simulink model "Simulation"  (R2016a)
(part 16 of 30)

C= [ thetadot4*(cos(theta5)*(((sin(theta6)*(cos(theta5)*(sin(theta4)*(thetadot2 + thetadot3) + thetadot1*cos(theta2 + theta3)*cos(theta4)) - sin(theta5)*(thetadot4 + thetadot1*sin(theta2 + theta3))))/10 + (cos(theta6)*(thetadot5 + cos(theta4)*(thetadot2 + thetadot3) - thetadot1*cos(theta2 + theta3)*sin(theta4)))/10)*(cos(theta2)*cos(theta6)*sin(theta3)*sin(theta5) - cos(theta2)*cos(theta3)*sin(theta4)*sin(theta6) + cos(theta3)*cos(theta6)*sin(theta2)*sin(theta5) + sin(theta2)*sin(theta3)*sin(theta4)*sin(theta6) - cos(theta2)*cos(theta3)*cos(theta4)*cos(theta5)*cos(theta6) + cos(theta4)*cos(theta5)*cos(theta6)*sin(theta2)*sin(theta3)) + ((sin(theta6)*(thetadot5 + cos(theta4)*(thetadot2 + thetadot3) - thetadot1*cos(theta2 + theta3)*sin(theta4)))/10 - (cos(theta6)*(cos(theta5)*(sin(theta4)*(thetadot2 + thetadot3) + thetadot1*cos(theta2 + theta3)*cos(theta4)) - sin(theta5)*(thetadot4 + thetadot1*sin(theta2 + theta3))))/10)*(cos(theta2)*cos(theta3)*cos(theta6)*sin(theta4) - cos(theta6)*sin(theta2)*sin(theta3)*sin(theta4) + cos(theta2)*sin(theta3)*sin(theta5)*sin(theta6) + cos(theta3)*sin(theta2)*sin(theta5)*sin(theta6) - cos(theta2)*cos(theta3)*cos(theta4)*cos(theta5)*sin(theta6) + cos(theta4)*cos(theta5)*sin(theta2)*sin(theta3)*sin(theta6))) + sin(theta5)*((thetadot5/10 + (cos(theta4)*(thetadot2 + thetadot3))/10 - (thetadot1*cos(theta2 + theta3)*sin(theta4))/10)*(cos(theta2)*cos(theta5)*sin(theta3) + cos(theta3)*cos(theta5)*sin(theta2) + cos(theta2)*cos(theta3)*cos(theta4)*sin(theta5) - cos(theta4)*sin(theta2)*sin(theta3)*sin(theta5)) - (thetadot6*sin(theta6)*(cos(theta2)*cos(theta6)*sin(theta3)*sin(theta5) - cos(theta2)*cos(theta3)*sin(theta4)*sin(theta6) + cos(theta3)*cos(theta6)*sin(theta2)*sin(theta5) + sin(theta2)*sin(theta3)*sin(theta4)*sin(theta6) - cos(theta2)*cos(theta3)*cos(theta4)*cos(theta5)*cos(theta6) + cos(theta4)*cos(theta5)*cos(theta6)*sin(theta2)*sin(theta3)))/10 + (2*thetadot6*cos(theta6)*((cos(theta2)*sin(theta4)*sin(theta5))/5 + (2*sin(theta2)*sin(theta3)*sin(theta4))/5 - (2*cos(theta2)*cos(theta3)*sin(theta4))/5 + (2*cos(theta2)*cos(theta3)*cos(theta6)*sin(theta4))/5 + (2*cos(theta2)*cos(theta3)*sin(theta4)*sin(theta5))/5 - (2*cos(theta6)*sin(theta2)*sin(theta3)*sin(theta4))/5 + (2*cos(theta2)*sin(theta3)*sin(theta5)*sin(theta6))/5 + (2*cos(theta3)*sin(theta2)*sin(theta5)*sin(theta6))/5 - (2*sin(theta2)*sin(theta3)*sin(theta4)*sin(theta5))/5 - (2*cos(theta2)*cos(theta3)*cos(theta4)*cos(theta5)*sin(theta6))/5 + (2*cos(theta4)*cos(theta5)*sin(theta2)*sin(theta3)*sin(theta6))/5))/5 + (thetadot6*cos(theta6)*(cos(theta2)*cos(theta3)*cos(theta6)*sin(theta4) - cos(theta6)*sin(theta2)*sin(theta3)*sin(theta4) + cos(theta2)*sin(theta3)*sin(theta5)*sin(theta6) + cos(theta3)*sin(theta2)*sin(theta5)*sin(theta6) - cos(theta2)*cos(theta3)*cos(theta4)*cos(theta5)*sin(theta6) + cos(theta4)*cos(theta5)*sin(theta2)*sin(theta3)*sin(theta6)))/10 + cos(theta2 + theta3)*sin(theta4)*((sin(theta5)*(sin(theta4)*(thetadot2 + thetadot3) + thetadot1*cos(theta2 + theta3)*cos(theta4)))/10 + (cos(theta5)*(thetadot4 + thetadot1*sin(theta2 + theta3)))/10)) + cos(theta5)*(((2*thetadot6)/5 + thetadot6*((2*cos(theta6))/5 - 2/5))*((cos(theta2)*cos(theta5)*cos(theta6)*sin(theta4))/5 - (2*cos(theta2)*cos(theta3)*cos(theta4)*sin(theta6))/5 - (cos(theta2)*cos(theta4)*sin(theta6))/5 + (2*cos(theta2)*cos(theta5)*sin(theta3)*sin(theta6))/5 + (2*cos(theta3)*cos(theta5)*sin(theta2)*sin(theta6))/5 + (2*cos(theta4)*sin(theta2)*sin(theta3)*sin(theta6))/5 + (2*cos(theta2)*cos(theta3)*cos(theta5)*cos(theta6)*sin(theta4))/5 + (2*cos(theta2)*cos(theta3)*cos(theta4)*sin(theta5)*sin(theta6))/5 - (2*cos(theta5)*cos(theta6)*sin(theta2)*sin(theta3)*sin(theta4))/5 - (2*cos(theta4)*sin(theta2)*sin(theta3)*sin(theta5)*sin(theta6))/5) - (thetadot5/10 + (cos(theta4)*(thetadot2 + thetadot3))/10 - (thetadot1*cos(theta2 + theta3)*sin(theta4))/10)*(cos(theta2)*sin(theta3)*sin(theta5) + cos(theta3)*sin(theta2)*sin(theta5) - cos(theta2)*cos(theta3)*cos(theta4)*cos(theta5) + cos(theta4)*cos(theta5)*sin(theta2)*sin(theta3)) + cos(theta2 + theta3)*sin(theta4)*((cos(theta5)*(sin(theta4)*(thetadot2 + thetadot3) + thetadot1*cos(theta2 + theta3)*cos(theta4)))/10 - (sin(theta5)*(thetadot4 + thetadot1*sin(theta2 + theta3)))/10) + (2*thetadot6*sin(theta6)*((cos(theta2)*cos(theta4)*cos(theta6))/5 + (2*cos(theta2)*cos(theta5)*sin(theta3))/5 + (2*cos(theta3)*cos(theta5)*sin(theta2))/5 + (2*cos(theta2)*cos(theta3)*cos(theta4)*cos(theta6))/5 + (2*cos(theta2)*cos(theta3)*cos(theta4)*sin(theta5))/5 - (2*cos(theta2)*cos(theta5)*cos(theta6)*sin(theta3))/5 - (2*cos(theta3)*cos(theta5)*cos(theta6)*sin(theta2))/5 - (2*cos(theta4)*cos(theta6)*sin(theta2)*sin(theta3))/5 + (cos(theta2)*cos(theta5)*sin(theta4)*sin(theta6))/5 - (2*cos(theta4)*sin(theta2)*sin(theta3)*sin(theta5))/5 - (2*cos(theta2)*cos(theta3)*cos(theta4)*cos(theta6)*sin(theta5))/5 + (2*cos(theta2)*cos(theta3)*cos(theta5)*sin(theta4)*sin(theta6))/5 + (2*cos(theta4)*cos(theta6)*sin(theta2)*sin(theta3)*sin(theta5))/5 - (2*cos(theta5)*sin(theta2)*sin(theta3)*sin(theta4)*sin(theta6))/5))/5) + sin(theta5)*sin(theta6)*((thetadot6/10 + (sin(theta5)*(sin(theta4)*(thetadot2 + thetadot3) + thetadot1*cos(theta2 + theta3)*cos(theta4)))/10 + (cos(theta5)*(thetadot4 + thetadot1*sin(theta2 + theta3)))/10)*(cos(theta2)*cos(theta6)*sin(theta3)*sin(theta5) - cos(theta2)*cos(theta3)*sin(theta4)*sin(theta6) + cos(theta3)*cos(theta6)*sin(theta2)*sin(theta5) + sin(theta2)*sin(theta3)*sin(theta4)*sin(theta6) - cos(theta2)*cos(theta3)*cos(theta4)*cos(theta5)*cos(theta6) + cos(theta4)*cos(theta5)*cos(theta6)*sin(theta2)*sin(theta3)) - ((sin(theta6)*(thetadot5 + cos(theta4)*(thetadot2 + thetadot3) - thetadot1*cos(theta2 + theta3)*sin(theta4)))/10 - (cos(theta6)*(cos(theta5)*(sin(theta4)*(thetadot2 + thetadot3) + thetadot1*cos(theta2 + theta3)*cos(theta4)) - sin(theta5)*(thetadot4 + thetadot1*sin(theta2 + theta3))))/10)*(cos(theta2)*cos(theta5)*sin(theta3) + cos(theta3)*cos(theta5)*sin(theta2) + cos(theta2)*cos(theta3)*cos(theta4)*sin(theta5) - cos(theta4)*sin(theta2)*sin(theta3)*sin(theta5))) + cos(theta2 + theta3)*cos(theta4)*((cos(theta4)*(thetadot2 + thetadot3))/10 - (thetadot1*cos(theta2 + theta3)*sin(theta4))/10) - cos(theta6)*sin(theta5)*((thetadot6/10 + (sin(theta5)*(sin(theta4)*(thetadot2 + thetadot3) + thetadot1*cos(theta2 + theta3)*cos(theta4)))/10 + (cos(theta5)*(thetadot4 + thetadot1*sin(theta2 + theta3)))/10)*(cos(theta2)*cos(theta3)*cos(theta6)*sin(theta4) - cos(theta6)*sin(theta2)*sin(theta3)*sin(theta4) + cos(theta2)*sin(theta3)*sin(theta5)*sin(theta6) + cos(theta3)*sin(theta2)*sin(theta5)*sin(theta6) - cos(theta2)*cos(theta3)*cos(theta4)*cos(theta5)*sin(theta6) + cos(theta4)*cos(theta5)*sin(theta2)*sin(theta3)*sin(theta6)) + ((sin(theta6)*(cos(theta5)*(sin(theta4)*(thetadot2 + thetadot3) + thetadot1*cos(theta2 + theta3)*cos(theta4)) - sin(theta5)*(thetadot4 + thetadot1*sin(theta2 + theta3))))/10 + (cos(theta6)*(thetadot5 + cos(theta4)*(thetadot2 + thetadot3) - thetadot1*cos(theta2 + theta3)*sin(theta4)))/10)*(cos(theta2)*cos(theta5)*sin(theta3) + cos(theta3)*cos(theta5)*sin(theta2) + cos(theta2)*cos(theta3)*cos(theta4)*sin(theta5) - cos(theta4)*sin(theta2)*sin(theta3)*sin(theta5))) + cos(theta2 + theta3)*sin(theta4)*((sin(theta4)*(thetadot2 + thetadot3))/10 + (thetadot1*cos(theta2 + theta3)*cos(theta4))/10) - (2*cos(theta5)*sin(theta6)*((thetadot6 + sin(theta5)*(sin(theta4)*(thetadot2 + thetadot3) + thetadot1*cos(theta2 + theta3)*cos(theta4)) + cos(theta5)*(thetadot4 + thetadot1*sin(theta2 + theta3)))*((cos(theta2)*cos(theta4)*cos(theta6))/5 + (2*cos(theta2)*cos(theta5)*sin(theta3))/5 + (2*cos(theta3)*cos(theta5)*sin(theta2))/5 + (2*cos(theta2)*cos(theta3)*cos(theta4)*cos(theta6))/5 + (2*cos(theta2)*cos(theta3)*cos(theta4)*sin(theta5))/5 - (2*cos(theta2)*cos(theta5)*cos(theta6)*sin(theta3))/5 - (2*cos(theta3)*cos(theta5)*cos(theta6)*sin(theta2))/5 - (2*cos(theta4)*cos(theta6)*sin(theta2)*sin(theta3))/5 + (cos(theta2)*cos(theta5)*sin(theta4)*sin(theta6))/5 - (2*cos(theta4)*sin(theta2)*sin(theta3)*sin(theta5))/5 - (2*cos(theta2)*cos(theta3)*cos(theta4)*cos(theta6)*sin(theta5))/5 + (2*cos(theta2)*cos(theta3)*cos(theta5)*sin(theta4)*sin(theta6))/5 + (2*cos(theta4)*cos(theta6)*sin(theta2)*sin(theta3)*sin(theta5))/5 - (2*cos(theta5)*sin(theta2)*sin(theta3)*sin(theta4)*sin(theta6))/5) - (cos(theta2)*cos(theta5)*sin(theta3) + cos(theta3)*cos(theta5)*sin(theta2) + cos(theta2)*cos(theta3)*cos(theta4)*sin(theta5) - cos(theta4)*sin(theta2)*sin(theta3)*sin(theta5))*((2*thetadot6)/5 - (sin(theta5)*(thetadot2*sin(theta4) + thetadot3*sin(theta4) + thetadot1*cos(theta2 + theta3)*cos(theta4)) + cos(theta5)*(thetadot4 + thetadot1*sin(theta2 + theta3)))*((2*cos(theta6))/5 - 2/5) - (sin(theta6)*(2*thetadot2*cos(theta4)*cos(theta5) + 2*thetadot3*cos(theta4)*cos(theta5) - thetadot2*sin(theta3)*sin(theta5) + thetadot2*cos(theta3)*cos(theta4)*cos(theta5) - thetadot1*cos(theta2)*cos(theta5)*sin(theta4) - 2*thetadot1*cos(theta2)*cos(theta3)*cos(theta5)*sin(theta4) + 2*thetadot1*cos(theta5)*sin(theta2)*sin(theta3)*sin(theta4)))/5 + (cos(theta6)*(2*thetadot2*sin(theta4) + 2*thetadot3*sin(theta4) + thetadot1*cos(theta2)*cos(theta4) + thetadot2*cos(theta3)*sin(theta4) + 2*thetadot1*cos(theta2)*cos(theta3)*cos(theta4) - 2*thetadot1*cos(theta4)*sin(theta2)*sin(theta3)))/5) - (sin(theta6)*(cos(theta5)*(sin(theta4)*(thetadot2 + thetadot3) + thetadot1*cos(theta2 + theta3)*cos(theta4)) - sin(theta5)*(thetadot4 + thetadot1*sin(theta2 + theta3))) + cos(theta6)*(thetadot5 + cos(theta4)*(thetadot2 + thetadot3) - thetadot1*cos(theta2 + theta3)*sin(theta4)))*((cos(theta2)*sin(theta4)*sin(theta5))/5 + (2*sin(theta2)*sin(theta3)*sin(theta4))/5 - (2*cos(theta2)*cos(theta3)*sin(theta4))/5 + (2*cos(theta2)*cos(theta3)*cos(theta6)*sin(theta4))/5 + (2*cos(theta2)*cos(theta3)*sin(theta4)*sin(theta5))/5 - (2*cos(theta6)*sin(theta2)*sin(theta3)*sin(theta4))/5 + (2*cos(theta2)*sin(theta3)*sin(theta5)*sin(theta6))/5 + (2*cos(theta3)*sin(theta2)*sin(theta5)*sin(theta6))/5 - (2*sin(theta2)*sin(theta3)*sin(theta4)*sin(theta5))/5 - (2*cos(theta2)*cos(theta3)*cos(theta4)*cos(theta5)*sin(theta6))/5 + (2*cos(theta4)*cos(theta5)*sin(theta2)*sin(theta3)*sin(theta6))/5) + ((sin(theta5)*(thetadot2*cos(theta4) + thetadot3*cos(theta4) - thetadot1*cos(theta2 + theta3)*sin(theta4)))/5 + sin(theta5)*((thetadot2*cos(theta4))/5 + (thetadot3*cos(theta4))/5 - (thetadot1*cos(theta2 + theta3)*sin(theta4))/5 + (thetadot2*cos(theta3)*cos(theta4))/5 - (thetadot1*cos(theta2)*sin(theta4))/5) + ((2*cos(theta6))/5 - 2/5)*(thetadot5 + thetadot2*cos(theta4) + thetadot3*cos(theta4) - thetadot1*cos(theta2 + theta3)*sin(theta4)) + (2*sin(theta6)*(cos(theta5)*(thetadot2*sin(theta4) + thetadot3*sin(theta4) + thetadot1*cos(theta2 + theta3)*cos(theta4)) - sin(theta5)*(thetadot4 + thetadot1*sin(theta2 + theta3))))/5 + (thetadot2*cos(theta5)*sin(theta3))/5)*(cos(theta2)*cos(theta3)*cos(theta6)*sin(theta4) - cos(theta6)*sin(theta2)*sin(theta3)*sin(theta4) + cos(theta2)*sin(theta3)*sin(theta5)*sin(theta6) + cos(theta3)*sin(theta2)*sin(theta5)*sin(theta6) - cos(theta2)*cos(theta3)*cos(theta4)*cos(theta5)*sin(theta6) + cos(theta4)*cos(theta5)*sin(theta2)*sin(theta3)*sin(theta6))))/5 - (2*cos(theta5)*(cos(theta6) - 1)*(((sin(theta6)*(2*thetadot2*sin(theta4) + 2*thetadot3*sin(theta4) + thetadot1*cos(theta2)*cos(theta4) + thetadot2*cos(theta3)*sin(theta4) + 2*thetadot1*cos(theta2)*cos(theta3)*cos(theta4) - 2*thetadot1*cos(theta4)*sin(theta2)*sin(theta3)))/5 + (cos(theta6)*(2*thetadot2*cos(theta4)*cos(theta5) + 2*thetadot3*cos(theta4)*cos(theta5) - thetadot2*sin(theta3)*sin(theta5) + thetadot2*cos(theta3)*cos(theta4)*cos(theta5) - thetadot1*cos(theta2)*cos(theta5)*sin(theta4) - 2*thetadot1*cos(theta2)*cos(theta3)*cos(theta5)*sin(theta4) + 2*thetadot1*cos(theta5)*sin(theta2)*sin(theta3)*sin(theta4)))/5 - (2*sin(theta6)*(sin(theta5)*(thetadot2*sin(theta4) + thetadot3*sin(theta4) + thetadot1*cos(theta2 + theta3)*cos(theta4)) + cos(theta5)*(thetadot4 + thetadot1*sin(theta2 + theta3))))/5)*(cos(theta2)*cos(theta5)*sin(theta3) + cos(theta3)*cos(theta5)*sin(theta2) + cos(theta2)*cos(theta3)*cos(theta4)*sin(theta5) - cos(theta4)*sin(theta2)*sin(theta3)*sin(theta5)) + ((sin(theta5)*(thetadot2*cos(theta4) + thetadot3*cos(theta4) - thetadot1*cos(theta2 + theta3)*sin(theta4)))/5 + sin(theta5)*((thetadot2*cos(theta4))/5 + (thetadot3*cos(theta4))/5 - (thetadot1*cos(theta2 + theta3)*sin(theta4))/5 + (thetadot2*cos(theta3)*cos(theta4))/5 - (thetadot1*cos(theta2)*sin(theta4))/5) + ((2*cos(theta6))/5 - 2/5)*(thetadot5 + thetadot2*cos(theta4) + thetadot3*cos(theta4) - thetadot1*cos(theta2 + theta3)*sin(theta4)) + (2*sin(theta6)*(cos(theta5)*(thetadot2*sin(theta4) + thetadot3*sin(theta4) + thetadot1*cos(theta2 + theta3)*cos(theta4)) - sin(theta5)*(thetadot4 + thetadot1*sin(theta2 + theta3))))/5 + (thetadot2*cos(theta5)*sin(theta3))/5)*(cos(theta2)*cos(theta6)*sin(theta3)*sin(theta5) - cos(theta2)*cos(theta3)*sin(theta4)*sin(theta6) + cos(theta3)*cos(theta6)*sin(theta2)*sin(theta5) + sin(theta2)*sin(theta3)*sin(theta4)*sin(theta6) - cos(theta2)*cos(theta3)*cos(theta4)*cos(theta5)*cos(theta6) + cos(theta4)*cos(theta5)*cos(theta6)*sin(theta2)*sin(theta3)) + (sin(theta6)*(thetadot5 + cos(theta4)*(thetadot2 + thetadot3) - thetadot1*cos(theta2 + theta3)*sin(theta4)) - cos(theta6)*(cos(theta5)*(sin(theta4)*(thetadot2 + thetadot3) + thetadot1*cos(theta2 + theta3)*cos(theta4)) - sin(theta5)*(thetadot4 + thetadot1*sin(theta2 + theta3))))*((cos(theta2)*sin(theta4)*sin(theta5))/5 + (2*sin(theta2)*sin(theta3)*sin(theta4))/5 - (2*cos(theta2)*cos(theta3)*sin(theta4))/5 + (2*cos(theta2)*cos(theta3)*cos(theta6)*sin(theta4))/5 + (2*cos(theta2)*cos(theta3)*sin(theta4)*sin(theta5))/5 - (2*cos(theta6)*sin(theta2)*sin(theta3)*sin(theta4))/5 + (2*cos(theta2)*sin(theta3)*sin(theta5)*sin(theta6))/5 + (2*cos(theta3)*sin(theta2)*sin(theta5)*sin(theta6))/5 - (2*sin(theta2)*sin(theta3)*sin(theta4)*sin(theta5))/5 - (2*cos(theta2)*cos(theta3)*cos(theta4)*cos(theta5)*sin(theta6))/5 + (2*cos(theta4)*cos(theta5)*sin(theta2)*sin(theta3)*sin(theta6))/5) + (thetadot6 + sin(theta5)*(sin(theta4)*(thetadot2 + thetadot3) + thetadot1*cos(theta2 + theta3)*cos(theta4)) + cos(theta5)*(thetadot4 + thetadot1*sin(theta2 + theta3)))*((cos(theta2)*cos(theta5)*cos(theta6)*sin(theta4))/5 - (2*cos(theta2)*cos(theta3)*cos(theta4)*sin(theta6))/5 - (cos(theta2)*cos(theta4)*sin(theta6))/5 + (2*cos(theta2)*cos(theta5)*sin(theta3)*sin(theta6))/5 + (2*cos(theta3)*cos(theta5)*sin(theta2)*sin(theta6))/5 + (2*cos(theta4)*sin(theta2)*sin(theta3)*sin(theta6))/5 + (2*cos(theta2)*cos(theta3)*cos(theta5)*cos(theta6)*sin(theta4))/5 + (2*cos(theta2)*cos(theta3)*cos(theta4)*sin(theta5)*sin(theta6))/5 - (2*cos(theta5)*cos(theta6)*sin(theta2)*sin(theta3)*sin(theta4))/5 - (2*cos(theta4)*sin(theta2)*sin(theta3)*sin(theta5)*sin(theta6))/5)))/5 + (thetadot5*cos(theta5)*(cos(theta2)*sin(theta3)*sin(theta5) + cos(theta3)*sin(theta2)*sin(theta5) - cos(theta2)*cos(theta3)*cos(theta4)*cos(theta5) + cos(theta4)*cos(theta5)*sin(theta2)*sin(theta3)))/10 - (2*sin(theta5)*sin(theta6)*((sin(theta6)*(cos(theta5)*(sin(theta4)*(thetadot2 + thetadot3) + thetadot1*cos(theta2 + theta3)*cos(theta4)) - sin(theta5)*(thetadot4 + thetadot1*sin(theta2 + theta3))) + cos(theta6)*(thetadot5 + cos(theta4)*(thetadot2 + thetadot3) - thetadot1*cos(theta2 + theta3)*sin(theta4)))*((cos(theta2)*cos(theta5)*cos(theta6)*sin(theta4))/5 - (2*cos(theta2)*cos(theta3)*cos(theta4)*sin(theta6))/5 - (cos(theta2)*cos(theta4)*sin(theta6))/5 + (2*cos(theta2)*cos(theta5)*sin(theta3)*sin(theta6))/5 + (2*cos(theta3)*cos(theta5)*sin(theta2)*sin(theta6))/5 + (2*cos(theta4)*sin(theta2)*sin(theta3)*sin(theta6))/5 + (2*cos(theta2)*cos(theta3)*cos(theta5)*cos(theta6)*sin(theta4))/5 + (2*cos(theta2)*cos(theta3)*cos(theta4)*sin(theta5)*sin(theta6))/5 - (2*cos(theta5)*cos(theta6)*sin(theta2)*sin(theta3)*sin(theta4))/5 - (2*cos(theta4)*sin(theta2)*sin(theta3)*sin(theta5)*sin(theta6))/5) + (sin(theta6)*(thetadot5 + cos(theta4)*(thetadot2 + thetadot3) - thetadot1*cos(theta2 + theta3)*sin(theta4)) - cos(theta6)*(cos(theta5)*(sin(theta4)*(thetadot2 + thetadot3) + thetadot1*cos(theta2 + theta3)*cos(theta4)) - sin(theta5)*(thetadot4 + thetadot1*sin(theta2 + theta3))))*((cos(theta2)*cos(theta4)*cos(theta6))/5 + (2*cos(theta2)*cos(theta5)*sin(theta3))/5 + (2*cos(theta3)*cos(theta5)*sin(theta2))/5 + (2*cos(theta2)*cos(theta3)*cos(theta4)*cos(theta6))/5 + (2*cos(theta2)*cos(theta3)*cos(theta4)*sin(theta5))/5 - (2*cos(theta2)*cos(theta5)*cos(theta6)*sin(theta3))/5 - (2*cos(theta3)*cos(theta5)*cos(theta6)*sin(theta2))/5 - (2*cos(theta4)*cos(theta6)*sin(theta2)*sin(theta3))/5 + (cos(theta2)*cos(theta5)*sin(theta4)*sin(theta6))/5 - (2*cos(theta4)*sin(theta2)*sin(theta3)*sin(theta5))/5 - (2*cos(theta2)*cos(theta3)*cos(theta4)*cos(theta6)*sin(theta5))/5 + (2*cos(theta2)*cos(theta3)*cos(theta5)*sin(theta4)*sin(theta6))/5 + (2*cos(theta4)*cos(theta6)*sin(theta2)*sin(theta3)*sin(theta5))/5 - (2*cos(theta5)*sin(theta2)*sin(theta3)*sin(theta4)*sin(theta6))/5) - ((sin(theta6)*(2*thetadot2*sin(theta4) + 2*thetadot3*sin(theta4) + thetadot1*cos(theta2)*cos(theta4) + thetadot2*cos(theta3)*sin(theta4) + 2*thetadot1*cos(theta2)*cos(theta3)*cos(theta4) - 2*thetadot1*cos(theta4)*sin(theta2)*sin(theta3)))/5 + (cos(theta6)*(2*thetadot2*cos(theta4)*cos(theta5) + 2*thetadot3*cos(theta4)*cos(theta5) - thetadot2*sin(theta3)*sin(theta5) + thetadot2*cos(theta3)*cos(theta4)*cos(theta5) - thetadot1*cos(theta2)*cos(theta5)*sin(theta4) - 2*thetadot1*cos(theta2)*cos(theta3)*cos(theta5)*sin(theta4) + 2*thetadot1*cos(theta5)*sin(theta2)*sin(theta3)*sin(theta4)))/5 - (2*sin(theta6)*(sin(theta5)*(thetadot2*sin(theta4) + thetadot3*sin(theta4) + thetadot1*cos(theta2 + theta3)*cos(theta4)) + cos(theta5)*(thetadot4 + thetadot1*sin(theta2 + theta3))))/5)*(cos(theta2)*cos(theta3)*cos(theta6)*sin(theta4) - cos(theta6)*sin(theta2)*sin(theta3)*sin(theta4) + cos(theta2)*sin(theta3)*sin(theta5)*sin(theta6) + cos(theta3)*sin(theta2)*sin(theta5)*sin(theta6) - cos(theta2)*cos(theta3)*cos(theta4)*cos(theta5)*sin(theta6) + cos(theta4)*cos(theta5)*sin(theta2)*sin(theta3)*sin(theta6)) - ((2*thetadot6)/5 - (sin(theta5)*(thetadot2*sin(theta4) + thetadot3*sin(theta4) + thetadot1*cos(theta2 + theta3)*cos(theta4)) + cos(theta5)*(thetadot4 + thetadot1*sin(theta2 + theta3)))*((2*cos(theta6))/5 - 2/5) - (sin(theta6)*(2*thetadot2*cos(theta4)*cos(theta5) + 2*thetadot3*cos(theta4)*cos(theta5) - thetadot2*sin(theta3)*sin(theta5) + thetadot2*cos(theta3)*cos(theta4)*cos(theta5) - thetadot1*cos(theta2)*cos(theta5)*sin(theta4) - 2*thetadot1*cos(theta2)*cos(theta3)*cos(theta5)*sin(theta4) + 2*thetadot1*cos(theta5)*sin(theta2)*sin(theta3)*sin(theta4)))/5 + (cos(theta6)*(2*thetadot2*sin(theta4) + 2*thetadot3*sin(theta4) + thetadot1*cos(theta2)*cos(theta4) + thetadot2*cos(theta3)*sin(theta4) + 2*thetadot1*cos(theta2)*cos(theta3)*cos(theta4) - 2*thetadot1*cos(theta4)*sin(theta2)*sin(theta3)))/5)*(cos(theta2)*cos(theta6)*sin(theta3)*sin(theta5) - cos(theta2)*cos(theta3)*sin(theta4)*sin(theta6) + cos(theta3)*cos(theta6)*sin(theta2)*sin(theta5) + sin(theta2)*sin(theta3)*sin(theta4)*sin(theta6) - cos(theta2)*cos(theta3)*cos(theta4)*cos(theta5)*cos(theta6) + cos(theta4)*cos(theta5)*cos(theta6)*sin(theta2)*sin(theta3))))/5 - (thetadot5*sin(theta5)*(cos(theta2)*cos(theta5)*sin(theta3) + cos(theta3)*cos(theta5)*sin(theta2) + cos(theta2)*cos(theta3)*cos(theta4)*sin(theta5) - cos(theta4)*sin(theta2)*sin(theta3)*sin(theta5)))/5 - (2*thetadot5*sin(theta5)*sin(theta6)*((cos(theta2)*cos(theta5)*cos(theta6)*sin(theta4))/5 - (2*cos(theta2)*cos(theta3)*cos(theta4)*sin(theta6))/5 - (cos(theta2)*cos(theta4)*sin(theta6))/5 + (2*cos(theta2)*cos(theta5)*sin(theta3)*sin(theta6))/5 + (2*cos(theta3)*cos(theta5)*sin(theta2)*sin(theta6))/5 + (2*cos(theta4)*sin(theta2)*sin(theta3)*sin(theta6))/5 + (2*cos(theta2)*cos(theta3)*cos(theta5)*cos(theta6)*sin(theta4))/5 + (2*cos(theta2)*cos(theta3)*cos(theta4)*sin(theta5)*sin(theta6))/5 - (2*cos(theta5)*cos(theta6)*sin(theta2)*sin(theta3)*sin(theta4))/5 - (2*cos(theta4)*sin(theta2)*sin(theta3)*sin(theta5)*sin(theta6))/5))/5 + thetadot5*sin(theta5)*((2*cos(theta6))/5 - 2/5)*((cos(theta2)*cos(theta4)*cos(theta6))/5 + (2*cos(theta2)*cos(theta5)*sin(theta3))/5 + (2*cos(theta3)*cos(theta5)*sin(theta2))/5 + (2*cos(theta2)*cos(theta3)*cos(theta4)*cos(theta6))/5 + (2*cos(theta2)*cos(theta3)*cos(theta4)*sin(theta5))/5 - (2*cos(theta2)*cos(theta5)*cos(theta6)*sin(theta3))/5 - (2*cos(theta3)*cos(theta5)*cos(theta6)*sin(theta2))/5 - (2*cos(theta4)*cos(theta6)*sin(theta2)*sin(theta3))/5 + (cos(theta2)*cos(theta5)*sin(theta4)*sin(theta6))/5 - (2*cos(theta4)*sin(theta2)*sin(theta3)*sin(theta5))/5 - (2*cos(theta2)*cos(theta3)*cos(theta4)*cos(theta6)*sin(theta5))/5 + (2*cos(theta2)*cos(theta3)*cos(theta5)*sin(theta4)*sin(theta6))/5 + (2*cos(theta4)*cos(theta6)*sin(theta2)*sin(theta3)*sin(theta5))/5 - (2*cos(theta5)*sin(theta2)*sin(theta3)*sin(theta4)*sin(theta6))/5) + (thetadot5*cos(theta5)*cos(theta6)*(cos(theta2)*cos(theta6)*sin(theta3)*sin(theta5) - cos(theta2)*cos(theta3)*sin(theta4)*sin(theta6) + cos(theta3)*cos(theta6)*sin(theta2)*sin(theta5) + sin(theta2)*sin(theta3)*sin(theta4)*sin(theta6) - cos(theta2)*cos(theta3)*cos(theta4)*cos(theta5)*cos(theta6) + cos(theta4)*cos(theta5)*cos(theta6)*sin(theta2)*sin(theta3)))/10 + (2*thetadot5*cos(theta5)*sin(theta6)*((cos(theta2)*sin(theta4)*sin(theta5))/5 + (2*sin(theta2)*sin(theta3)*sin(theta4))/5 - (2*cos(theta2)*cos(theta3)*sin(theta4))/5 + (2*cos(theta2)*cos(theta3)*cos(theta6)*sin(theta4))/5 + (2*cos(theta2)*cos(theta3)*sin(theta4)*sin(theta5))/5 - (2*cos(theta6)*sin(theta2)*sin(theta3)*sin(theta4))/5 + (2*cos(theta2)*sin(theta3)*sin(theta5)*sin(theta6))/5 + (2*cos(theta3)*sin(theta2)*sin(theta5)*sin(theta6))/5 - (2*sin(theta2)*sin(theta3)*sin(theta4)*sin(theta5))/5 - (2*cos(theta2)*cos(theta3)*cos(theta4)*cos(theta5)*sin(theta6))/5 + (2*cos(theta4)*cos(theta5)*sin(theta2)*sin(theta3)*sin(theta6))/5))/5 + (thetadot5*cos(theta5)*sin(theta6)*(cos(theta2)*cos(theta3)*cos(theta6)*sin(theta4) - cos(theta6)*sin(theta2)*sin(theta3)*sin(theta4) + cos(theta2)*sin(theta3)*sin(theta5)*sin(theta6) + cos(theta3)*sin(theta2)*sin(theta5)*sin(theta6) - cos(theta2)*cos(theta3)*cos(theta4)*cos(theta5)*sin(theta6) + cos(theta4)*cos(theta5)*sin(theta2)*sin(theta3)*sin(theta6)))/10) - thetadot1*(((thetadot6 + sin(theta5)*(sin(theta4)*(thetadot2 + thetadot3) + thetadot1*cos(theta2 + theta3)*cos(theta4)) + cos(theta5)*(thetadot4 + thetadot1*sin(theta2 + theta3)))*((cos(theta2)*cos(theta4)*cos(theta6))/5 + (2*cos(theta2)*cos(theta5)*sin(theta3))/5 + (2*cos(theta3)*cos(theta5)*sin(theta2))/5 + (2*cos(theta2)*cos(theta3)*cos(theta4)*cos(theta6))/5 + (2*cos(theta2)*cos(theta3)*cos(theta4)*sin(theta5))/5 - (2*cos(theta2)*cos(theta5)*cos(theta6)*sin(theta3))/5 - (2*cos(theta3)*cos(theta5)*cos(theta6)*sin(theta2))/5 - (2*cos(theta4)*cos(theta6)*sin(theta2)*sin(theta3))/5 + (cos(theta2)*cos(theta5)*sin(theta4)*sin(theta6))/5 - (2*cos(theta4)*sin(theta2)*sin(theta3)*sin(theta5))/5 - (2*cos(theta2)*cos(theta3)*cos(theta4)*cos(theta6)*sin(theta5))/5 + (2*cos(theta2)*cos(theta3)*cos(theta5)*sin(theta4)*sin(theta6))/5 + (2*cos(theta4)*cos(theta6)*sin(theta2)*sin(theta3)*sin(theta5))/5 - (2*cos(theta5)*sin(theta2)*sin(theta3)*sin(theta4)*sin(theta6))/5) - (cos(theta2)*cos(theta5)*sin(theta3) + cos(theta3)*cos(theta5)*sin(theta2) + cos(theta2)*cos(theta3)*cos(theta4)*sin(theta5) - cos(theta4)*sin(theta2)*sin(theta3)*sin(theta5))*((2*thetadot6)/5 - (sin(theta5)*(thetadot2*sin(theta4) + thetadot3*sin(theta4) + thetadot1*cos(theta2 + theta3)*cos(theta4)) + cos(theta5)*(thetadot4 + thetadot1*sin(theta2 + theta3)))*((2*cos(theta6))/5 - 2/5) - (sin(theta6)*(2*thetadot2*cos(theta4)*cos(theta5) + 2*thetadot3*cos(theta4)*cos(theta5) - thetadot2*sin(theta3)*sin(theta5) + thetadot2*cos(theta3)*cos(theta4)*cos(theta5) - thetadot1*cos(theta2)*cos(theta5)*sin(theta4) - 2*thetadot1*cos(theta2)*cos(theta3)*cos(theta5)*sin(theta4) + 2*thetadot1*cos(theta5)*sin(theta2)*sin(theta3)*sin(theta4)))/5 + (cos(theta6)*(2*thetadot2*sin(theta4) + 2*thetadot3*sin(theta4) + thetadot1*cos(theta2)*cos(theta4) + thetadot2*cos(theta3)*sin(theta4) + 2*thetadot1*cos(theta2)*cos(theta3)*cos(theta4) - 2*thetadot1*cos(theta4)*sin(theta2)*sin(theta3)))/5) - (sin(theta6)*(cos(theta5)*(sin(theta4)*(thetadot2 + thetadot3) + thetadot1*cos(theta2 + theta3)*cos(theta4)) - sin(theta5)*(thetadot4 + thetadot1*sin(theta2 + theta3))) + cos(theta6)*(thetadot5 + cos(theta4)*(thetadot2 + thetadot3) - thetadot1*cos(theta2 + theta3)*sin(theta4)))*((cos(theta2)*sin(theta4)*sin(theta5))/5 + (2*sin(theta2)*sin(theta3)*sin(theta4))/5 - (2*cos(theta2)*cos(theta3)*sin(theta4))/5 + (2*cos(theta2)*cos(theta3)*cos(theta6)*sin(theta4))/5 + (2*cos(theta2)*cos(theta3)*sin(theta4)*sin(theta5))/5 - (2*cos(theta6)*sin(theta2)*sin(theta3)*sin(theta4))/5 + (2*cos(theta2)*sin(theta3)*sin(theta5)*sin(theta6))/5 + (2*cos(theta3)*sin(theta2)*sin(theta5)*sin(theta6))/5 - (2*sin(theta2)*sin(theta3)*sin(theta4)*sin(theta5))/5 - (2*cos(theta2)*cos(theta3)*cos(theta4)*cos(theta5)*sin(theta6))/5 + (2*cos(theta4)*cos(theta5)*sin(theta2)*sin(theta3)*sin(theta6))/5) + ((sin(theta5)*(thetadot2*cos(theta4) + thetadot3*cos(theta4) - thetadot1*cos(theta2 + theta3)*sin(theta4)))/5 + sin(theta5)*((thetadot2*cos(theta4))/5 + (thetadot3*cos(theta4))/5 - (thetadot1*cos(theta2 + theta3)*sin(theta4))/5 + (thetadot2*cos(theta3)*cos(theta4))/5 - (thetadot1*cos(theta2)*sin(theta4))/5) + ((2*cos(theta6))/5 - 2/5)*(thetadot5 + thetadot2*cos(theta4) + thetadot3*cos(theta4) - thetadot1*cos(theta2 + theta3)*sin(theta4)) + (2*sin(theta6)*(cos(theta5)*(thetadot2*sin(theta4) + thetadot3*sin(theta4) + thetadot1*cos(theta2 + theta3)*cos(theta4)) - sin(theta5)*(thetadot4 + thetadot1*sin(theta2 + theta3))))/5 + (thetadot2*cos(theta5)*sin(theta3))/5)*(cos(theta2)*cos(theta3)*cos(theta6)*sin(theta4) - cos(theta6)*sin(theta2)*sin(theta3)*sin(theta4) + cos(theta2)*sin(theta3)*sin(theta5)*sin(theta6) + cos(theta3)*sin(theta2)*sin(theta5)*sin(theta6) - cos(theta2)*cos(theta3)*cos(theta4)*cos(theta5)*sin(theta6) + cos(theta4)*cos(theta5)*sin(theta2)*sin(theta3)*sin(theta6)))*((cos(theta2)*cos(theta5)*cos(theta6)*sin(theta4))/5 - (2*cos(theta2)*cos(theta3)*cos(theta4)*sin(theta6))/5 - (cos(theta2)*cos(theta4)*sin(theta6))/5 + (2*cos(theta2)*cos(theta5)*sin(theta3)*sin(theta6))/5 + (2*cos(theta3)*cos(theta5)*sin(theta2)*sin(theta6))/5 + (2*cos(theta4)*sin(theta2)*sin(theta3)*sin(theta6))/5 + (2*cos(theta2)*cos(theta3)*cos(theta5)*cos(theta6)*sin(theta4))/5 + (2*cos(theta2)*cos(theta3)*cos(theta4)*sin(theta5)*sin(theta6))/5 - (2*cos(theta5)*cos(theta6)*sin(theta2)*sin(theta3)*sin(theta4))/5 - (2*cos(theta4)*sin(theta2)*sin(theta3)*sin(theta5)*sin(theta6))/5) - cos(theta2 + theta3)*(((thetadot4*cos(theta4)*cos(theta6))/10 + (thetadot4*cos(theta5)*sin(theta4)*sin(theta6))/10)*(cos(theta2)*cos(theta3)*cos(theta6)*sin(theta4) - cos(theta6)*sin(theta2)*sin(theta3)*sin(theta4) + cos(theta2)*sin(theta3)*sin(theta5)*sin(theta6) + cos(theta3)*sin(theta2)*sin(theta5)*sin(theta6) - cos(theta2)*cos(theta3)*cos(theta4)*cos(theta5)*sin(theta6) + cos(theta4)*cos(theta5)*sin(theta2)*sin(theta3)*sin(theta6)) - sin(theta2 + theta3)*(thetadot2/10 + thetadot3/10) - ((thetadot4*cos(theta4)*sin(theta6))/10 - (thetadot4*cos(theta5)*cos(theta6)*sin(theta4))/10)*(cos(theta2)*cos(theta6)*sin(theta3)*sin(theta5) - cos(theta2)*cos(theta3)*sin(theta4)*sin(theta6) + cos(theta3)*cos(theta6)*sin(theta2)*sin(theta5) + sin(theta2)*sin(theta3)*sin(theta4)*sin(theta6) - cos(theta2)*cos(theta3)*cos(theta4)*cos(theta5)*cos(theta6) + cos(theta4)*cos(theta5)*cos(theta6)*sin(theta2)*sin(theta3)) - ((thetadot4*cos(theta6)*sin(theta4))/5 + thetadot4*sin(theta4)*(cos(theta6)/5 + (2*sin(theta5))/5 - (2*cos(theta6)*sin(theta5))/5) - (2*thetadot4*cos(theta4)*cos(theta5)*sin(theta6))/5)*((cos(theta2)*cos(theta4)*cos(theta6))/5 + (2*cos(theta2)*cos(theta5)*sin(theta3))/5 + (2*cos(theta3)*cos(theta5)*sin(theta2))/5 + (2*cos(theta2)*cos(theta3)*cos(theta4)*cos(theta6))/5 + (2*cos(theta2)*cos(theta3)*cos(theta4)*sin(theta5))/5 - (2*cos(theta2)*cos(theta5)*cos(theta6)*sin(theta3))/5 - (2*cos(theta3)*cos(theta5)*cos(theta6)*sin(theta2))/5 - (2*cos(theta4)*cos(theta6)*sin(theta2)*sin(theta3))/5 + (cos(theta2)*cos(theta5)*sin(theta4)*sin(theta6))/5 - (2*cos(theta4)*sin(theta2)*sin(theta3)*sin(theta5))/5 - (2*cos(theta2)*cos(theta3)*cos(theta4)*cos(theta6)*sin(theta5))/5 + (2*cos(theta2)*cos(theta3)*cos(theta5)*sin(theta4)*sin(theta6))/5 + (2*cos(theta4)*cos(theta6)*sin(theta2)*sin(theta3)*sin(theta5))/5 - (2*cos(theta5)*sin(theta2)*sin(theta3)*sin(theta4)*sin(theta6))/5) + ((thetadot4*sin(theta4)*sin(theta6))/5 - (thetadot4*sin(theta4)*sin(theta6)*(2*sin(theta5) - 1))/5 + (2*thetadot4*cos(theta4)*cos(theta5)*cos(theta6))/5)*((cos(theta2)*cos(theta5)*cos(theta6)*sin(theta4))/5 - (2*cos(theta2)*cos(theta3)*cos(theta4)*sin(theta6))/5 - (cos(theta2)*cos(theta4)*sin(theta6))/5 + (2*cos(theta2)*cos(theta5)*sin(theta3)*sin(theta6))/5 + (2*cos(theta3)*cos(theta5)*sin(theta2)*sin(theta6))/5 + (2*cos(theta4)*sin(theta2)*sin(theta3)*sin(theta6))/5 + (2*cos(theta2)*cos(theta3)*cos(theta5)*cos(theta6)*sin(theta4))/5 + (2*cos(theta2)*cos(theta3)*cos(theta4)*sin(theta5)*sin(theta6))/5 - (2*cos(theta5)*cos(theta6)*sin(theta2)*sin(theta3)*sin(theta4))/5 - (2*cos(theta4)*sin(theta2)*sin(theta3)*sin(theta5)*sin(theta6))/5) + (thetadot4*cos(theta4)*((2*cos(theta6))/5 + sin(theta5)/5 - 2/5) + (thetadot4*cos(theta4)*sin(theta5))/5 + (2*thetadot4*cos(theta5)*sin(theta4)*sin(theta6))/5)*((cos(theta2)*sin(theta4)*sin(theta5))/5 + (2*sin(theta2)*sin(theta3)*sin(theta4))/5 - (2*cos(theta2)*cos(theta3)*sin(theta4))/5 + (2*cos(theta2)*cos(theta3)*cos(theta6)*sin(theta4))/5 + (2*cos(theta2)*cos(theta3)*sin(theta4)*sin(theta5))/5 - (2*cos(theta6)*sin(theta2)*sin(theta3)*sin(theta4))/5 + (2*cos(theta2)*sin(theta3)*sin(theta5)*sin(theta6))/5 + (2*cos(theta3)*sin(theta2)*sin(theta5)*sin(theta6))/5 - (2*sin(theta2)*sin(theta3)*sin(theta4)*sin(theta5))/5 - (2*cos(theta2)*cos(theta3)*cos(theta4)*cos(theta5)*sin(theta6))/5 + (2*cos(theta4)*cos(theta5)*sin(theta2)*sin(theta3)*sin(theta6))/5) + (thetadot4*cos(theta2 + theta3)*cos(theta4)*sin(theta4))/10 + (thetadot4*cos(theta5)*sin(theta4)*(cos(theta2)*sin(theta3)*sin(theta5) + cos(theta3)*sin(theta2)*sin(theta5) - cos(theta2)*cos(theta3)*cos(theta4)*cos(theta5) + cos(theta4)*cos(theta5)*sin(theta2)*sin(theta3)))/10 - (thetadot4*sin(theta4)*sin(theta5)*(cos(theta2)*cos(theta5)*sin(theta3) + cos(theta3)*cos(theta5)*sin(theta2) + cos(theta2)*cos(theta3)*cos(theta4)*sin(theta5) - cos(theta4)*sin(theta2)*sin(theta3)*sin(theta5)))/5 - (2*thetadot4*cos(theta4)*sin(theta4)*(2*cos(theta2 + theta3) + cos(theta2)))/25 + (2*thetadot4*cos(theta4)*cos(theta5)^2*sin(theta4)*(2*cos(theta2 + theta3) + cos(theta2)))/25 + (2*thetadot4*cos(theta4)*sin(theta4)*sin(theta5)^2*(2*cos(theta2 + theta3) + cos(theta2)))/25) - (thetadot2*cos(theta2)*((cos(theta3)*sin(theta5)*sin(theta6))/10 - (cos(theta6)*sin(theta3)*sin(theta4))/10 + (cos(theta4)*cos(theta5)*sin(theta3)*sin(theta6))/10) - thetadot2*sin(theta2)*((sin(theta3)*sin(theta5)*sin(theta6))/10 + (cos(theta3)*cos(theta6)*sin(theta4))/10 - (cos(theta3)*cos(theta4)*cos(theta5)*sin(theta6))/10))*(cos(theta2)*cos(theta3)*cos(theta6)*sin(theta4) - cos(theta6)*sin(theta2)*sin(theta3)*sin(theta4) + cos(theta2)*sin(theta3)*sin(theta5)*sin(theta6) + cos(theta3)*sin(theta2)*sin(theta5)*sin(theta6) - cos(theta2)*cos(theta3)*cos(theta4)*cos(theta5)*sin(theta6) + cos(theta4)*cos(theta5)*sin(theta2)*sin(theta3)*sin(theta6)) - 2*(thetadot2*cos(theta2)*((cos(theta3)*cos(theta5))/10 - (cos(theta4)*sin(theta3)*sin(theta5))/10) - thetadot2*sin(theta2)*((cos(theta5)*sin(theta3))/10 + (cos(theta3)*cos(theta4)*sin(theta5))/10))*(cos(theta2)*cos(theta5)*sin(theta3) + cos(theta3)*cos(theta5)*sin(theta2) + cos(theta2)*cos(theta3)*cos(theta4)*sin(theta5) - cos(theta4)*sin(theta2)*sin(theta3)*sin(theta5)) - (thetadot2*cos(theta2)*((cos(theta3)*sin(theta5))/10 + (cos(theta4)*cos(theta5)*sin(theta3))/10) - thetadot2*sin(theta2)*((sin(theta3)*sin(theta5))/10 - (cos(theta3)*cos(theta4)*cos(theta5))/10))*(cos(theta2)*sin(theta3)*sin(theta5) + cos(theta3)*sin(theta2)*sin(theta5) - cos(theta2)*cos(theta3)*cos(theta4)*cos(theta5) + cos(theta4)*cos(theta5)*sin(theta2)*sin(theta3)) - (cos(theta2)*cos(theta5)*sin(theta3) + cos(theta3)*cos(theta5)*sin(theta2) + cos(theta2)*cos(theta3)*cos(theta4)*sin(theta5) - cos(theta4)*sin(theta2)*sin(theta3)*sin(theta5))*(((2*thetadot6)/5 + thetadot6*((2*cos(theta6))/5 - 2/5))*((cos(theta2)*cos(theta5)*cos(theta6)*sin(theta4))/5 - (2*cos(theta2)*cos(theta3)*cos(theta4)*sin(theta6))/5 - (cos(theta2)*cos(theta4)*sin(theta6))/5 + (2*cos(theta2)*cos(theta5)*sin(theta3)*sin(theta6))/5 + (2*cos(theta3)*cos(theta5)*sin(theta2)*sin(theta6))/5 + (2*cos(theta4)*sin(theta2)*sin(theta3)*sin(theta6))/5 + (2*cos(theta2)*cos(theta3)*cos(theta5)*cos(theta6)*sin(theta4))/5 + (2*cos(theta2)*cos(theta3)*cos(theta4)*sin(theta5)*sin(theta6))/5 - (2*cos(theta5)*cos(theta6)*sin(theta2)*sin(theta3)*sin(theta4))/5 - (2*cos(theta4)*sin(theta2)*sin(theta3)*sin(theta5)*sin(theta6))/5) - (thetadot5/10 + (cos(theta4)*(thetadot2 + thetadot3))/10 - (thetadot1*cos(theta2 + theta3)*sin(theta4))/10)*(cos(theta2)*sin(theta3)*sin(theta5) + cos(theta3)*sin(theta2)*sin(theta5) - cos(theta2)*cos(theta3)*cos(theta4)*cos(theta5) + cos(theta4)*cos(theta5)*sin(theta2)*sin(theta3)) + cos(theta2 + theta3)*sin(theta4)*((cos(theta5)*(sin(theta4)*(thetadot2 + thetadot3) + thetadot1*cos(theta2 + theta3)*cos(theta4)))/10 - (sin(theta5)*(thetadot4 + thetadot1*sin(theta2 + theta3)))/10) + (2*thetadot6*sin(theta6)*((cos(theta2)*cos(theta4)*cos(theta6))/5 + (2*cos(theta2)*cos(theta5)*sin(theta3))/5 + (2*cos(theta3)*cos(theta5)*sin(theta2))/5 + (2*cos(theta2)*cos(theta3)*cos(theta4)*cos(theta6))/5 + (2*cos(theta2)*cos(theta3)*cos(theta4)*sin(theta5))/5 - (2*cos(theta2)*cos(theta5)*cos(theta6)*sin(theta3))/5 - (2*cos(theta3)*cos(theta5)*cos(theta6)*sin(theta2))/5 - (2*cos(theta4)*cos(theta6)*sin(theta2)*sin(theta3))/5 + (cos(theta2)*cos(theta5)*sin(theta4)*sin(theta6))/5 - (2*cos(theta4)*sin(theta2)*sin(theta3)*sin(theta5))/5 - (2*cos(theta2)*cos(theta3)*cos(theta4)*cos(theta6)*sin(theta5))/5 + (2*cos(theta2)*cos(theta3)*cos(theta5)*sin(theta4)*sin(theta6))/5 + (2*cos(theta4)*cos(theta6)*sin(theta2)*sin(theta3)*sin(theta5))/5 - (2*cos(theta5)*sin(theta2)*sin(theta3)*sin(theta4)*sin(theta6))/5))/5) - (thetadot2*cos(theta2)*((2*cos(theta4)*sin(theta3)*sin(theta6))/5 + (2*cos(theta3)*cos(theta5)*sin(theta6))/5 - (2*cos(theta5)*cos(theta6)*sin(theta3)*sin(theta4))/5 - (2*cos(theta4)*sin(theta3)*sin(theta5)*sin(theta6))/5) - thetadot2*sin(theta2)*((2*cos(theta5)*sin(theta3)*sin(theta6))/5 - (cos(theta4)*sin(theta6))/5 - (2*cos(theta3)*cos(theta4)*sin(theta6))/5 + (cos(theta5)*cos(theta6)*sin(theta4))/5 + (2*cos(theta3)*cos(theta5)*cos(theta6)*sin(theta4))/5 + (2*cos(theta3)*cos(theta4)*sin(theta5)*sin(theta6))/5))*((cos(theta2)*cos(theta5)*cos(theta6)*sin(theta4))/5 - (2*cos(theta2)*cos(theta3)*cos(theta4)*sin(theta6))/5 - (cos(theta2)*cos(theta4)*sin(theta6))/5 + (2*cos(theta2)*cos(theta5)*sin(theta3)*sin(theta6))/5 + (2*cos(theta3)*cos(theta5)*sin(theta2)*sin(theta6))/5 + (2*cos(theta4)*sin(theta2)*sin(theta3)*sin(theta6))/5 + (2*cos(theta2)*cos(theta3)*cos(theta5)*cos(theta6)*sin(theta4))/5 + (2*cos(theta2)*cos(theta3)*cos(theta4)*sin(theta5)*sin(theta6))/5 - (2*cos(theta5)*cos(theta6)*sin(theta2)*sin(theta3)*sin(theta4))/5 - (2*cos(theta4)*sin(theta2)*sin(theta3)*sin(theta5)*sin(theta6))/5) + ((sin(theta6)*(cos(theta5)*(sin(theta4)*(thetadot2 + thetadot3) + thetadot1*cos(theta2 + theta3)*cos(theta4)) - sin(theta5)*(thetadot4 + thetadot1*sin(theta2 + theta3))) + cos(theta6)*(thetadot5 + cos(theta4)*(thetadot2 + thetadot3) - thetadot1*cos(theta2 + theta3)*sin(theta4)))*((cos(theta2)*cos(theta5)*cos(theta6)*sin(theta4))/5 - (2*cos(theta2)*cos(theta3)*cos(theta4)*sin(theta6))/5 - (cos(theta2)*cos(theta4)*sin(theta6))/5 + (2*cos(theta2)*cos(theta5)*sin(theta3)*sin(theta6))/5 + (2*cos(theta3)*cos(theta5)*sin(theta2)*sin(theta6))/5 + (2*cos(theta4)*sin(theta2)*sin(theta3)*sin(theta6))/5 + (2*cos(theta2)*cos(theta3)*cos(theta5)*cos(theta6)*sin(theta4))/5 + (2*cos(theta2)*cos(theta3)*cos(theta4)*sin(theta5)*sin(theta6))/5 - (2*cos(theta5)*cos(theta6)*sin(theta2)*sin(theta3)*sin(theta4))/5 - (2*cos(theta4)*sin(theta2)*sin(theta3)*sin(theta5)*sin(theta6))/5) + (sin(theta6)*(thetadot5 + cos(theta4)*(thetadot2 + thetadot3) - thetadot1*cos(theta2 + theta3)*sin(theta4)) - cos(theta6)*(cos(theta5)*(sin(theta4)*(thetadot2 + thetadot3) + thetadot1*cos(theta2 + theta3)*cos(theta4)) - sin(theta5)*(thetadot4 + thetadot1*sin(theta2 + theta3))))*((cos(theta2)*cos(theta4)*cos(theta6))/5 + (2*cos(theta2)*cos(theta5)*sin(theta3))/5 + (2*cos(theta3)*cos(theta5)*sin(theta2))/5 + (2*cos(theta2)*cos(theta3)*cos(theta4)*cos(theta6))/5 + (2*cos(theta2)*cos(theta3)*cos(theta4)*sin(theta5))/5 - (2*cos(theta2)*cos(theta5)*cos(theta6)*sin(theta3))/5 - (2*cos(theta3)*cos(theta5)*cos(theta6)*sin(theta2))/5 - (2*cos(theta4)*cos(theta6)*sin(theta2)*sin(theta3))/5 + (cos(theta2)*cos(theta5)*sin(theta4)*sin(theta6))/5 - (2*cos(theta4)*sin(theta2)*sin(theta3)*sin(theta5))/5 - (2*cos(theta2)*cos(theta3)*cos(theta4)*cos(theta6)*sin(theta5))/5 + (2*cos(theta2)*cos(theta3)*cos(theta5)*sin(theta4)*sin(theta6))/5 + (2*cos(theta4)*cos(theta6)*sin(theta2)*sin(theta3)*sin(theta5))/5 - (2*cos(theta5)*sin(theta2)*sin(theta3)*sin(theta4)*sin(theta6))/5) - ((sin(theta6)*(2*thetadot2*sin(theta4) + 2*thetadot3*sin(theta4) + thetadot1*cos(theta2)*cos(theta4) + thetadot2*cos(theta3)*sin(theta4) + 2*thetadot1*cos(theta2)*cos(theta3)*cos(theta4) - 2*thetadot1*cos(theta4)*sin(theta2)*sin(theta3)))/5 + (cos(theta6)*(2*thetadot2*cos(theta4)*cos(theta5) + 2*thetadot3*cos(theta4)*cos(theta5) - thetadot2*sin(theta3)*sin(theta5) + thetadot2*cos(theta3)*cos(theta4)*cos(theta5) - thetadot1*cos(theta2)*cos(theta5)*sin(theta4) - 2*thetadot1*cos(theta2)*cos(theta3)*cos(theta5)*sin(theta4) + 2*thetadot1*cos(theta5)*sin(theta2)*sin(theta3)*sin(theta4)))/5 - (2*sin(theta6)*(sin(theta5)*(thetadot2*sin(theta4) + thetadot3*sin(theta4) + thetadot1*cos(theta2 + theta3)*cos(theta4)) + cos(theta5)*(thetadot4 + thetadot1*sin(theta2 + theta3))))/5)*(cos(theta2)*cos(theta3)*cos(theta6)*sin(theta4) - cos(theta6)*sin(theta2)*sin(theta3)*sin(theta4) + cos(theta2)*sin(theta3)*sin(theta5)*sin(theta6) + cos(theta3)*sin(theta2)*sin(theta5)*sin(theta6) - cos(theta2)*cos(theta3)*cos(theta4)*cos(theta5)*sin(theta6) + cos(theta4)*cos(theta5)*sin(theta2)*sin(theta3)*sin(theta6)) - ((2*thetadot6)/5 - (sin(theta5)*(thetadot2*sin(theta4) + thetadot3*sin(theta4) + thetadot1*cos(theta2 + theta3)*cos(theta4)) + cos(theta5)*(thetadot4 + thetadot1*sin(theta2 + theta3)))*((2*cos(theta6))/5 - 2/5) - (sin(theta6)*(2*thetadot2*cos(theta4)*cos(theta5) + 2*thetadot3*cos(theta4)*cos(theta5) - thetadot2*sin(theta3)*sin(theta5) + thetadot2*cos(theta3)*cos(theta4)*cos(theta5) - thetadot1*cos(theta2)*cos(theta5)*sin(theta4) - 2*thetadot1*cos(theta2)*cos(theta3)*cos(theta5)*sin(theta4) + 2*thetadot1*cos(theta5)*sin(theta2)*sin(theta3)*sin(theta4)))/5 + (cos(theta6)*(2*thetadot2*sin(theta4) + 2*thetadot3*sin(theta4) + thetadot1*cos(theta2)*cos(theta4) + thetadot2*cos(theta3)*sin(theta4) + 2*thetadot1*cos(theta2)*cos(theta3)*cos(theta4) - 2*thetadot1*cos(theta4)*sin(theta2)*sin(theta3)))/5)*(cos(theta2)*cos(theta6)*sin(theta3)*sin(theta5) - cos(theta2)*cos(theta3)*sin(theta4)*sin(theta6) + cos(theta3)*cos(theta6)*sin(theta2)*sin(theta5) + sin(theta2)*sin(theta3)*sin(theta4)*sin(theta6) - cos(theta2)*cos(theta3)*cos(theta4)*cos(theta5)*cos(theta6) + cos(theta4)*cos(theta5)*cos(theta6)*sin(theta2)*sin(theta3)))*((cos(theta2)*sin(theta4)*sin(theta5))/5 + (2*sin(theta2)*sin(theta3)*sin(theta4))/5 - (2*cos(theta2)*cos(theta3)*sin(theta4))/5 + (2*cos(theta2)*cos(theta3)*cos(theta6)*sin(theta4))/5 + (2*cos(theta2)*cos(theta3)*sin(theta4)*sin(theta5))/5 - (2*cos(theta6)*sin(theta2)*sin(theta3)*sin(theta4))/5 + (2*cos(theta2)*sin(theta3)*sin(theta5)*sin(theta6))/5 + (2*cos(theta3)*sin(theta2)*sin(theta5)*sin(theta6))/5 - (2*sin(theta2)*sin(theta3)*sin(theta4)*sin(theta5))/5 - (2*cos(theta2)*cos(theta3)*cos(theta4)*cos(theta5)*sin(theta6))/5 + (2*cos(theta4)*cos(theta5)*sin(theta2)*sin(theta3)*sin(theta6))/5) + (thetadot2*cos(theta2)*((2*cos(theta4)*sin(theta3)*sin(theta5))/5 - (2*cos(theta3)*cos(theta5))/5 + (2*cos(theta3)*cos(theta5)*cos(theta6))/5 + (2*cos(theta4)*cos(theta6)*sin(theta3))/5 - (2*cos(theta4)*cos(theta6)*sin(theta3)*sin(theta5))/5 + (2*cos(theta5)*sin(theta3)*sin(theta4)*sin(theta6))/5) + thetadot2*sin(theta2)*((cos(theta4)*cos(theta6))/5 + (2*cos(theta5)*sin(theta3))/5 + (cos(theta5)*sin(theta4)*sin(theta6))/5 + (2*cos(theta3)*cos(theta4)*cos(theta6))/5 + (2*cos(theta3)*cos(theta4)*sin(theta5))/5 - (2*cos(theta5)*cos(theta6)*sin(theta3))/5 - (2*cos(theta3)*cos(theta4)*cos(theta6)*sin(theta5))/5 + (2*cos(theta3)*cos(theta5)*sin(theta4)*sin(theta6))/5))*((cos(theta2)*cos(theta4)*cos(theta6))/5 + (2*cos(theta2)*cos(theta5)*sin(theta3))/5 + (2*cos(theta3)*cos(theta5)*sin(theta2))/5 + (2*cos(theta2)*cos(theta3)*cos(theta4)*cos(theta6))/5 + (2*cos(theta2)*cos(theta3)*cos(theta4)*sin(theta5))/5 - (2*cos(theta2)*cos(theta5)*cos(theta6)*sin(theta3))/5 - (2*cos(theta3)*cos(theta5)*cos(theta6)*sin(theta2))/5 - (2*cos(theta4)*cos(theta6)*sin(theta2)*sin(theta3))/5 + (cos(theta2)*cos(theta5)*sin(theta4)*sin(theta6))/5 - (2*cos(theta4)*sin(theta2)*sin(theta3)*sin(theta5))/5 - (2*cos(theta2)*cos(theta3)*cos(theta4)*cos(theta6)*sin(theta5))/5 + (2*cos(theta2)*cos(theta3)*cos(theta5)*sin(theta4)*sin(theta6))/5 + (2*cos(theta4)*cos(theta6)*sin(theta2)*sin(theta3)*sin(theta5))/5 - (2*cos(theta5)*sin(theta2)*sin(theta3)*sin(theta4)*sin(theta6))/5) + cos(theta2)*((thetadot2*sin(theta2))/10 - (thetadot3*sin(theta3)*((sin(theta4)*sin(theta6))/10 + (cos(theta4)*cos(theta5)*cos(theta6))/10) + (thetadot3*cos(theta3)*cos(theta6)*sin(theta5))/10)*(cos(theta2)*cos(theta6)*sin(theta3)*sin(theta5) - cos(theta2)*cos(theta3)*sin(theta4)*sin(theta6) + cos(theta3)*cos(theta6)*sin(theta2)*sin(theta5) + sin(theta2)*sin(theta3)*sin(theta4)*sin(theta6) - cos(theta2)*cos(theta3)*cos(theta4)*cos(theta5)*cos(theta6) + cos(theta4)*cos(theta5)*cos(theta6)*sin(theta2)*sin(theta3)) - (thetadot3*sin(theta3)*((2*sin(theta4))/5 - (2*cos(theta6)*sin(theta4))/5 - (2*sin(theta4)*sin(theta5))/5 + (2*cos(theta4)*cos(theta5)*sin(theta6))/5) + (2*thetadot3*cos(theta3)*sin(theta5)*sin(theta6))/5)*((cos(theta2)*sin(theta4)*sin(theta5))/5 + (2*sin(theta2)*sin(theta3)*sin(theta4))/5 - (2*cos(theta2)*cos(theta3)*sin(theta4))/5 + (2*cos(theta2)*cos(theta3)*cos(theta6)*sin(theta4))/5 + (2*cos(theta2)*cos(theta3)*sin(theta4)*sin(theta5))/5 - (2*cos(theta6)*sin(theta2)*sin(theta3)*sin(theta4))/5 + (2*cos(theta2)*sin(theta3)*sin(theta5)*sin(theta6))/5 + (2*cos(theta3)*sin(theta2)*sin(theta5)*sin(theta6))/5 - (2*sin(theta2)*sin(theta3)*sin(theta4)*sin(theta5))/5 - (2*cos(theta2)*cos(theta3)*cos(theta4)*cos(theta5)*sin(theta6))/5 + (2*cos(theta4)*cos(theta5)*sin(theta2)*sin(theta3)*sin(theta6))/5) + (thetadot3*sin(theta3)*((2*cos(theta4)*cos(theta6))/5 + (2*cos(theta4)*sin(theta5))/5 + (2*cos(theta5)*sin(theta4)*sin(theta6))/5 - (2*cos(theta4)*cos(theta6)*sin(theta5))/5) + (2*thetadot3*cos(theta3)*cos(theta5)*(cos(theta6) - 1))/5)*((cos(theta2)*cos(theta4)*cos(theta6))/5 + (2*cos(theta2)*cos(theta5)*sin(theta3))/5 + (2*cos(theta3)*cos(theta5)*sin(theta2))/5 + (2*cos(theta2)*cos(theta3)*cos(theta4)*cos(theta6))/5 + (2*cos(theta2)*cos(theta3)*cos(theta4)*sin(theta5))/5 - (2*cos(theta2)*cos(theta5)*cos(theta6)*sin(theta3))/5 - (2*cos(theta3)*cos(theta5)*cos(theta6)*sin(theta2))/5 - (2*cos(theta4)*cos(theta6)*sin(theta2)*sin(theta3))/5 + (cos(theta2)*cos(theta5)*sin(theta4)*sin(theta6))/5 - (2*cos(theta4)*sin(theta2)*sin(theta3)*sin(theta5))/5 - (2*cos(theta2)*cos(theta3)*cos(theta4)*cos(theta6)*sin(theta5))/5 + (2*cos(theta2)*cos(theta3)*cos(theta5)*sin(theta4)*sin(theta6))/5 + (2*cos(theta4)*cos(theta6)*sin(theta2)*sin(theta3)*sin(theta5))/5 - (2*cos(theta5)*sin(theta2)*sin(theta3)*sin(theta4)*sin(theta6))/5) - 2*((thetadot3*cos(theta3)*cos(theta5))/10 - (thetadot3*cos(theta4)*sin(theta3)*sin(theta5))/10)*(cos(theta2)*cos(theta5)*sin(theta3) + cos(theta3)*cos(theta5)*sin(theta2) + cos(theta2)*cos(theta3)*cos(theta4)*sin(theta5) - cos(theta4)*sin(theta2)*sin(theta3)*sin(theta5)) - ((thetadot3*cos(theta3)*sin(theta5))/10 + (thetadot3*cos(theta4)*cos(theta5)*sin(theta3))/10)*(cos(theta2)*sin(theta3)*sin(theta5) + cos(theta3)*sin(theta2)*sin(theta5) - cos(theta2)*cos(theta3)*cos(theta4)*cos(theta5) + cos(theta4)*cos(theta5)*sin(theta2)*sin(theta3)) + (thetadot3*sin(theta3)*((cos(theta6)*sin(theta4))/10 - (cos(theta4)*cos(theta5)*sin(theta6))/10) - (thetadot3*cos(theta3)*sin(theta5)*sin(theta6))/10)*(cos(theta2)*cos(theta3)*cos(theta6)*sin(theta4) - cos(theta6)*sin(theta2)*sin(theta3)*sin(theta4) + cos(theta2)*sin(theta3)*sin(theta5)*sin(theta6) + cos(theta3)*sin(theta2)*sin(theta5)*sin(theta6) - cos(theta2)*cos(theta3)*cos(theta4)*cos(theta5)*sin(theta6) + cos(theta4)*cos(theta5)*sin(theta2)*sin(theta3)*sin(theta6)) + (thetadot3*sin(theta3)*((2*cos(theta4)*sin(theta5)*sin(theta6))/5 - (2*cos(theta4)*sin(theta6))/5 + (2*cos(theta5)*cos(theta6)*sin(theta4))/5) - (2*thetadot3*cos(theta3)*cos(theta5)*sin(theta6))/5)*((cos(theta2)*cos(theta5)*cos(theta6)*sin(theta4))/5 - (2*cos(theta2)*cos(theta3)*cos(theta4)*sin(theta6))/5 - (cos(theta2)*cos(theta4)*sin(theta6))/5 + (2*cos(theta2)*cos(theta5)*sin(theta3)*sin(theta6))/5 + (2*cos(theta3)*cos(theta5)*sin(theta2)*sin(theta6))/5 + (2*cos(theta4)*sin(theta2)*sin(theta3)*sin(theta6))/5 + (2*cos(theta2)*cos(theta3)*cos(theta5)*cos(theta6)*sin(theta4))/5 + (2*cos(theta2)*cos(theta3)*cos(theta4)*sin(theta5)*sin(theta6))/5 - (2*cos(theta5)*cos(theta6)*sin(theta2)*sin(theta3)*sin(theta4))/5 - (2*cos(theta4)*sin(theta2)*sin(theta3)*sin(theta5)*sin(theta6))/5) + (thetadot3*cos(theta2 + theta3)*sin(theta3))/10 - (thetadot3*sin(theta2 + theta3)*cos(theta3))/5 + (2*thetadot3*cos(theta4)^2*sin(theta3)*(2*cos(theta2 + theta3) + cos(theta2)))/25 + (thetadot3*cos(theta2 + theta3)*cos(theta4)^2*sin(theta3))/10 + (thetadot3*cos(theta2 + theta3)*sin(theta3)*sin(theta4)^2)/5 + (thetadot3*cos(theta4)^2*sin(theta3)*(cos(theta2 + theta3) + cos(theta2)))/25 + (thetadot3*sin(theta3)*sin(theta4)^2*(cos(theta2 + theta3) + cos(theta2)))/25 + (2*thetadot3*cos(theta5)^2*sin(theta3)*sin(theta4)^2*(2*cos(theta2 + theta3) + cos(theta2)))/25 + (2*thetadot3*sin(theta3)*sin(theta4)^2*sin(theta5)^2*(2*cos(theta2 + theta3) + cos(theta2)))/25) - (cos(theta2)*((thetadot4*sin(theta4)*sin(theta6) + thetadot4*cos(theta4)*cos(theta5)*cos(theta6))*((cos(theta2)*cos(theta5)*cos(theta6)*sin(theta4))/5 - (2*cos(theta2)*cos(theta3)*cos(theta4)*sin(theta6))/5 - (cos(theta2)*cos(theta4)*sin(theta6))/5 + (2*cos(theta2)*cos(theta5)*sin(theta3)*sin(theta6))/5 + (2*cos(theta3)*cos(theta5)*sin(theta2)*sin(theta6))/5 + (2*cos(theta4)*sin(theta2)*sin(theta3)*sin(theta6))/5 + (2*cos(theta2)*cos(theta3)*cos(theta5)*cos(theta6)*sin(theta4))/5 + (2*cos(theta2)*cos(theta3)*cos(theta4)*sin(theta5)*sin(theta6))/5 - (2*cos(theta5)*cos(theta6)*sin(theta2)*sin(theta3)*sin(theta4))/5 - (2*cos(theta4)*sin(theta2)*sin(theta3)*sin(theta5)*sin(theta6))/5) - (thetadot4*cos(theta6)*sin(theta4) - thetadot4*cos(theta4)*cos(theta5)*sin(theta6))*((cos(theta2)*cos(theta4)*cos(theta6))/5 + (2*cos(theta2)*cos(theta5)*sin(theta3))/5 + (2*cos(theta3)*cos(theta5)*sin(theta2))/5 + (2*cos(theta2)*cos(theta3)*cos(theta4)*cos(theta6))/5 + (2*cos(theta2)*cos(theta3)*cos(theta4)*sin(theta5))/5 - (2*cos(theta2)*cos(theta5)*cos(theta6)*sin(theta3))/5 - (2*cos(theta3)*cos(theta5)*cos(theta6)*sin(theta2))/5 - (2*cos(theta4)*cos(theta6)*sin(theta2)*sin(theta3))/5 + (cos(theta2)*cos(theta5)*sin(theta4)*sin(theta6))/5 - (2*cos(theta4)*sin(theta2)*sin(theta3)*sin(theta5))/5 - (2*cos(theta2)*cos(theta3)*cos(theta4)*cos(theta6)*sin(theta5))/5 + (2*cos(theta2)*cos(theta3)*cos(theta5)*sin(theta4)*sin(theta6))/5 + (2*cos(theta4)*cos(theta6)*sin(theta2)*sin(theta3)*sin(theta5))/5 - (2*cos(theta5)*sin(theta2)*sin(theta3)*sin(theta4)*sin(theta6))/5) + (thetadot2*cos(theta2 + theta3)*sin(theta3))/5 - (thetadot2*sin(theta2 + theta3)*cos(theta3))/5 - (thetadot4*cos(theta4)*sin(theta4)*(2*cos(theta2 + theta3) + cos(theta2)))/5 + thetadot4*cos(theta4)*sin(theta5)*((cos(theta2)*sin(theta4)*sin(theta5))/5 + (2*sin(theta2)*sin(theta3)*sin(theta4))/5 - (2*cos(theta2)*cos(theta3)*sin(theta4))/5 + (2*cos(theta2)*cos(theta3)*cos(theta6)*sin(theta4))/5 + (2*cos(theta2)*cos(theta3)*sin(theta4)*sin(theta5))/5 - (2*cos(theta6)*sin(theta2)*sin(theta3)*sin(theta4))/5 + (2*cos(theta2)*sin(theta3)*sin(theta5)*sin(theta6))/5 + (2*cos(theta3)*sin(theta2)*sin(theta5)*sin(theta6))/5 - (2*sin(theta2)*sin(theta3)*sin(theta4)*sin(theta5))/5 - (2*cos(theta2)*cos(theta3)*cos(theta4)*cos(theta5)*sin(theta6))/5 + (2*cos(theta4)*cos(theta5)*sin(theta2)*sin(theta3)*sin(theta6))/5) + (thetadot4*cos(theta4)*cos(theta5)^2*sin(theta4)*(2*cos(theta2 + theta3) + cos(theta2)))/5 + (thetadot4*cos(theta4)*sin(theta4)*sin(theta5)^2*(2*cos(theta2 + theta3) + cos(theta2)))/5))/5 - (((sin(theta6)*(cos(theta5)*(sin(theta4)*(thetadot2 + thetadot3) + thetadot1*cos(theta2 + theta3)*cos(theta4)) - sin(theta5)*(thetadot4 + thetadot1*sin(theta2 + theta3))))/10 + (cos(theta6)*(thetadot5 + cos(theta4)*(thetadot2 + thetadot3) - thetadot1*cos(theta2 + theta3)*sin(theta4)))/10)*(cos(theta2)*cos(theta6)*sin(theta3)*sin(theta5) - cos(theta2)*cos(theta3)*sin(theta4)*sin(theta6) + cos(theta3)*cos(theta6)*sin(theta2)*sin(theta5) + sin(theta2)*sin(theta3)*sin(theta4)*sin(theta6) - cos(theta2)*cos(theta3)*cos(theta4)*cos(theta5)*cos(theta6) + cos(theta4)*cos(theta5)*cos(theta6)*sin(theta2)*sin(theta3)) + ((sin(theta6)*(thetadot5 + cos(theta4)*(thetadot2 + thetadot3) - thetadot1*cos(theta2 + theta3)*sin(theta4)))/10 - (cos(theta6)*(cos(theta5)*(sin(theta4)*(thetadot2 + thetadot3) + thetadot1*cos(theta2 + theta3)*cos(theta4)) - sin(theta5)*(thetadot4 + thetadot1*sin(theta2 + theta3))))/10)*(cos(theta2)*cos(theta3)*cos(theta6)*sin(theta4) - cos(theta6)*sin(theta2)*sin(theta3)*sin(theta4) + cos(theta2)*sin(theta3)*sin(theta5)*sin(theta6) + cos(theta3)*sin(theta2)*sin(theta5)*sin(theta6) - cos(theta2)*cos(theta3)*cos(theta4)*cos(theta5)*sin(theta6) + cos(theta4)*cos(theta5)*sin(theta2)*sin(theta3)*sin(theta6)))*(cos(theta2)*cos(theta5)*sin(theta3) + cos(theta3)*cos(theta5)*sin(theta2) + cos(theta2)*cos(theta3)*cos(theta4)*sin(theta5) - cos(theta4)*sin(theta2)*sin(theta3)*sin(theta5)) - (((sin(theta6)*(2*thetadot2*sin(theta4) + 2*thetadot3*sin(theta4) + thetadot1*cos(theta2)*cos(theta4) + thetadot2*cos(theta3)*sin(theta4) + 2*thetadot1*cos(theta2)*cos(theta3)*cos(theta4) - 2*thetadot1*cos(theta4)*sin(theta2)*sin(theta3)))/5 + (cos(theta6)*(2*thetadot2*cos(theta4)*cos(theta5) + 2*thetadot3*cos(theta4)*cos(theta5) - thetadot2*sin(theta3)*sin(theta5) + thetadot2*cos(theta3)*cos(theta4)*cos(theta5) - thetadot1*cos(theta2)*cos(theta5)*sin(theta4) - 2*thetadot1*cos(theta2)*cos(theta3)*cos(theta5)*sin(theta4) + 2*thetadot1*cos(theta5)*sin(theta2)*sin(theta3)*sin(theta4)))/5 - (2*sin(theta6)*(sin(theta5)*(thetadot2*sin(theta4) + thetadot3*sin(theta4) + thetadot1*cos(theta2 + theta3)*cos(theta4)) + cos(theta5)*(thetadot4 + thetadot1*sin(theta2 + theta3))))/5)*(cos(theta2)*cos(theta5)*sin(theta3) + cos(theta3)*cos(theta5)*sin(theta2) + cos(theta2)*cos(theta3)*cos(theta4)*sin(theta5) - cos(theta4)*sin(theta2)*sin(theta3)*sin(theta5)) + ((sin(theta5)*(thetadot2*cos(theta4) + thetadot3*cos(theta4) - thetadot1*cos(theta2 + theta3)*sin(theta4)))/5 + sin(theta5)*((thetadot2*cos(theta4))/5 + (thetadot3*cos(theta4))/5 - (thetadot1*cos(theta2 + theta3)*sin(theta4))/5 + (thetadot2*cos(theta3)*cos(theta4))/5 - (thetadot1*cos(theta2)*sin(theta4))/5) + ((2*cos(theta6))/5 - 2/5)*(thetadot5 + thetadot2*cos(theta4) + thetadot3*cos(theta4) - thetadot1*cos(theta2 + theta3)*sin(theta4)) + (2*sin(theta6)*(cos(theta5)*(thetadot2*sin(theta4) + thetadot3*sin(theta4) + thetadot1*cos(theta2 + theta3)*cos(theta4)) - sin(theta5)*(thetadot4 + thetadot1*sin(theta2 + theta3))))/5 + (thetadot2*cos(theta5)*sin(theta3))/5)*(cos(theta2)*cos(theta6)*sin(theta3)*sin(theta5) - cos(theta2)*cos(theta3)*sin(theta4)*sin(theta6) + cos(theta3)*cos(theta6)*sin(theta2)*sin(theta5) + sin(theta2)*sin(theta3)*sin(theta4)*sin(theta6) - cos(theta2)*cos(theta3)*cos(theta4)*cos(theta5)*cos(theta6) + cos(theta4)*cos(theta5)*cos(theta6)*sin(theta2)*sin(theta3)) + (sin(theta6)*(thetadot5 + cos(theta4)*(thetadot2 + thetadot3) - thetadot1*cos(theta2 + theta3)*sin(theta4)) - cos(theta6)*(cos(theta5)*(sin(theta4)*(thetadot2 + thetadot3) + thetadot1*cos(theta2 + theta3)*cos(theta4)) - sin(theta5)*(thetadot4 + thetadot1*sin(theta2 + theta3))))*((cos(theta2)*sin(theta4)*sin(theta5))/5 + (2*sin(theta2)*sin(theta3)*sin(theta4))/5 - (2*cos(theta2)*cos(theta3)*sin(theta4))/5 + (2*cos(theta2)*cos(theta3)*cos(theta6)*sin(theta4))/5 + (2*cos(theta2)*cos(theta3)*sin(theta4)*sin(theta5))/5 - (2*cos(theta6)*sin(theta2)*sin(theta3)*sin(theta4))/5 + (2*cos(theta2)*sin(theta3)*sin(theta5)*sin(theta6))/5 + (2*cos(theta3)*sin(theta2)*sin(theta5)*sin(theta6))/5 - (2*sin(theta2)*sin(theta3)*sin(theta4)*sin(theta5))/5 - (2*cos(theta2)*cos(theta3)*cos(theta4)*cos(theta5)*sin(theta6))/5 + (2*cos(theta4)*cos(theta5)*sin(theta2)*sin(theta3)*sin(theta6))/5) + (thetadot6 + sin(theta5)*(sin(theta4)*(thetadot2 + thetadot3) + thetadot1*cos(theta2 + theta3)*cos(theta4)) + cos(theta5)*(thetadot4 + thetadot1*sin(theta2 + theta3)))*((cos(theta2)*cos(theta5)*cos(theta6)*sin(theta4))/5 - (2*cos(theta2)*cos(theta3)*cos(theta4)*sin(theta6))/5 - (cos(theta2)*cos(theta4)*sin(theta6))/5 + (2*cos(theta2)*cos(theta5)*sin(theta3)*sin(theta6))/5 + (2*cos(theta3)*cos(theta5)*sin(theta2)*sin(theta6))/5 + (2*cos(theta4)*sin(theta2)*sin(theta3)*sin(theta6))/5 + (2*cos(theta2)*cos(theta3)*cos(theta5)*cos(theta6)*sin(theta4))/5 + (2*cos(theta2)*cos(theta3)*cos(theta4)*sin(theta5)*sin(theta6))/5 - (2*cos(theta5)*cos(theta6)*sin(theta2)*sin(theta3)*sin(theta4))/5 - (2*cos(theta4)*sin(theta2)*sin(theta3)*sin(theta5)*sin(theta6))/5))*((cos(theta2)*cos(theta4)*cos(theta6))/5 + (2*cos(theta2)*cos(theta5)*sin(theta3))/5 + (2*cos(theta3)*cos(theta5)*sin(theta2))/5 + (2*cos(theta2)*cos(theta3)*cos(theta4)*cos(theta6))/5 + (2*cos(theta2)*cos(theta3)*cos(theta4)*sin(theta5))/5 - (2*cos(theta2)*cos(theta5)*cos(theta6)*sin(theta3))/5 - (2*cos(theta3)*cos(theta5)*cos(theta6)*sin(theta2))/5 - (2*cos(theta4)*cos(theta6)*sin(theta2)*sin(theta3))/5 + (cos(theta2)*cos(theta5)*sin(theta4)*sin(theta6))/5 - (2*cos(theta4)*sin(theta2)*sin(theta3)*sin(theta5))/5 - (2*cos(theta2)*cos(theta3)*cos(theta4)*cos(theta6)*sin(theta5))/5 + (2*cos(theta2)*cos(theta3)*cos(theta5)*sin(theta4)*sin(theta6))/5 + (2*cos(theta4)*cos(theta6)*sin(theta2)*sin(theta3)*sin(theta5))/5 - (2*cos(theta5)*sin(theta2)*sin(theta3)*sin(theta4)*sin(theta6))/5) + cos(theta2 + theta3)*((thetadot2*cos(theta2)*sin(theta3))/10 + (thetadot2*cos(theta3)*sin(theta2))/10) - 2*sin(theta2 + theta3)*((thetadot2*cos(theta2)*cos(theta3))/10 - (thetadot2*sin(theta2)*sin(theta3))/10) - (thetadot2*cos(theta2)*((2*sin(theta3)*sin(theta4))/5 - (2*cos(theta6)*sin(theta3)*sin(theta4))/5 + (2*cos(theta3)*sin(theta5)*sin(theta6))/5 - (2*sin(theta3)*sin(theta4)*sin(theta5))/5 + (2*cos(theta4)*cos(theta5)*sin(theta3)*sin(theta6))/5) - thetadot2*sin(theta2)*((sin(theta4)*sin(theta5))/5 - (2*cos(theta3)*sin(theta4))/5 + (2*cos(theta3)*sin(theta4)*sin(theta5))/5 + (2*sin(theta3)*sin(theta5)*sin(theta6))/5 + (2*cos(theta3)*cos(theta6)*sin(theta4))/5 - (2*cos(theta3)*cos(theta4)*cos(theta5)*sin(theta6))/5))*((cos(theta2)*sin(theta4)*sin(theta5))/5 + (2*sin(theta2)*sin(theta3)*sin(theta4))/5 - (2*cos(theta2)*cos(theta3)*sin(theta4))/5 + (2*cos(theta2)*cos(theta3)*cos(theta6)*sin(theta4))/5 + (2*cos(theta2)*cos(theta3)*sin(theta4)*sin(theta5))/5 - (2*cos(theta6)*sin(theta2)*sin(theta3)*sin(theta4))/5 + (2*cos(theta2)*sin(theta3)*sin(theta5)*sin(theta6))/5 + (2*cos(theta3)*sin(theta2)*sin(theta5)*sin(theta6))/5 - (2*sin(theta2)*sin(theta3)*sin(theta4)*sin(theta5))/5 - (2*cos(theta2)*cos(theta3)*cos(theta4)*cos(theta5)*sin(theta6))/5 + (2*cos(theta4)*cos(theta5)*sin(theta2)*sin(theta3)*sin(theta6))/5) - sin(theta2 + theta3)*(cos(theta2 + theta3)*cos(theta4)*((cos(theta4)*(thetadot2 + thetadot3))/10 - (thetadot1*cos(theta2 + theta3)*sin(theta4))/10) + cos(theta2 + theta3)*sin(theta4)*((sin(theta4)*(thetadot2 + thetadot3))/10 + (thetadot1*cos(theta2 + theta3)*cos(theta4))/10) + (thetadot5*cos(theta5)*(cos(theta2)*sin(theta3)*sin(theta5) + cos(theta3)*sin(theta2)*sin(theta5) - cos(theta2)*cos(theta3)*cos(theta4)*cos(theta5) + cos(theta4)*cos(theta5)*sin(theta2)*sin(theta3)))/10 - (thetadot5*sin(theta5)*(cos(theta2)*cos(theta5)*sin(theta3) + cos(theta3)*cos(theta5)*sin(theta2) + cos(theta2)*cos(theta3)*cos(theta4)*sin(theta5) - cos(theta4)*sin(theta2)*sin(theta3)*sin(theta5)))/5 - (2*thetadot5*sin(theta5)*sin(theta6)*((cos(theta2)*cos(theta5)*cos(theta6)*sin(theta4))/5 - (2*cos(theta2)*cos(theta3)*cos(theta4)*sin(theta6))/5 - (cos(theta2)*cos(theta4)*sin(theta6))/5 + (2*cos(theta2)*cos(theta5)*sin(theta3)*sin(theta6))/5 + (2*cos(theta3)*cos(theta5)*sin(theta2)*sin(theta6))/5 + (2*cos(theta4)*sin(theta2)*sin(theta3)*sin(theta6))/5 + (2*cos(theta2)*cos(theta3)*cos(theta5)*cos(theta6)*sin(theta4))/5 + (2*cos(theta2)*cos(theta3)*cos(theta4)*sin(theta5)*sin(theta6))/5 - (2*cos(theta5)*cos(theta6)*sin(theta2)*sin(theta3)*sin(theta4))/5 - (2*cos(theta4)*sin(theta2)*sin(theta3)*sin(theta5)*sin(theta6))/5))/5 + thetadot5*sin(theta5)*((2*cos(theta6))/5 - 2/5)*((cos(theta2)*cos(theta4)*cos(theta6))/5 + (2*cos(theta2)*cos(theta5)*sin(theta3))/5 + (2*cos(theta3)*cos(theta5)*sin(theta2))/5 + (2*cos(theta2)*cos(theta3)*cos(theta4)*cos(theta6))/5 + (2*cos(theta2)*cos(theta3)*cos(theta4)*sin(theta5))/5 - (2*cos(theta2)*cos(theta5)*cos(theta6)*sin(theta3))/5 - (2*cos(theta3)*cos(theta5)*cos(theta6)*sin(theta2))/5 - (2*cos(theta4)*cos(theta6)*sin(theta2)*sin(theta3))/5 + (cos(theta2)*cos(theta5)*sin(theta4)*sin(theta6))/5 - (2*cos(theta4)*sin(theta2)*sin(theta3)*sin(theta5))/5 - (2*cos(theta2)*cos(theta3)*cos(theta4)*cos(theta6)*sin(theta5))/5 + (2*cos(theta2)*cos(theta3)*cos(theta5)*sin(theta4)*sin(theta6))/5 + (2*cos(theta4)*cos(theta6)*sin(theta2)*sin(theta3)*sin(theta5))/5 - (2*cos(theta5)*sin(theta2)*sin(theta3)*sin(theta4)*sin(theta6))/5) + (thetadot5*cos(theta5)*cos(theta6)*(cos(theta2)*cos(theta6)*sin(theta3)*sin(theta5) - cos(theta2)*cos(theta3)*sin(theta4)*sin(theta6) + cos(theta3)*cos(theta6)*sin(theta2)*sin(theta5) + sin(theta2)*sin(theta3)*sin(theta4)*sin(theta6) - cos(theta2)*cos(theta3)*cos(theta4)*cos(theta5)*cos(theta6) + cos(theta4)*cos(theta5)*cos(theta6)*sin(theta2)*sin(theta3)))/10 + (2*thetadot5*cos(theta5)*sin(theta6)*((cos(theta2)*sin(theta4)*sin(theta5))/5 + (2*sin(theta2)*sin(theta3)*sin(theta4))/5 - (2*cos(theta2)*cos(theta3)*sin(theta4))/5 + (2*cos(theta2)*cos(theta3)*cos(theta6)*sin(theta4))/5 + (2*cos(theta2)*cos(theta3)*sin(theta4)*sin(theta5))/5 - (2*cos(theta6)*sin(theta2)*sin(theta3)*sin(theta4))/5 + (2*cos(theta2)*sin(theta3)*sin(theta5)*sin(theta6))/5 + (2*cos(theta3)*sin(theta2)*sin(theta5)*sin(theta6))/5 - (2*sin(theta2)*sin(theta3)*sin(theta4)*sin(theta5))/5 - (2*cos(theta2)*cos(theta3)*cos(theta4)*cos(theta5)*sin(theta6))/5 + (2*cos(theta4)*cos(theta5)*sin(theta2)*sin(theta3)*sin(theta6))/5))/5 + (thetadot5*cos(theta5)*sin(theta6)*(cos(theta2)*cos(theta3)*cos(theta6)*sin(theta4) - cos(theta6)*sin(theta2)*sin(theta3)*sin(theta4) + cos(theta2)*sin(theta3)*sin(theta5)*sin(theta6) + cos(theta3)*sin(theta2)*sin(theta5)*sin(theta6) - cos(theta2)*cos(theta3)*cos(theta4)*cos(theta5)*sin(theta6) + cos(theta4)*cos(theta5)*sin(theta2)*sin(theta3)*sin(theta6)))/10) + ((thetadot6/10 + (sin(theta5)*(sin(theta4)*(thetadot2 + thetadot3) + thetadot1*cos(theta2 + theta3)*cos(theta4)))/10 + (cos(theta5)*(thetadot4 + thetadot1*sin(theta2 + theta3)))/10)*(cos(theta2)*cos(theta3)*cos(theta6)*sin(theta4) - cos(theta6)*sin(theta2)*sin(theta3)*sin(theta4) + cos(theta2)*sin(theta3)*sin(theta5)*sin(theta6) + cos(theta3)*sin(theta2)*sin(theta5)*sin(theta6) - cos(theta2)*cos(theta3)*cos(theta4)*cos(theta5)*sin(theta6) + cos(theta4)*cos(theta5)*sin(theta2)*sin(theta3)*sin(theta6)) + ((sin(theta6)*(cos(theta5)*(sin(theta4)*(thetadot2 + thetadot3) + thetadot1*cos(theta2 + theta3)*cos(theta4)) - sin(theta5)*(thetadot4 + thetadot1*sin(theta2 + theta3))))/10 + (cos(theta6)*(thetadot5 + cos(theta4)*(thetadot2 + thetadot3) - thetadot1*cos(theta2 + theta3)*sin(theta4)))/10)*(cos(theta2)*cos(theta5)*sin(theta3) + cos(theta3)*cos(theta5)*sin(theta2) + cos(theta2)*cos(theta3)*cos(theta4)*sin(theta5) - cos(theta4)*sin(theta2)*sin(theta3)*sin(theta5)))*(cos(theta2)*cos(theta6)*sin(theta3)*sin(theta5) - cos(theta2)*cos(theta3)*sin(theta4)*sin(theta6) + cos(theta3)*cos(theta6)*sin(theta2)*sin(theta5) + sin(theta2)*sin(theta3)*sin(theta4)*sin(theta6) - cos(theta2)*cos(theta3)*cos(theta4)*cos(theta5)*cos(theta6) + cos(theta4)*cos(theta5)*cos(theta6)*sin(theta2)*sin(theta3)) - ((thetadot6/10 + (sin(theta5)*(sin(theta4)*(thetadot2 + thetadot3) + thetadot1*cos(theta2 + theta3)*cos(theta4)))/10 + (cos(theta5)*(thetadot4 + thetadot1*sin(theta2 + theta3)))/10)*(cos(theta2)*cos(theta6)*sin(theta3)*sin(theta5) - cos(theta2)*cos(theta3)*sin(theta4)*sin(theta6) + cos(theta3)*cos(theta6)*sin(theta2)*sin(theta5) + sin(theta2)*sin(theta3)*sin(theta4)*sin(theta6) - cos(theta2)*cos(theta3)*cos(theta4)*cos(theta5)*cos(theta6) + cos(theta4)*cos(theta5)*cos(theta6)*sin(theta2)*sin(theta3)) - ((sin(theta6)*(thetadot5 + cos(theta4)*(thetadot2 + thetadot3) - thetadot1*cos(theta2 + theta3)*sin(theta4)))/10 - (cos(theta6)*(cos(theta5)*(sin(theta4)*(thetadot2 + thetadot3) + thetadot1*cos(theta2 + theta3)*cos(theta4)) - sin(theta5)*(thetadot4 + thetadot1*sin(theta2 + theta3))))/10)*(cos(theta2)*cos(theta5)*sin(theta3) + cos(theta3)*cos(theta5)*sin(theta2) + cos(theta2)*cos(theta3)*cos(theta4)*sin(theta5) - cos(theta4)*sin(theta2)*sin(theta3)*sin(theta5)))*(cos(theta2)*cos(theta3)*cos(theta6)*sin(theta4) - cos(theta6)*sin(theta2)*sin(theta3)*sin(theta4) + cos(theta2)*sin(theta3)*sin(theta5)*sin(theta6) + cos(theta3)*sin(theta2)*sin(theta5)*sin(theta6) - cos(theta2)*cos(theta3)*cos(theta4)*cos(theta5)*sin(theta6) + cos(theta4)*cos(theta5)*sin(theta2)*sin(theta3)*sin(theta6)) - (thetadot2*cos(theta2)*((sin(theta3)*sin(theta4)*sin(theta6))/10 + (cos(theta3)*cos(theta6)*sin(theta5))/10 + (cos(theta4)*cos(theta5)*cos(theta6)*sin(theta3))/10) + thetadot2*sin(theta2)*((cos(theta3)*sin(theta4)*sin(theta6))/10 - (cos(theta6)*sin(theta3)*sin(theta5))/10 + (cos(theta3)*cos(theta4)*cos(theta5)*cos(theta6))/10))*(cos(theta2)*cos(theta6)*sin(theta3)*sin(theta5) - cos(theta2)*cos(theta3)*sin(theta4)*sin(theta6) + cos(theta3)*cos(theta6)*sin(theta2)*sin(theta5) + sin(theta2)*sin(theta3)*sin(theta4)*sin(theta6) - cos(theta2)*cos(theta3)*cos(theta4)*cos(theta5)*cos(theta6) + cos(theta4)*cos(theta5)*cos(theta6)*sin(theta2)*sin(theta3)) - (cos(theta2)*sin(theta3)*sin(theta5) + cos(theta3)*sin(theta2)*sin(theta5) - cos(theta2)*cos(theta3)*cos(theta4)*cos(theta5) + cos(theta4)*cos(theta5)*sin(theta2)*sin(theta3))*((thetadot5/10 + (cos(theta4)*(thetadot2 + thetadot3))/10 - (thetadot1*cos(theta2 + theta3)*sin(theta4))/10)*(cos(theta2)*cos(theta5)*sin(theta3) + cos(theta3)*cos(theta5)*sin(theta2) + cos(theta2)*cos(theta3)*cos(theta4)*sin(theta5) - cos(theta4)*sin(theta2)*sin(theta3)*sin(theta5)) - (thetadot6*sin(theta6)*(cos(theta2)*cos(theta6)*sin(theta3)*sin(theta5) - cos(theta2)*cos(theta3)*sin(theta4)*sin(theta6) + cos(theta3)*cos(theta6)*sin(theta2)*sin(theta5) + sin(theta2)*sin(theta3)*sin(theta4)*sin(theta6) - cos(theta2)*cos(theta3)*cos(theta4)*cos(theta5)*cos(theta6) + cos(theta4)*cos(theta5)*cos(theta6)*sin(theta2)*sin(theta3)))/10 + (2*thetadot6*cos(theta6)*((cos(theta2)*sin(theta4)*sin(theta5))/5 + (2*sin(theta2)*sin(theta3)*sin(theta4))/5 - (2*cos(theta2)*cos(theta3)*sin(theta4))/5 + (2*cos(theta2)*cos(theta3)*cos(theta6)*sin(theta4))/5 + (2*cos(theta2)*cos(theta3)*sin(theta4)*sin(theta5))/5 - (2*cos(theta6)*sin(theta2)*sin(theta3)*sin(theta4))/5 + (2*cos(theta2)*sin(theta3)*sin(theta5)*sin(theta6))/5 + (2*cos(theta3)*sin(theta2)*sin(theta5)*sin(theta6))/5 - (2*sin(theta2)*sin(theta3)*sin(theta4)*sin(theta5))/5 - (2*cos(theta2)*cos(theta3)*cos(theta4)*cos(theta5)*sin(theta6))/5 + (2*cos(theta4)*cos(theta5)*sin(theta2)*sin(theta3)*sin(theta6))/5))/5 + (thetadot6*cos(theta6)*(cos(theta2)*cos(theta3)*cos(theta6)*sin(theta4) - cos(theta6)*sin(theta2)*sin(theta3)*sin(theta4) + cos(theta2)*sin(theta3)*sin(theta5)*sin(theta6) + cos(theta3)*sin(theta2)*sin(theta5)*sin(theta6) - cos(theta2)*cos(theta3)*cos(theta4)*cos(theta5)*sin(theta6) + cos(theta4)*cos(theta5)*sin(theta2)*sin(theta3)*sin(theta6)))/10 + cos(theta2 + theta3)*sin(theta4)*((sin(theta5)*(sin(theta4)*(thetadot2 + thetadot3) + thetadot1*cos(theta2 + theta3)*cos(theta4)))/10 + (cos(theta5)*(thetadot4 + thetadot1*sin(theta2 + theta3)))/10)) + sin(theta2)*((thetadot3*cos(theta3)*((2*cos(theta4)*cos(theta6))/5 + (2*cos(theta4)*sin(theta5))/5 + (2*cos(theta5)*sin(theta4)*sin(theta6))/5 - (2*cos(theta4)*cos(theta6)*sin(theta5))/5) - (2*thetadot3*cos(theta5)*sin(theta3)*(cos(theta6) - 1))/5)*((cos(theta2)*cos(theta4)*cos(theta6))/5 + (2*cos(theta2)*cos(theta5)*sin(theta3))/5 + (2*cos(theta3)*cos(theta5)*sin(theta2))/5 + (2*cos(theta2)*cos(theta3)*cos(theta4)*cos(theta6))/5 + (2*cos(theta2)*cos(theta3)*cos(theta4)*sin(theta5))/5 - (2*cos(theta2)*cos(theta5)*cos(theta6)*sin(theta3))/5 - (2*cos(theta3)*cos(theta5)*cos(theta6)*sin(theta2))/5 - (2*cos(theta4)*cos(theta6)*sin(theta2)*sin(theta3))/5 + (cos(theta2)*cos(theta5)*sin(theta4)*sin(theta6))/5 - (2*cos(theta4)*sin(theta2)*sin(theta3)*sin(theta5))/5 - (2*cos(theta2)*cos(theta3)*cos(theta4)*cos(theta6)*sin(theta5))/5 + (2*cos(theta2)*cos(theta3)*cos(theta5)*sin(theta4)*sin(theta6))/5 + (2*cos(theta4)*cos(theta6)*sin(theta2)*sin(theta3)*sin(theta5))/5 - (2*cos(theta5)*sin(theta2)*sin(theta3)*sin(theta4)*sin(theta6))/5) - (thetadot3*cos(theta3)*((sin(theta4)*sin(theta6))/10 + (cos(theta4)*cos(theta5)*cos(theta6))/10) - (thetadot3*cos(theta6)*sin(theta3)*sin(theta5))/10)*(cos(theta2)*cos(theta6)*sin(theta3)*sin(theta5) - cos(theta2)*cos(theta3)*sin(theta4)*sin(theta6) + cos(theta3)*cos(theta6)*sin(theta2)*sin(theta5) + sin(theta2)*sin(theta3)*sin(theta4)*sin(theta6) - cos(theta2)*cos(theta3)*cos(theta4)*cos(theta5)*cos(theta6) + cos(theta4)*cos(theta5)*cos(theta6)*sin(theta2)*sin(theta3)) - (thetadot2*cos(theta2))/10 - (thetadot3*cos(theta3)*((2*sin(theta4))/5 - (2*cos(theta6)*sin(theta4))/5 - (2*sin(theta4)*sin(theta5))/5 + (2*cos(theta4)*cos(theta5)*sin(theta6))/5) - (2*thetadot3*sin(theta3)*sin(theta5)*sin(theta6))/5)*((cos(theta2)*sin(theta4)*sin(theta5))/5 + (2*sin(theta2)*sin(theta3)*sin(theta4))/5 - (2*cos(theta2)*cos(theta3)*sin(theta4))/5 + (2*cos(theta2)*cos(theta3)*cos(theta6)*sin(theta4))/5 + (2*cos(theta2)*cos(theta3)*sin(theta4)*sin(theta5))/5 - (2*cos(theta6)*sin(theta2)*sin(theta3)*sin(theta4))/5 + (2*cos(theta2)*sin(theta3)*sin(theta5)*sin(theta6))/5 + (2*cos(theta3)*sin(theta2)*sin(theta5)*sin(theta6))/5 - (2*sin(theta2)*sin(theta3)*sin(theta4)*sin(theta5))/5 - (2*cos(theta2)*cos(theta3)*cos(theta4)*cos(theta5)*sin(theta6))/5 + (2*cos(theta4)*cos(theta5)*sin(theta2)*sin(theta3)*sin(theta6))/5) + 2*((thetadot3*cos(theta5)*sin(theta3))/10 + (thetadot3*cos(theta3)*cos(theta4)*sin(theta5))/10)*(cos(theta2)*cos(theta5)*sin(theta3) + cos(theta3)*cos(theta5)*sin(theta2) + cos(theta2)*cos(theta3)*cos(theta4)*sin(theta5) - cos(theta4)*sin(theta2)*sin(theta3)*sin(theta5)) + ((thetadot3*sin(theta3)*sin(theta5))/10 - (thetadot3*cos(theta3)*cos(theta4)*cos(theta5))/10)*(cos(theta2)*sin(theta3)*sin(theta5) + cos(theta3)*sin(theta2)*sin(theta5) - cos(theta2)*cos(theta3)*cos(theta4)*cos(theta5) + cos(theta4)*cos(theta5)*sin(theta2)*sin(theta3)) + (thetadot3*cos(theta3)*((cos(theta6)*sin(theta4))/10 - (cos(theta4)*cos(theta5)*sin(theta6))/10) + (thetadot3*sin(theta3)*sin(theta5)*sin(theta6))/10)*(cos(theta2)*cos(theta3)*cos(theta6)*sin(theta4) - cos(theta6)*sin(theta2)*sin(theta3)*sin(theta4) + cos(theta2)*sin(theta3)*sin(theta5)*sin(theta6) + cos(theta3)*sin(theta2)*sin(theta5)*sin(theta6) - cos(theta2)*cos(theta3)*cos(theta4)*cos(theta5)*sin(theta6) + cos(theta4)*cos(theta5)*sin(theta2)*sin(theta3)*sin(theta6)) + (thetadot3*cos(theta3)*((2*cos(theta4)*sin(theta5)*sin(theta6))/5 - (2*cos(theta4)*sin(theta6))/5 + (2*cos(theta5)*cos(theta6)*sin(theta4))/5) + (2*thetadot3*cos(theta5)*sin(theta3)*sin(theta6))/5)*((cos(theta2)*cos(theta5)*cos(theta6)*sin(theta4))/5 - (2*cos(theta2)*cos(theta3)*cos(theta4)*sin(theta6))/5 - (cos(theta2)*cos(theta4)*sin(theta6))/5 + (2*cos(theta2)*cos(theta5)*sin(theta3)*sin(theta6))/5 + (2*cos(theta3)*cos(theta5)*sin(theta2)*sin(theta6))/5 + (2*cos(theta4)*sin(theta2)*sin(theta3)*sin(theta6))/5 + (2*cos(theta2)*cos(theta3)*cos(theta5)*cos(theta6)*sin(theta4))/5 + (2*cos(theta2)*cos(theta3)*cos(theta4)*sin(theta5)*sin(theta6))/5 - (2*cos(theta5)*cos(theta6)*sin(theta2)*sin(theta3)*sin(theta4))/5 - (2*cos(theta4)*sin(theta2)*sin(theta3)*sin(theta5)*sin(theta6))/5) + (thetadot3*cos(theta2 + theta3)*cos(theta3))/10 + (thetadot3*sin(theta2 + theta3)*sin(theta3))/5 + (2*thetadot3*cos(theta3)*cos(theta4)^2*(2*cos(theta2 + theta3) + cos(theta2)))/25 + (thetadot3*cos(theta2 + theta3)*cos(theta3)*cos(theta4)^2)/10 + (thetadot3*cos(theta2 + theta3)*cos(theta3)*sin(theta4)^2)/5 + (thetadot3*cos(theta3)*cos(theta4)^2*(cos(theta2 + theta3) + cos(theta2)))/25 + (thetadot3*cos(theta3)*sin(theta4)^2*(cos(theta2 + theta3) + cos(theta2)))/25 + (2*thetadot3*cos(theta3)*cos(theta5)^2*sin(theta4)^2*(2*cos(theta2 + theta3) + cos(theta2)))/25 + (2*thetadot3*cos(theta3)*sin(theta4)^2*sin(theta5)^2*(2*cos(theta2 + theta3) + cos(theta2)))/25) + cos(theta2 + theta3)*cos(theta4)*((thetadot2*cos(theta2)*cos(theta4)*sin(theta3))/10 + (thetadot2*cos(theta3)*cos(theta4)*sin(theta2))/10) - cos(theta2 + theta3)*cos(theta4)*((thetadot5*cos(theta5)*(cos(theta2)*cos(theta5)*sin(theta3) + cos(theta3)*cos(theta5)*sin(theta2) + cos(theta2)*cos(theta3)*cos(theta4)*sin(theta5) - cos(theta4)*sin(theta2)*sin(theta3)*sin(theta5)))/5 - cos(theta2 + theta3)*sin(theta4)*(thetadot4/10 + (thetadot1*sin(theta2 + theta3))/10) - sin(theta2 + theta3)*((cos(theta4)*(thetadot2 + thetadot3))/10 - (thetadot1*cos(theta2 + theta3)*sin(theta4))/10) + (thetadot5*sin(theta5)*(cos(theta2)*sin(theta3)*sin(theta5) + cos(theta3)*sin(theta2)*sin(theta5) - cos(theta2)*cos(theta3)*cos(theta4)*cos(theta5) + cos(theta4)*cos(theta5)*sin(theta2)*sin(theta3)))/10 + (thetadot5*sin(theta5)*sin(theta6)*(cos(theta2)*cos(theta3)*cos(theta6)*sin(theta4) - cos(theta6)*sin(theta2)*sin(theta3)*sin(theta4) + cos(theta2)*sin(theta3)*sin(theta5)*sin(theta6) + cos(theta3)*sin(theta2)*sin(theta5)*sin(theta6) - cos(theta2)*cos(theta3)*cos(theta4)*cos(theta5)*sin(theta6) + cos(theta4)*cos(theta5)*sin(theta2)*sin(theta3)*sin(theta6)))/10 + (2*thetadot5*cos(theta5)*sin(theta6)*((cos(theta2)*cos(theta5)*cos(theta6)*sin(theta4))/5 - (2*cos(theta2)*cos(theta3)*cos(theta4)*sin(theta6))/5 - (cos(theta2)*cos(theta4)*sin(theta6))/5 + (2*cos(theta2)*cos(theta5)*sin(theta3)*sin(theta6))/5 + (2*cos(theta3)*cos(theta5)*sin(theta2)*sin(theta6))/5 + (2*cos(theta4)*sin(theta2)*sin(theta3)*sin(theta6))/5 + (2*cos(theta2)*cos(theta3)*cos(theta5)*cos(theta6)*sin(theta4))/5 + (2*cos(theta2)*cos(theta3)*cos(theta4)*sin(theta5)*sin(theta6))/5 - (2*cos(theta5)*cos(theta6)*sin(theta2)*sin(theta3)*sin(theta4))/5 - (2*cos(theta4)*sin(theta2)*sin(theta3)*sin(theta5)*sin(theta6))/5))/5 - thetadot5*cos(theta5)*((2*cos(theta6))/5 - 2/5)*((cos(theta2)*cos(theta4)*cos(theta6))/5 + (2*cos(theta2)*cos(theta5)*sin(theta3))/5 + (2*cos(theta3)*cos(theta5)*sin(theta2))/5 + (2*cos(theta2)*cos(theta3)*cos(theta4)*cos(theta6))/5 + (2*cos(theta2)*cos(theta3)*cos(theta4)*sin(theta5))/5 - (2*cos(theta2)*cos(theta5)*cos(theta6)*sin(theta3))/5 - (2*cos(theta3)*cos(theta5)*cos(theta6)*sin(theta2))/5 - (2*cos(theta4)*cos(theta6)*sin(theta2)*sin(theta3))/5 + (cos(theta2)*cos(theta5)*sin(theta4)*sin(theta6))/5 - (2*cos(theta4)*sin(theta2)*sin(theta3)*sin(theta5))/5 - (2*cos(theta2)*cos(theta3)*cos(theta4)*cos(theta6)*sin(theta5))/5 + (2*cos(theta2)*cos(theta3)*cos(theta5)*sin(theta4)*sin(theta6))/5 + (2*cos(theta4)*cos(theta6)*sin(theta2)*sin(theta3)*sin(theta5))/5 - (2*cos(theta5)*sin(theta2)*sin(theta3)*sin(theta4)*sin(theta6))/5) + (thetadot5*cos(theta6)*sin(theta5)*(cos(theta2)*cos(theta6)*sin(theta3)*sin(theta5) - cos(theta2)*cos(theta3)*sin(theta4)*sin(theta6) + cos(theta3)*cos(theta6)*sin(theta2)*sin(theta5) + sin(theta2)*sin(theta3)*sin(theta4)*sin(theta6) - cos(theta2)*cos(theta3)*cos(theta4)*cos(theta5)*cos(theta6) + cos(theta4)*cos(theta5)*cos(theta6)*sin(theta2)*sin(theta3)))/10 + (2*thetadot5*sin(theta5)*sin(theta6)*((cos(theta2)*sin(theta4)*sin(theta5))/5 + (2*sin(theta2)*sin(theta3)*sin(theta4))/5 - (2*cos(theta2)*cos(theta3)*sin(theta4))/5 + (2*cos(theta2)*cos(theta3)*cos(theta6)*sin(theta4))/5 + (2*cos(theta2)*cos(theta3)*sin(theta4)*sin(theta5))/5 - (2*cos(theta6)*sin(theta2)*sin(theta3)*sin(theta4))/5 + (2*cos(theta2)*sin(theta3)*sin(theta5)*sin(theta6))/5 + (2*cos(theta3)*sin(theta2)*sin(theta5)*sin(theta6))/5 - (2*sin(theta2)*sin(theta3)*sin(theta4)*sin(theta5))/5 - (2*cos(theta2)*cos(theta3)*cos(theta4)*cos(theta5)*sin(theta6))/5 + (2*cos(theta4)*cos(theta5)*sin(theta2)*sin(theta3)*sin(theta6))/5))/5) + cos(theta2 + theta3)*sin(theta4)*(sin(theta2 + theta3)*((sin(theta4)*(thetadot2 + thetadot3))/10 + (thetadot1*cos(theta2 + theta3)*cos(theta4))/10) - (thetadot5*cos(theta5)*((cos(theta2)*sin(theta4)*sin(theta5))/5 + (2*sin(theta2)*sin(theta3)*sin(theta4))/5 - (2*cos(theta2)*cos(theta3)*sin(theta4))/5 + (2*cos(theta2)*cos(theta3)*cos(theta6)*sin(theta4))/5 + (2*cos(theta2)*cos(theta3)*sin(theta4)*sin(theta5))/5 - (2*cos(theta6)*sin(theta2)*sin(theta3)*sin(theta4))/5 + (2*cos(theta2)*sin(theta3)*sin(theta5)*sin(theta6))/5 + (2*cos(theta3)*sin(theta2)*sin(theta5)*sin(theta6))/5 - (2*sin(theta2)*sin(theta3)*sin(theta4)*sin(theta5))/5 - (2*cos(theta2)*cos(theta3)*cos(theta4)*cos(theta5)*sin(theta6))/5 + (2*cos(theta4)*cos(theta5)*sin(theta2)*sin(theta3)*sin(theta6))/5))/5 - cos(theta2 + theta3)*cos(theta4)*(thetadot4/10 + (thetadot1*sin(theta2 + theta3))/10) + (thetadot5*cos(theta6)*sin(theta5)*((cos(theta2)*cos(theta5)*cos(theta6)*sin(theta4))/5 - (2*cos(theta2)*cos(theta3)*cos(theta4)*sin(theta6))/5 - (cos(theta2)*cos(theta4)*sin(theta6))/5 + (2*cos(theta2)*cos(theta5)*sin(theta3)*sin(theta6))/5 + (2*cos(theta3)*cos(theta5)*sin(theta2)*sin(theta6))/5 + (2*cos(theta4)*sin(theta2)*sin(theta3)*sin(theta6))/5 + (2*cos(theta2)*cos(theta3)*cos(theta5)*cos(theta6)*sin(theta4))/5 + (2*cos(theta2)*cos(theta3)*cos(theta4)*sin(theta5)*sin(theta6))/5 - (2*cos(theta5)*cos(theta6)*sin(theta2)*sin(theta3)*sin(theta4))/5 - (2*cos(theta4)*sin(theta2)*sin(theta3)*sin(theta5)*sin(theta6))/5))/5 + (thetadot5*sin(theta5)*sin(theta6)*((cos(theta2)*cos(theta4)*cos(theta6))/5 + (2*cos(theta2)*cos(theta5)*sin(theta3))/5 + (2*cos(theta3)*cos(theta5)*sin(theta2))/5 + (2*cos(theta2)*cos(theta3)*cos(theta4)*cos(theta6))/5 + (2*cos(theta2)*cos(theta3)*cos(theta4)*sin(theta5))/5 - (2*cos(theta2)*cos(theta5)*cos(theta6)*sin(theta3))/5 - (2*cos(theta3)*cos(theta5)*cos(theta6)*sin(theta2))/5 - (2*cos(theta4)*cos(theta6)*sin(theta2)*sin(theta3))/5 + (cos(theta2)*cos(theta5)*sin(theta4)*sin(theta6))/5 - (2*cos(theta4)*sin(theta2)*sin(theta3)*sin(theta5))/5 - (2*cos(theta2)*cos(theta3)*cos(theta4)*cos(theta6)*sin(theta5))/5 + (2*cos(theta2)*cos(theta3)*cos(theta5)*sin(theta4)*sin(theta6))/5 + (2*cos(theta4)*cos(theta6)*sin(theta2)*sin(theta3)*sin(theta5))/5 - (2*cos(theta5)*sin(theta2)*sin(theta3)*sin(theta4)*sin(theta6))/5))/5) + 2*cos(theta2 + theta3)*sin(theta4)*((thetadot2*cos(theta2)*sin(theta3)*sin(theta4))/10 + (thetadot2*cos(theta3)*sin(theta2)*sin(theta4))/10) + cos(theta2 + theta3)*sin(theta4)*(((cos(theta5)*(sin(theta4)*(thetadot2 + thetadot3) + thetadot1*cos(theta2 + theta3)*cos(theta4)))/10 - (sin(theta5)*(thetadot4 + thetadot1*sin(theta2 + theta3)))/10)*(cos(theta2)*cos(theta5)*sin(theta3) + cos(theta3)*cos(theta5)*sin(theta2) + cos(theta2)*cos(theta3)*cos(theta4)*sin(theta5) - cos(theta4)*sin(theta2)*sin(theta3)*sin(theta5)) + ((sin(theta5)*(sin(theta4)*(thetadot2 + thetadot3) + thetadot1*cos(theta2 + theta3)*cos(theta4)))/10 + (cos(theta5)*(thetadot4 + thetadot1*sin(theta2 + theta3)))/10)*(cos(theta2)*sin(theta3)*sin(theta5) + cos(theta3)*sin(theta2)*sin(theta5) - cos(theta2)*cos(theta3)*cos(theta4)*cos(theta5) + cos(theta4)*cos(theta5)*sin(theta2)*sin(theta3)) + (2*thetadot6*sin(theta6)*((cos(theta2)*sin(theta4)*sin(theta5))/5 + (2*sin(theta2)*sin(theta3)*sin(theta4))/5 - (2*cos(theta2)*cos(theta3)*sin(theta4))/5 + (2*cos(theta2)*cos(theta3)*cos(theta6)*sin(theta4))/5 + (2*cos(theta2)*cos(theta3)*sin(theta4)*sin(theta5))/5 - (2*cos(theta6)*sin(theta2)*sin(theta3)*sin(theta4))/5 + (2*cos(theta2)*sin(theta3)*sin(theta5)*sin(theta6))/5 + (2*cos(theta3)*sin(theta2)*sin(theta5)*sin(theta6))/5 - (2*sin(theta2)*sin(theta3)*sin(theta4)*sin(theta5))/5 - (2*cos(theta2)*cos(theta3)*cos(theta4)*cos(theta5)*sin(theta6))/5 + (2*cos(theta4)*cos(theta5)*sin(theta2)*sin(theta3)*sin(theta6))/5))/5 + (thetadot6*sin(theta6)*(cos(theta2)*cos(theta3)*cos(theta6)*sin(theta4) - cos(theta6)*sin(theta2)*sin(theta3)*sin(theta4) + cos(theta2)*sin(theta3)*sin(theta5)*sin(theta6) + cos(theta3)*sin(theta2)*sin(theta5)*sin(theta6) - cos(theta2)*cos(theta3)*cos(theta4)*cos(theta5)*sin(theta6) + cos(theta4)*cos(theta5)*sin(theta2)*sin(theta3)*sin(theta6)))/10 + (thetadot6*cos(theta6)*(cos(theta2)*cos(theta6)*sin(theta3)*sin(theta5) - cos(theta2)*cos(theta3)*sin(theta4)*sin(theta6) + cos(theta3)*cos(theta6)*sin(theta2)*sin(theta5) + sin(theta2)*sin(theta3)*sin(theta4)*sin(theta6) - cos(theta2)*cos(theta3)*cos(theta4)*cos(theta5)*cos(theta6) + cos(theta4)*cos(theta5)*cos(theta6)*sin(theta2)*sin(theta3)))/10) + (sin(theta4)*(cos(theta2 + theta3) + cos(theta2))*(sin(theta2 + theta3)*(sin(theta4)*(thetadot2/5 + thetadot3/5) + (thetadot1*cos(theta2 + theta3)*cos(theta4))/5 + (thetadot1*cos(theta2)*cos(theta4))/5 + (thetadot2*cos(theta3)*sin(theta4))/5) - thetadot5*cos(theta5)*((cos(theta2)*sin(theta4)*sin(theta5))/5 + (2*sin(theta2)*sin(theta3)*sin(theta4))/5 - (2*cos(theta2)*cos(theta3)*sin(theta4))/5 + (2*cos(theta2)*cos(theta3)*cos(theta6)*sin(theta4))/5 + (2*cos(theta2)*cos(theta3)*sin(theta4)*sin(theta5))/5 - (2*cos(theta6)*sin(theta2)*sin(theta3)*sin(theta4))/5 + (2*cos(theta2)*sin(theta3)*sin(theta5)*sin(theta6))/5 + (2*cos(theta3)*sin(theta2)*sin(theta5)*sin(theta6))/5 - (2*sin(theta2)*sin(theta3)*sin(theta4)*sin(theta5))/5 - (2*cos(theta2)*cos(theta3)*cos(theta4)*cos(theta5)*sin(theta6))/5 + (2*cos(theta4)*cos(theta5)*sin(theta2)*sin(theta3)*sin(theta6))/5) - (cos(theta4)*(thetadot4 + thetadot1*sin(theta2 + theta3))*(cos(theta2 + theta3) + cos(theta2)))/5 + thetadot5*cos(theta6)*sin(theta5)*((cos(theta2)*cos(theta5)*cos(theta6)*sin(theta4))/5 - (2*cos(theta2)*cos(theta3)*cos(theta4)*sin(theta6))/5 - (cos(theta2)*cos(theta4)*sin(theta6))/5 + (2*cos(theta2)*cos(theta5)*sin(theta3)*sin(theta6))/5 + (2*cos(theta3)*cos(theta5)*sin(theta2)*sin(theta6))/5 + (2*cos(theta4)*sin(theta2)*sin(theta3)*sin(theta6))/5 + (2*cos(theta2)*cos(theta3)*cos(theta5)*cos(theta6)*sin(theta4))/5 + (2*cos(theta2)*cos(theta3)*cos(theta4)*sin(theta5)*sin(theta6))/5 - (2*cos(theta5)*cos(theta6)*sin(theta2)*sin(theta3)*sin(theta4))/5 - (2*cos(theta4)*sin(theta2)*sin(theta3)*sin(theta5)*sin(theta6))/5) - (thetadot2*cos(theta2 + theta3)*sin(theta3)*sin(theta4))/5 + thetadot5*sin(theta5)*sin(theta6)*((cos(theta2)*cos(theta4)*cos(theta6))/5 + (2*cos(theta2)*cos(theta5)*sin(theta3))/5 + (2*cos(theta3)*cos(theta5)*sin(theta2))/5 + (2*cos(theta2)*cos(theta3)*cos(theta4)*cos(theta6))/5 + (2*cos(theta2)*cos(theta3)*cos(theta4)*sin(theta5))/5 - (2*cos(theta2)*cos(theta5)*cos(theta6)*sin(theta3))/5 - (2*cos(theta3)*cos(theta5)*cos(theta6)*sin(theta2))/5 - (2*cos(theta4)*cos(theta6)*sin(theta2)*sin(theta3))/5 + (cos(theta2)*cos(theta5)*sin(theta4)*sin(theta6))/5 - (2*cos(theta4)*sin(theta2)*sin(theta3)*sin(theta5))/5 - (2*cos(theta2)*cos(theta3)*cos(theta4)*cos(theta6)*sin(theta5))/5 + (2*cos(theta2)*cos(theta3)*cos(theta5)*sin(theta4)*sin(theta6))/5 + (2*cos(theta4)*cos(theta6)*sin(theta2)*sin(theta3)*sin(theta5))/5 - (2*cos(theta5)*sin(theta2)*sin(theta3)*sin(theta4)*sin(theta6))/5)))/5 + (cos(theta4)*(2*cos(theta2 + theta3) + cos(theta2))*((thetadot2*cos(theta4)*sin(theta2)*(2*cos(theta3) + 1))/5 + (2*thetadot2*cos(theta2)*cos(theta4)*sin(theta3))/5))/5 + (cos(theta4)*(cos(theta2 + theta3) + cos(theta2))*(sin(theta2 + theta3)*(cos(theta4)*(thetadot2/5 + thetadot3/5) - (thetadot1*cos(theta2 + theta3)*sin(theta4))/5 + (thetadot2*cos(theta3)*cos(theta4))/5 - (thetadot1*cos(theta2)*sin(theta4))/5) + (sin(theta4)*(thetadot4 + thetadot1*sin(theta2 + theta3))*(cos(theta2 + theta3) + cos(theta2)))/5 - (thetadot2*cos(theta2 + theta3)*cos(theta4)*sin(theta3))/5))/5 + (thetadot2*cos(theta2)*sin(theta2))/25 + (cos(theta4)*((thetadot2*cos(theta2)*cos(theta4)*sin(theta3))/5 + (thetadot2*cos(theta4)*sin(theta2)*(cos(theta3) + 1))/5)*(cos(theta2 + theta3) + cos(theta2)))/5 - cos(theta2 + theta3)*sin(theta2 + theta3)*(thetadot2/10 + thetadot3/10) + (cos(theta4)*(2*cos(theta2 + theta3) + cos(theta2))*((cos(theta2)*sin(theta3)*sin(theta5) + cos(theta3)*sin(theta2)*sin(theta5) - cos(theta2)*cos(theta3)*cos(theta4)*cos(theta5) + cos(theta4)*cos(theta5)*sin(theta2)*sin(theta3))*((thetadot2*cos(theta5)*sin(theta3))/5 + (2*thetadot2*cos(theta4)*sin(theta5))/5 + (2*thetadot3*cos(theta4)*sin(theta5))/5 + (thetadot2*cos(theta3)*cos(theta4)*sin(theta5))/5 - (thetadot1*cos(theta2)*sin(theta4)*sin(theta5))/5 - (2*thetadot1*cos(theta2)*cos(theta3)*sin(theta4)*sin(theta5))/5 + (2*thetadot1*sin(theta2)*sin(theta3)*sin(theta4)*sin(theta5))/5) + (cos(theta2)*cos(theta5)*sin(theta3) + cos(theta3)*cos(theta5)*sin(theta2) + cos(theta2)*cos(theta3)*cos(theta4)*sin(theta5) - cos(theta4)*sin(theta2)*sin(theta3)*sin(theta5))*((2*thetadot2*cos(theta4)*cos(theta5))/5 + (2*thetadot3*cos(theta4)*cos(theta5))/5 - (thetadot2*sin(theta3)*sin(theta5))/5 + (thetadot2*cos(theta3)*cos(theta4)*cos(theta5))/5 - (thetadot1*cos(theta2)*cos(theta5)*sin(theta4))/5 - (2*thetadot1*cos(theta2)*cos(theta3)*cos(theta5)*sin(theta4))/5 + (2*thetadot1*cos(theta5)*sin(theta2)*sin(theta3)*sin(theta4))/5) + thetadot6*cos(theta6)*((cos(theta2)*cos(theta5)*cos(theta6)*sin(theta4))/5 - (2*cos(theta2)*cos(theta3)*cos(theta4)*sin(theta6))/5 - (cos(theta2)*cos(theta4)*sin(theta6))/5 + (2*cos(theta2)*cos(theta5)*sin(theta3)*sin(theta6))/5 + (2*cos(theta3)*cos(theta5)*sin(theta2)*sin(theta6))/5 + (2*cos(theta4)*sin(theta2)*sin(theta3)*sin(theta6))/5 + (2*cos(theta2)*cos(theta3)*cos(theta5)*cos(theta6)*sin(theta4))/5 + (2*cos(theta2)*cos(theta3)*cos(theta4)*sin(theta5)*sin(theta6))/5 - (2*cos(theta5)*cos(theta6)*sin(theta2)*sin(theta3)*sin(theta4))/5 - (2*cos(theta4)*sin(theta2)*sin(theta3)*sin(theta5)*sin(theta6))/5) + thetadot6*sin(theta6)*((cos(theta2)*cos(theta4)*cos(theta6))/5 + (2*cos(theta2)*cos(theta5)*sin(theta3))/5 + (2*cos(theta3)*cos(theta5)*sin(theta2))/5 + (2*cos(theta2)*cos(theta3)*cos(theta4)*cos(theta6))/5 + (2*cos(theta2)*cos(theta3)*cos(theta4)*sin(theta5))/5 - (2*cos(theta2)*cos(theta5)*cos(theta6)*sin(theta3))/5 - (2*cos(theta3)*cos(theta5)*cos(theta6)*sin(theta2))/5 - (2*cos(theta4)*cos(theta6)*sin(theta2)*sin(theta3))/5 + (cos(theta2)*cos(theta5)*sin(theta4)*sin(theta6))/5 - (2*cos(theta4)*sin(theta2)*sin(theta3)*sin(theta5))/5 - (2*cos(theta2)*cos(theta3)*cos(theta4)*cos(theta6)*sin(theta5))/5 + (2*cos(theta2)*cos(theta3)*cos(theta5)*sin(theta4)*sin(theta6))/5 + (2*cos(theta4)*cos(theta6)*sin(theta2)*sin(theta3)*sin(theta5))/5 - (2*cos(theta5)*sin(theta2)*sin(theta3)*sin(theta4)*sin(theta6))/5) + (cos(theta5)*sin(theta4)*(2*cos(theta2 + theta3) + cos(theta2))*(sin(theta5)*(sin(theta4)*(thetadot2 + thetadot3) + thetadot1*cos(theta2 + theta3)*cos(theta4)) + cos(theta5)*(thetadot4 + thetadot1*sin(theta2 + theta3))))/5 - (sin(theta4)*sin(theta5)*(2*cos(theta2 + theta3) + cos(theta2))*(cos(theta5)*(sin(theta4)*(thetadot2 + thetadot3) + thetadot1*cos(theta2 + theta3)*cos(theta4)) - sin(theta5)*(thetadot4 + thetadot1*sin(theta2 + theta3))))/5))/5 + (sin(theta4)*((thetadot2*cos(theta2)*sin(theta3)*sin(theta4))/5 + (thetadot2*sin(theta2)*sin(theta4)*(cos(theta3) + 1))/5)*(cos(theta2 + theta3) + cos(theta2)))/5 + (cos(theta5)*sin(theta4)*(2*cos(theta2 + theta3) + cos(theta2))*((thetadot2*cos(theta5)*sin(theta2)*sin(theta4)*(2*cos(theta3) + 1))/5 + (2*thetadot2*cos(theta2)*cos(theta5)*sin(theta3)*sin(theta4))/5))/5 + (sin(theta4)*sin(theta5)*(2*cos(theta2 + theta3) + cos(theta2))*((thetadot2*sin(theta2)*sin(theta4)*sin(theta5)*(2*cos(theta3) + 1))/5 + (2*thetadot2*cos(theta2)*sin(theta3)*sin(theta4)*sin(theta5))/5))/5 + (sin(theta4)*sin(theta5)*(2*cos(theta2 + theta3) + cos(theta2))*((cos(theta2)*sin(theta3)*sin(theta5) + cos(theta3)*sin(theta2)*sin(theta5) - cos(theta2)*cos(theta3)*cos(theta4)*cos(theta5) + cos(theta4)*cos(theta5)*sin(theta2)*sin(theta3))*((2*thetadot2*sin(theta4))/5 + (2*thetadot3*sin(theta4))/5 + (thetadot1*cos(theta2)*cos(theta4))/5 + (thetadot2*cos(theta3)*sin(theta4))/5 + (2*thetadot1*cos(theta2)*cos(theta3)*cos(theta4))/5 - (2*thetadot1*cos(theta4)*sin(theta2)*sin(theta3))/5) + (cos(theta4)*(2*cos(theta2 + theta3) + cos(theta2))*(cos(theta5)*(sin(theta4)*(thetadot2 + thetadot3) + thetadot1*cos(theta2 + theta3)*cos(theta4)) - sin(theta5)*(thetadot4 + thetadot1*sin(theta2 + theta3))))/5 + cos(theta2 + theta3)*sin(theta4)*((2*thetadot2*cos(theta4)*cos(theta5))/5 + (2*thetadot3*cos(theta4)*cos(theta5))/5 - (thetadot2*sin(theta3)*sin(theta5))/5 + (thetadot2*cos(theta3)*cos(theta4)*cos(theta5))/5 - (thetadot1*cos(theta2)*cos(theta5)*sin(theta4))/5 - (2*thetadot1*cos(theta2)*cos(theta3)*cos(theta5)*sin(theta4))/5 + (2*thetadot1*cos(theta5)*sin(theta2)*sin(theta3)*sin(theta4))/5) - (cos(theta5)*sin(theta4)*(2*cos(theta2 + theta3) + cos(theta2))*(thetadot5 + cos(theta4)*(thetadot2 + thetadot3) - thetadot1*cos(theta2 + theta3)*sin(theta4)))/5))/5 + (cos(theta5)*sin(theta4)*(2*cos(theta2 + theta3) + cos(theta2))*((cos(theta2)*cos(theta5)*sin(theta3) + cos(theta3)*cos(theta5)*sin(theta2) + cos(theta2)*cos(theta3)*cos(theta4)*sin(theta5) - cos(theta4)*sin(theta2)*sin(theta3)*sin(theta5))*((2*thetadot2*sin(theta4))/5 + (2*thetadot3*sin(theta4))/5 + (thetadot1*cos(theta2)*cos(theta4))/5 + (thetadot2*cos(theta3)*sin(theta4))/5 + (2*thetadot1*cos(theta2)*cos(theta3)*cos(theta4))/5 - (2*thetadot1*cos(theta4)*sin(theta2)*sin(theta3))/5) - (cos(theta4)*(2*cos(theta2 + theta3) + cos(theta2))*(sin(theta5)*(sin(theta4)*(thetadot2 + thetadot3) + thetadot1*cos(theta2 + theta3)*cos(theta4)) + cos(theta5)*(thetadot4 + thetadot1*sin(theta2 + theta3))))/5 + thetadot6*sin(theta6)*((cos(theta2)*cos(theta5)*cos(theta6)*sin(theta4))/5 - (2*cos(theta2)*cos(theta3)*cos(theta4)*sin(theta6))/5 - (cos(theta2)*cos(theta4)*sin(theta6))/5 + (2*cos(theta2)*cos(theta5)*sin(theta3)*sin(theta6))/5 + (2*cos(theta3)*cos(theta5)*sin(theta2)*sin(theta6))/5 + (2*cos(theta4)*sin(theta2)*sin(theta3)*sin(theta6))/5 + (2*cos(theta2)*cos(theta3)*cos(theta5)*cos(theta6)*sin(theta4))/5 + (2*cos(theta2)*cos(theta3)*cos(theta4)*sin(theta5)*sin(theta6))/5 - (2*cos(theta5)*cos(theta6)*sin(theta2)*sin(theta3)*sin(theta4))/5 - (2*cos(theta4)*sin(theta2)*sin(theta3)*sin(theta5)*sin(theta6))/5) - thetadot6*cos(theta6)*((cos(theta2)*cos(theta4)*cos(theta6))/5 + (2*cos(theta2)*cos(theta5)*sin(theta3))/5 + (2*cos(theta3)*cos(theta5)*sin(theta2))/5 + (2*cos(theta2)*cos(theta3)*cos(theta4)*cos(theta6))/5 + (2*cos(theta2)*cos(theta3)*cos(theta4)*sin(theta5))/5 - (2*cos(theta2)*cos(theta5)*cos(theta6)*sin(theta3))/5 - (2*cos(theta3)*cos(theta5)*cos(theta6)*sin(theta2))/5 - (2*cos(theta4)*cos(theta6)*sin(theta2)*sin(theta3))/5 + (cos(theta2)*cos(theta5)*sin(theta4)*sin(theta6))/5 - (2*cos(theta4)*sin(theta2)*sin(theta3)*sin(theta5))/5 - (2*cos(theta2)*cos(theta3)*cos(theta4)*cos(theta6)*sin(theta5))/5 + (2*cos(theta2)*cos(theta3)*cos(theta5)*sin(theta4)*sin(theta6))/5 + (2*cos(theta4)*cos(theta6)*sin(theta2)*sin(theta3)*sin(theta5))/5 - (2*cos(theta5)*sin(theta2)*sin(theta3)*sin(theta4)*sin(theta6))/5) - cos(theta2 + theta3)*sin(theta4)*((thetadot2*cos(theta5)*sin(theta3))/5 + (2*thetadot2*cos(theta4)*sin(theta5))/5 + (2*thetadot3*cos(theta4)*sin(theta5))/5 + (thetadot2*cos(theta3)*cos(theta4)*sin(theta5))/5 - (thetadot1*cos(theta2)*sin(theta4)*sin(theta5))/5 - (2*thetadot1*cos(theta2)*cos(theta3)*sin(theta4)*sin(theta5))/5 + (2*thetadot1*sin(theta2)*sin(theta3)*sin(theta4)*sin(theta5))/5) + (sin(theta4)*sin(theta5)*(2*cos(theta2 + theta3) + cos(theta2))*(thetadot5 + cos(theta4)*(thetadot2 + thetadot3) - thetadot1*cos(theta2 + theta3)*sin(theta4)))/5))/5) + thetadot5*(((2*cos(theta6))/5 - 2/5)*((sin(theta6)*(cos(theta5)*(sin(theta4)*(thetadot2 + thetadot3) + thetadot1*cos(theta2 + theta3)*cos(theta4)) - sin(theta5)*(thetadot4 + thetadot1*sin(theta2 + theta3))) + cos(theta6)*(thetadot5 + cos(theta4)*(thetadot2 + thetadot3) - thetadot1*cos(theta2 + theta3)*sin(theta4)))*((cos(theta2)*cos(theta5)*cos(theta6)*sin(theta4))/5 - (2*cos(theta2)*cos(theta3)*cos(theta4)*sin(theta6))/5 - (cos(theta2)*cos(theta4)*sin(theta6))/5 + (2*cos(theta2)*cos(theta5)*sin(theta3)*sin(theta6))/5 + (2*cos(theta3)*cos(theta5)*sin(theta2)*sin(theta6))/5 + (2*cos(theta4)*sin(theta2)*sin(theta3)*sin(theta6))/5 + (2*cos(theta2)*cos(theta3)*cos(theta5)*cos(theta6)*sin(theta4))/5 + (2*cos(theta2)*cos(theta3)*cos(theta4)*sin(theta5)*sin(theta6))/5 - (2*cos(theta5)*cos(theta6)*sin(theta2)*sin(theta3)*sin(theta4))/5 - (2*cos(theta4)*sin(theta2)*sin(theta3)*sin(theta5)*sin(theta6))/5) + (sin(theta6)*(thetadot5 + cos(theta4)*(thetadot2 + thetadot3) - thetadot1*cos(theta2 + theta3)*sin(theta4)) - cos(theta6)*(cos(theta5)*(sin(theta4)*(thetadot2 + thetadot3) + thetadot1*cos(theta2 + theta3)*cos(theta4)) - sin(theta5)*(thetadot4 + thetadot1*sin(theta2 + theta3))))*((cos(theta2)*cos(theta4)*cos(theta6))/5 + (2*cos(theta2)*cos(theta5)*sin(theta3))/5 + (2*cos(theta3)*cos(theta5)*sin(theta2))/5 + (2*cos(theta2)*cos(theta3)*cos(theta4)*cos(theta6))/5 + (2*cos(theta2)*cos(theta3)*cos(theta4)*sin(theta5))/5 - (2*cos(theta2)*cos(theta5)*cos(theta6)*sin(theta3))/5 - (2*cos(theta3)*cos(theta5)*cos(theta6)*sin(theta2))/5 - (2*cos(theta4)*cos(theta6)*sin(theta2)*sin(theta3))/5 + (cos(theta2)*cos(theta5)*sin(theta4)*sin(theta6))/5 - (2*cos(theta4)*sin(theta2)*sin(theta3)*sin(theta5))/5 - (2*cos(theta2)*cos(theta3)*cos(theta4)*cos(theta6)*sin(theta5))/5 + (2*cos(theta2)*cos(theta3)*cos(theta5)*sin(theta4)*sin(theta6))/5 + (2*cos(theta4)*cos(theta6)*sin(theta2)*sin(theta3)*sin(theta5))/5 - (2*cos(theta5)*sin(theta2)*sin(theta3)*sin(theta4)*sin(theta6))/5) - ((sin(theta6)*(2*thetadot2*sin(theta4) + 2*thetadot3*sin(theta4) + thetadot1*cos(theta2)*cos(theta4) + thetadot2*cos(theta3)*sin(theta4) + 2*thetadot1*cos(theta2)*cos(theta3)*cos(theta4) - 2*thetadot1*cos(theta4)*sin(theta2)*sin(theta3)))/5 + (cos(theta6)*(2*thetadot2*cos(theta4)*cos(theta5) + 2*thetadot3*cos(theta4)*cos(theta5) - thetadot2*sin(theta3)*sin(theta5) + thetadot2*cos(theta3)*cos(theta4)*cos(theta5) - thetadot1*cos(theta2)*cos(theta5)*sin(theta4) - 2*thetadot1*cos(theta2)*cos(theta3)*cos(theta5)*sin(theta4) + 2*thetadot1*cos(theta5)*sin(theta2)*sin(theta3)*sin(theta4)))/5 - (2*sin(theta6)*(sin(theta5)*(thetadot2*sin(theta4) + thetadot3*sin(theta4) + thetadot1*cos(theta2 + theta3)*cos(theta4)) + cos(theta5)*(thetadot4 + thetadot1*sin(theta2 + theta3))))/5)*(cos(theta2)*cos(theta3)*cos(theta6)*sin(theta4) - cos(theta6)*sin(theta2)*sin(theta3)*sin(theta4) + cos(theta2)*sin(theta3)*sin(theta5)*sin(theta6) + cos(theta3)*sin(theta2)*sin(theta5)*sin(theta6) - cos(theta2)*cos(theta3)*cos(theta4)*cos(theta5)*sin(theta6) + cos(theta4)*cos(theta5)*sin(theta2)*sin(theta3)*sin(theta6)) - ((2*thetadot6)/5 - (sin(theta5)*(thetadot2*sin(theta4) + thetadot3*sin(theta4) + thetadot1*cos(theta2 + theta3)*cos(theta4)) + cos(theta5)*(thetadot4 + thetadot1*sin(theta2 + theta3)))*((2*cos(theta6))/5 - 2/5) - (sin(theta6)*(2*thetadot2*cos(theta4)*cos(theta5) + 2*thetadot3*cos(theta4)*cos(theta5) - thetadot2*sin(theta3)*sin(theta5) + thetadot2*cos(theta3)*cos(theta4)*cos(theta5) - thetadot1*cos(theta2)*cos(theta5)*sin(theta4) - 2*thetadot1*cos(theta2)*cos(theta3)*cos(theta5)*sin(theta4) + 2*thetadot1*cos(theta5)*sin(theta2)*sin(theta3)*sin(theta4)))/5 + (cos(theta6)*(2*thetadot2*sin(theta4) + 2*thetadot3*sin(theta4) + thetadot1*cos(theta2)*cos(theta4) + thetadot2*cos(theta3)*sin(theta4) + 2*thetadot1*cos(theta2)*cos(theta3)*cos(theta4) - 2*thetadot1*cos(theta4)*sin(theta2)*sin(theta3)))/5)*(cos(theta2)*cos(theta6)*sin(theta3)*sin(theta5) - cos(theta2)*cos(theta3)*sin(theta4)*sin(theta6) + cos(theta3)*cos(theta6)*sin(theta2)*sin(theta5) + sin(theta2)*sin(theta3)*sin(theta4)*sin(theta6) - cos(theta2)*cos(theta3)*cos(theta4)*cos(theta5)*cos(theta6) + cos(theta4)*cos(theta5)*cos(theta6)*sin(theta2)*sin(theta3))) - sin(theta6)*((thetadot6/10 + (sin(theta5)*(sin(theta4)*(thetadot2 + thetadot3) + thetadot1*cos(theta2 + theta3)*cos(theta4)))/10 + (cos(theta5)*(thetadot4 + thetadot1*sin(theta2 + theta3)))/10)*(cos(theta2)*cos(theta3)*cos(theta6)*sin(theta4) - cos(theta6)*sin(theta2)*sin(theta3)*sin(theta4) + cos(theta2)*sin(theta3)*sin(theta5)*sin(theta6) + cos(theta3)*sin(theta2)*sin(theta5)*sin(theta6) - cos(theta2)*cos(theta3)*cos(theta4)*cos(theta5)*sin(theta6) + cos(theta4)*cos(theta5)*sin(theta2)*sin(theta3)*sin(theta6)) + ((sin(theta6)*(cos(theta5)*(sin(theta4)*(thetadot2 + thetadot3) + thetadot1*cos(theta2 + theta3)*cos(theta4)) - sin(theta5)*(thetadot4 + thetadot1*sin(theta2 + theta3))))/10 + (cos(theta6)*(thetadot5 + cos(theta4)*(thetadot2 + thetadot3) - thetadot1*cos(theta2 + theta3)*sin(theta4)))/10)*(cos(theta2)*cos(theta5)*sin(theta3) + cos(theta3)*cos(theta5)*sin(theta2) + cos(theta2)*cos(theta3)*cos(theta4)*sin(theta5) - cos(theta4)*sin(theta2)*sin(theta3)*sin(theta5))) - cos(theta6)*((thetadot6/10 + (sin(theta5)*(sin(theta4)*(thetadot2 + thetadot3) + thetadot1*cos(theta2 + theta3)*cos(theta4)))/10 + (cos(theta5)*(thetadot4 + thetadot1*sin(theta2 + theta3)))/10)*(cos(theta2)*cos(theta6)*sin(theta3)*sin(theta5) - cos(theta2)*cos(theta3)*sin(theta4)*sin(theta6) + cos(theta3)*cos(theta6)*sin(theta2)*sin(theta5) + sin(theta2)*sin(theta3)*sin(theta4)*sin(theta6) - cos(theta2)*cos(theta3)*cos(theta4)*cos(theta5)*cos(theta6) + cos(theta4)*cos(theta5)*cos(theta6)*sin(theta2)*sin(theta3)) - ((sin(theta6)*(thetadot5 + cos(theta4)*(thetadot2 + thetadot3) - thetadot1*cos(theta2 + theta3)*sin(theta4)))/10 - (cos(theta6)*(cos(theta5)*(sin(theta4)*(thetadot2 + thetadot3) + thetadot1*cos(theta2 + theta3)*cos(theta4)) - sin(theta5)*(thetadot4 + thetadot1*sin(theta2 + theta3))))/10)*(cos(theta2)*cos(theta5)*sin(theta3) + cos(theta3)*cos(theta5)*sin(theta2) + cos(theta2)*cos(theta3)*cos(theta4)*sin(theta5) - cos(theta4)*sin(theta2)*sin(theta3)*sin(theta5))) + ((cos(theta5)*(sin(theta4)*(thetadot2 + thetadot3) + thetadot1*cos(theta2 + theta3)*cos(theta4)))/10 - (sin(theta5)*(thetadot4 + thetadot1*sin(theta2 + theta3)))/10)*(cos(theta2)*cos(theta5)*sin(theta3) + cos(theta3)*cos(theta5)*sin(theta2) + cos(theta2)*cos(theta3)*cos(theta4)*sin(theta5) - cos(theta4)*sin(theta2)*sin(theta3)*sin(theta5)) + ((sin(theta5)*(sin(theta4)*(thetadot2 + thetadot3) + thetadot1*cos(theta2 + theta3)*cos(theta4)))/10 + (cos(theta5)*(thetadot4 + thetadot1*sin(theta2 + theta3)))/10)*(cos(theta2)*sin(theta3)*sin(theta5) + cos(theta3)*sin(theta2)*sin(theta5) - cos(theta2)*cos(theta3)*cos(theta4)*cos(theta5) + cos(theta4)*cos(theta5)*sin(theta2)*sin(theta3)) + (2*thetadot6*sin(theta6)*((cos(theta2)*sin(theta4)*sin(theta5))/5 + (2*sin(theta2)*sin(theta3)*sin(theta4))/5 - (2*cos(theta2)*cos(theta3)*sin(theta4))/5 + (2*cos(theta2)*cos(theta3)*cos(theta6)*sin(theta4))/5 + (2*cos(theta2)*cos(theta3)*sin(theta4)*sin(theta5))/5 - (2*cos(theta6)*sin(theta2)*sin(theta3)*sin(theta4))/5 + (2*cos(theta2)*sin(theta3)*sin(theta5)*sin(theta6))/5 + (2*cos(theta3)*sin(theta2)*sin(theta5)*sin(theta6))/5 - (2*sin(theta2)*sin(theta3)*sin(theta4)*sin(theta5))/5 - (2*cos(theta2)*cos(theta3)*cos(theta4)*cos(theta5)*sin(theta6))/5 + (2*cos(theta4)*cos(theta5)*sin(theta2)*sin(theta3)*sin(theta6))/5))/5 + (thetadot6*sin(theta6)*(cos(theta2)*cos(theta3)*cos(theta6)*sin(theta4) - cos(theta6)*sin(theta2)*sin(theta3)*sin(theta4) + cos(theta2)*sin(theta3)*sin(theta5)*sin(theta6) + cos(theta3)*sin(theta2)*sin(theta5)*sin(theta6) - cos(theta2)*cos(theta3)*cos(theta4)*cos(theta5)*sin(theta6) + cos(theta4)*cos(theta5)*sin(theta2)*sin(theta3)*sin(theta6)))/10 + (thetadot6*cos(theta6)*(cos(theta2)*cos(theta6)*sin(theta3)*sin(theta5) - cos(theta2)*cos(theta3)*sin(theta4)*sin(theta6) + cos(theta3)*cos(theta6)*sin(theta2)*sin(theta5) + sin(theta2)*sin(theta3)*sin(theta4)*sin(theta6) - cos(theta2)*cos(theta3)*cos(theta4)*cos(theta5)*cos(theta6) + cos(theta4)*cos(theta5)*cos(theta6)*sin(theta2)*sin(theta3)))/10) + thetadot6*((2*((sin(theta6)*(2*thetadot2*sin(theta4) + 2*thetadot3*sin(theta4) + thetadot1*cos(theta2)*cos(theta4) + thetadot2*cos(theta3)*sin(theta4) + 2*thetadot1*cos(theta2)*cos(theta3)*cos(theta4) - 2*thetadot1*cos(theta4)*sin(theta2)*sin(theta3)))/5 + (cos(theta6)*(2*thetadot2*cos(theta4)*cos(theta5) + 2*thetadot3*cos(theta4)*cos(theta5) - thetadot2*sin(theta3)*sin(theta5) + thetadot2*cos(theta3)*cos(theta4)*cos(theta5) - thetadot1*cos(theta2)*cos(theta5)*sin(theta4) - 2*thetadot1*cos(theta2)*cos(theta3)*cos(theta5)*sin(theta4) + 2*thetadot1*cos(theta5)*sin(theta2)*sin(theta3)*sin(theta4)))/5 - (2*sin(theta6)*(sin(theta5)*(thetadot2*sin(theta4) + thetadot3*sin(theta4) + thetadot1*cos(theta2 + theta3)*cos(theta4)) + cos(theta5)*(thetadot4 + thetadot1*sin(theta2 + theta3))))/5)*(cos(theta2)*cos(theta5)*sin(theta3) + cos(theta3)*cos(theta5)*sin(theta2) + cos(theta2)*cos(theta3)*cos(theta4)*sin(theta5) - cos(theta4)*sin(theta2)*sin(theta3)*sin(theta5)))/5 + (2*((sin(theta5)*(thetadot2*cos(theta4) + thetadot3*cos(theta4) - thetadot1*cos(theta2 + theta3)*sin(theta4)))/5 + sin(theta5)*((thetadot2*cos(theta4))/5 + (thetadot3*cos(theta4))/5 - (thetadot1*cos(theta2 + theta3)*sin(theta4))/5 + (thetadot2*cos(theta3)*cos(theta4))/5 - (thetadot1*cos(theta2)*sin(theta4))/5) + ((2*cos(theta6))/5 - 2/5)*(thetadot5 + thetadot2*cos(theta4) + thetadot3*cos(theta4) - thetadot1*cos(theta2 + theta3)*sin(theta4)) + (2*sin(theta6)*(cos(theta5)*(thetadot2*sin(theta4) + thetadot3*sin(theta4) + thetadot1*cos(theta2 + theta3)*cos(theta4)) - sin(theta5)*(thetadot4 + thetadot1*sin(theta2 + theta3))))/5 + (thetadot2*cos(theta5)*sin(theta3))/5)*(cos(theta2)*cos(theta6)*sin(theta3)*sin(theta5) - cos(theta2)*cos(theta3)*sin(theta4)*sin(theta6) + cos(theta3)*cos(theta6)*sin(theta2)*sin(theta5) + sin(theta2)*sin(theta3)*sin(theta4)*sin(theta6) - cos(theta2)*cos(theta3)*cos(theta4)*cos(theta5)*cos(theta6) + cos(theta4)*cos(theta5)*cos(theta6)*sin(theta2)*sin(theta3)))/5 + ((sin(theta6)*(cos(theta5)*(sin(theta4)*(thetadot2 + thetadot3) + thetadot1*cos(theta2 + theta3)*cos(theta4)) - sin(theta5)*(thetadot4 + thetadot1*sin(theta2 + theta3))))/10 + (cos(theta6)*(thetadot5 + cos(theta4)*(thetadot2 + thetadot3) - thetadot1*cos(theta2 + theta3)*sin(theta4)))/10)*(cos(theta2)*cos(theta6)*sin(theta3)*sin(theta5) - cos(theta2)*cos(theta3)*sin(theta4)*sin(theta6) + cos(theta3)*cos(theta6)*sin(theta2)*sin(theta5) + sin(theta2)*sin(theta3)*sin(theta4)*sin(theta6) - cos(theta2)*cos(theta3)*cos(theta4)*cos(theta5)*cos(theta6) + cos(theta4)*cos(theta5)*cos(theta6)*sin(theta2)*sin(theta3)) + (2*(sin(theta6)*(thetadot5 + cos(theta4)*(thetadot2 + thetadot3) - thetadot1*cos(theta2 + theta3)*sin(theta4)) - cos(theta6)*(cos(theta5)*(sin(theta4)*(thetadot2 + thetadot3) + thetadot1*cos(theta2 + theta3)*cos(theta4)) - sin(theta5)*(thetadot4 + thetadot1*sin(theta2 + theta3))))*((cos(theta2)*sin(theta4)*sin(theta5))/5 + (2*sin(theta2)*sin(theta3)*sin(theta4))/5 - (2*cos(theta2)*cos(theta3)*sin(theta4))/5 + (2*cos(theta2)*cos(theta3)*cos(theta6)*sin(theta4))/5 + (2*cos(theta2)*cos(theta3)*sin(theta4)*sin(theta5))/5 - (2*cos(theta6)*sin(theta2)*sin(theta3)*sin(theta4))/5 + (2*cos(theta2)*sin(theta3)*sin(theta5)*sin(theta6))/5 + (2*cos(theta3)*sin(theta2)*sin(theta5)*sin(theta6))/5 - (2*sin(theta2)*sin(theta3)*sin(theta4)*sin(theta5))/5 - (2*cos(theta2)*cos(theta3)*cos(theta4)*cos(theta5)*sin(theta6))/5 + (2*cos(theta4)*cos(theta5)*sin(theta2)*sin(theta3)*sin(theta6))/5))/5 + ((sin(theta6)*(thetadot5 + cos(theta4)*(thetadot2 + thetadot3) - thetadot1*cos(theta2 + theta3)*sin(theta4)))/10 - (cos(theta6)*(cos(theta5)*(sin(theta4)*(thetadot2 + thetadot3) + thetadot1*cos(theta2 + theta3)*cos(theta4)) - sin(theta5)*(thetadot4 + thetadot1*sin(theta2 + theta3))))/10)*(cos(theta2)*cos(theta3)*cos(theta6)*sin(theta4) - cos(theta6)*sin(theta2)*sin(theta3)*sin(theta4) + cos(theta2)*sin(theta3)*sin(theta5)*sin(theta6) + cos(theta3)*sin(theta2)*sin(theta5)*sin(theta6) - cos(theta2)*cos(theta3)*cos(theta4)*cos(theta5)*sin(theta6) + cos(theta4)*cos(theta5)*sin(theta2)*sin(theta3)*sin(theta6)) + (2*(thetadot6 + sin(theta5)*(sin(theta4)*(thetadot2 + thetadot3) + thetadot1*cos(theta2 + theta3)*cos(theta4)) + cos(theta5)*(thetadot4 + thetadot1*sin(theta2 + theta3)))*((cos(theta2)*cos(theta5)*cos(theta6)*sin(theta4))/5 - (2*cos(theta2)*cos(theta3)*cos(theta4)*sin(theta6))/5 - (cos(theta2)*cos(theta4)*sin(theta6))/5 + (2*cos(theta2)*cos(theta5)*sin(theta3)*sin(theta6))/5 + (2*cos(theta3)*cos(theta5)*sin(theta2)*sin(theta6))/5 + (2*cos(theta4)*sin(theta2)*sin(theta3)*sin(theta6))/5 + (2*cos(theta2)*cos(theta3)*cos(theta5)*cos(theta6)*sin(theta4))/5 + (2*cos(theta2)*cos(theta3)*cos(theta4)*sin(theta5)*sin(theta6))/5 - (2*cos(theta5)*cos(theta6)*sin(theta2)*sin(theta3)*sin(theta4))/5 - (2*cos(theta4)*sin(theta2)*sin(theta3)*sin(theta5)*sin(theta6))/5))/5) + thetadot2*(((cos(theta5)*sin(theta3))/5 + (2*cos(theta4)*sin(theta5))/5 + (cos(theta3)*cos(theta4)*sin(theta5))/5)*((cos(theta2)*sin(theta3)*sin(theta5) + cos(theta3)*sin(theta2)*sin(theta5) - cos(theta2)*cos(theta3)*cos(theta4)*cos(theta5) + cos(theta4)*cos(theta5)*sin(theta2)*sin(theta3))*((2*thetadot2*sin(theta4))/5 + (2*thetadot3*sin(theta4))/5 + (thetadot1*cos(theta2)*cos(theta4))/5 + (thetadot2*cos(theta3)*sin(theta4))/5 + (2*thetadot1*cos(theta2)*cos(theta3)*cos(theta4))/5 - (2*thetadot1*cos(theta4)*sin(theta2)*sin(theta3))/5) + (cos(theta4)*(2*cos(theta2 + theta3) + cos(theta2))*(cos(theta5)*(sin(theta4)*(thetadot2 + thetadot3) + thetadot1*cos(theta2 + theta3)*cos(theta4)) - sin(theta5)*(thetadot4 + thetadot1*sin(theta2 + theta3))))/5 + cos(theta2 + theta3)*sin(theta4)*((2*thetadot2*cos(theta4)*cos(theta5))/5 + (2*thetadot3*cos(theta4)*cos(theta5))/5 - (thetadot2*sin(theta3)*sin(theta5))/5 + (thetadot2*cos(theta3)*cos(theta4)*cos(theta5))/5 - (thetadot1*cos(theta2)*cos(theta5)*sin(theta4))/5 - (2*thetadot1*cos(theta2)*cos(theta3)*cos(theta5)*sin(theta4))/5 + (2*thetadot1*cos(theta5)*sin(theta2)*sin(theta3)*sin(theta4))/5) - (cos(theta5)*sin(theta4)*(2*cos(theta2 + theta3) + cos(theta2))*(thetadot5 + cos(theta4)*(thetadot2 + thetadot3) - thetadot1*cos(theta2 + theta3)*sin(theta4)))/5) - ((thetadot4*sin(theta4)*sin(theta6))/10 + (thetadot4*cos(theta4)*cos(theta5)*cos(theta6))/10)*(cos(theta2)*cos(theta6)*sin(theta3)*sin(theta5) - cos(theta2)*cos(theta3)*sin(theta4)*sin(theta6) + cos(theta3)*cos(theta6)*sin(theta2)*sin(theta5) + sin(theta2)*sin(theta3)*sin(theta4)*sin(theta6) - cos(theta2)*cos(theta3)*cos(theta4)*cos(theta5)*cos(theta6) + cos(theta4)*cos(theta5)*cos(theta6)*sin(theta2)*sin(theta3)) + (((sin(theta6)*(2*thetadot2*sin(theta4) + 2*thetadot3*sin(theta4) + thetadot1*cos(theta2)*cos(theta4) + thetadot2*cos(theta3)*sin(theta4) + 2*thetadot1*cos(theta2)*cos(theta3)*cos(theta4) - 2*thetadot1*cos(theta4)*sin(theta2)*sin(theta3)))/5 + (cos(theta6)*(2*thetadot2*cos(theta4)*cos(theta5) + 2*thetadot3*cos(theta4)*cos(theta5) - thetadot2*sin(theta3)*sin(theta5) + thetadot2*cos(theta3)*cos(theta4)*cos(theta5) - thetadot1*cos(theta2)*cos(theta5)*sin(theta4) - 2*thetadot1*cos(theta2)*cos(theta3)*cos(theta5)*sin(theta4) + 2*thetadot1*cos(theta5)*sin(theta2)*sin(theta3)*sin(theta4)))/5 - (2*sin(theta6)*(sin(theta5)*(thetadot2*sin(theta4) + thetadot3*sin(theta4) + thetadot1*cos(theta2 + theta3)*cos(theta4)) + cos(theta5)*(thetadot4 + thetadot1*sin(theta2 + theta3))))/5)*(cos(theta2)*cos(theta5)*sin(theta3) + cos(theta3)*cos(theta5)*sin(theta2) + cos(theta2)*cos(theta3)*cos(theta4)*sin(theta5) - cos(theta4)*sin(theta2)*sin(theta3)*sin(theta5)) + ((sin(theta5)*(thetadot2*cos(theta4) + thetadot3*cos(theta4) - thetadot1*cos(theta2 + theta3)*sin(theta4)))/5 + sin(theta5)*((thetadot2*cos(theta4))/5 + (thetadot3*cos(theta4))/5 - (thetadot1*cos(theta2 + theta3)*sin(theta4))/5 + (thetadot2*cos(theta3)*cos(theta4))/5 - (thetadot1*cos(theta2)*sin(theta4))/5) + ((2*cos(theta6))/5 - 2/5)*(thetadot5 + thetadot2*cos(theta4) + thetadot3*cos(theta4) - thetadot1*cos(theta2 + theta3)*sin(theta4)) + (2*sin(theta6)*(cos(theta5)*(thetadot2*sin(theta4) + thetadot3*sin(theta4) + thetadot1*cos(theta2 + theta3)*cos(theta4)) - sin(theta5)*(thetadot4 + thetadot1*sin(theta2 + theta3))))/5 + (thetadot2*cos(theta5)*sin(theta3))/5)*(cos(theta2)*cos(theta6)*sin(theta3)*sin(theta5) - cos(theta2)*cos(theta3)*sin(theta4)*sin(theta6) + cos(theta3)*cos(theta6)*sin(theta2)*sin(theta5) + sin(theta2)*sin(theta3)*sin(theta4)*sin(theta6) - cos(theta2)*cos(theta3)*cos(theta4)*cos(theta5)*cos(theta6) + cos(theta4)*cos(theta5)*cos(theta6)*sin(theta2)*sin(theta3)) + (sin(theta6)*(thetadot5 + cos(theta4)*(thetadot2 + thetadot3) - thetadot1*cos(theta2 + theta3)*sin(theta4)) - cos(theta6)*(cos(theta5)*(sin(theta4)*(thetadot2 + thetadot3) + thetadot1*cos(theta2 + theta3)*cos(theta4)) - sin(theta5)*(thetadot4 + thetadot1*sin(theta2 + theta3))))*((cos(theta2)*sin(theta4)*sin(theta5))/5 + (2*sin(theta2)*sin(theta3)*sin(theta4))/5 - (2*cos(theta2)*cos(theta3)*sin(theta4))/5 + (2*cos(theta2)*cos(theta3)*cos(theta6)*sin(theta4))/5 + (2*cos(theta2)*cos(theta3)*sin(theta4)*sin(theta5))/5 - (2*cos(theta6)*sin(theta2)*sin(theta3)*sin(theta4))/5 + (2*cos(theta2)*sin(theta3)*sin(theta5)*sin(theta6))/5 + (2*cos(theta3)*sin(theta2)*sin(theta5)*sin(theta6))/5 - (2*sin(theta2)*sin(theta3)*sin(theta4)*sin(theta5))/5 - (2*cos(theta2)*cos(theta3)*cos(theta4)*cos(theta5)*sin(theta6))/5 + (2*cos(theta4)*cos(theta5)*sin(theta2)*sin(theta3)*sin(theta6))/5) + (thetadot6 + sin(theta5)*(sin(theta4)*(thetadot2 + thetadot3) + thetadot1*cos(theta2 + theta3)*cos(theta4)) + cos(theta5)*(thetadot4 + thetadot1*sin(theta2 + theta3)))*((cos(theta2)*cos(theta5)*cos(theta6)*sin(theta4))/5 - (2*cos(theta2)*cos(theta3)*cos(theta4)*sin(theta6))/5 - (cos(theta2)*cos(theta4)*sin(theta6))/5 + (2*cos(theta2)*cos(theta5)*sin(theta3)*sin(theta6))/5 + (2*cos(theta3)*cos(theta5)*sin(theta2)*sin(theta6))/5 + (2*cos(theta4)*sin(theta2)*sin(theta3)*sin(theta6))/5 + (2*cos(theta2)*cos(theta3)*cos(theta5)*cos(theta6)*sin(theta4))/5 + (2*cos(theta2)*cos(theta3)*cos(theta4)*sin(theta5)*sin(theta6))/5 - (2*cos(theta5)*cos(theta6)*sin(theta2)*sin(theta3)*sin(theta4))/5 - (2*cos(theta4)*sin(theta2)*sin(theta3)*sin(theta5)*sin(theta6))/5))*((2*cos(theta6)*sin(theta4))/5 + (2*sin(theta4)*sin(theta5))/5 - (2*cos(theta6)*sin(theta4)*sin(theta5))/5 + (sin(theta3)*sin(theta5)*sin(theta6))/5 + (cos(theta3)*cos(theta6)*sin(theta4))/5 - (2*cos(theta4)*cos(theta5)*sin(theta6))/5 - (cos(theta3)*cos(theta4)*cos(theta5)*sin(theta6))/5) - ((thetadot3*cos(theta3)*cos(theta5))/5 - (thetadot3*cos(theta4)*sin(theta3)*sin(theta5))/5)*((cos(theta2)*sin(theta4)*sin(theta5))/5 + (2*sin(theta2)*sin(theta3)*sin(theta4))/5 - (2*cos(theta2)*cos(theta3)*sin(theta4))/5 + (2*cos(theta2)*cos(theta3)*cos(theta6)*sin(theta4))/5 + (2*cos(theta2)*cos(theta3)*sin(theta4)*sin(theta5))/5 - (2*cos(theta6)*sin(theta2)*sin(theta3)*sin(theta4))/5 + (2*cos(theta2)*sin(theta3)*sin(theta5)*sin(theta6))/5 + (2*cos(theta3)*sin(theta2)*sin(theta5)*sin(theta6))/5 - (2*sin(theta2)*sin(theta3)*sin(theta4)*sin(theta5))/5 - (2*cos(theta2)*cos(theta3)*cos(theta4)*cos(theta5)*sin(theta6))/5 + (2*cos(theta4)*cos(theta5)*sin(theta2)*sin(theta3)*sin(theta6))/5) + (cos(theta3)*((thetadot4*cos(theta4)*cos(theta6) + thetadot4*cos(theta5)*sin(theta4)*sin(theta6))*((cos(theta2)*cos(theta4)*cos(theta6))/5 + (2*cos(theta2)*cos(theta5)*sin(theta3))/5 + (2*cos(theta3)*cos(theta5)*sin(theta2))/5 + (2*cos(theta2)*cos(theta3)*cos(theta4)*cos(theta6))/5 + (2*cos(theta2)*cos(theta3)*cos(theta4)*sin(theta5))/5 - (2*cos(theta2)*cos(theta5)*cos(theta6)*sin(theta3))/5 - (2*cos(theta3)*cos(theta5)*cos(theta6)*sin(theta2))/5 - (2*cos(theta4)*cos(theta6)*sin(theta2)*sin(theta3))/5 + (cos(theta2)*cos(theta5)*sin(theta4)*sin(theta6))/5 - (2*cos(theta4)*sin(theta2)*sin(theta3)*sin(theta5))/5 - (2*cos(theta2)*cos(theta3)*cos(theta4)*cos(theta6)*sin(theta5))/5 + (2*cos(theta2)*cos(theta3)*cos(theta5)*sin(theta4)*sin(theta6))/5 + (2*cos(theta4)*cos(theta6)*sin(theta2)*sin(theta3)*sin(theta5))/5 - (2*cos(theta5)*sin(theta2)*sin(theta3)*sin(theta4)*sin(theta6))/5) - (thetadot4*cos(theta4)*sin(theta6) - thetadot4*cos(theta5)*cos(theta6)*sin(theta4))*((cos(theta2)*cos(theta5)*cos(theta6)*sin(theta4))/5 - (2*cos(theta2)*cos(theta3)*cos(theta4)*sin(theta6))/5 - (cos(theta2)*cos(theta4)*sin(theta6))/5 + (2*cos(theta2)*cos(theta5)*sin(theta3)*sin(theta6))/5 + (2*cos(theta3)*cos(theta5)*sin(theta2)*sin(theta6))/5 + (2*cos(theta4)*sin(theta2)*sin(theta3)*sin(theta6))/5 + (2*cos(theta2)*cos(theta3)*cos(theta5)*cos(theta6)*sin(theta4))/5 + (2*cos(theta2)*cos(theta3)*cos(theta4)*sin(theta5)*sin(theta6))/5 - (2*cos(theta5)*cos(theta6)*sin(theta2)*sin(theta3)*sin(theta4))/5 - (2*cos(theta4)*sin(theta2)*sin(theta3)*sin(theta5)*sin(theta6))/5) + (thetadot4*cos(theta4)^2*(2*cos(theta2 + theta3) + cos(theta2)))/5 + (thetadot4*cos(theta4)^2*(cos(theta2 + theta3) + cos(theta2)))/5 + (thetadot4*sin(theta4)^2*(cos(theta2 + theta3) + cos(theta2)))/5 + (thetadot4*cos(theta5)^2*sin(theta4)^2*(2*cos(theta2 + theta3) + cos(theta2)))/5 + (thetadot4*sin(theta4)^2*sin(theta5)^2*(2*cos(theta2 + theta3) + cos(theta2)))/5 + thetadot4*sin(theta4)*sin(theta5)*((cos(theta2)*sin(theta4)*sin(theta5))/5 + (2*sin(theta2)*sin(theta3)*sin(theta4))/5 - (2*cos(theta2)*cos(theta3)*sin(theta4))/5 + (2*cos(theta2)*cos(theta3)*cos(theta6)*sin(theta4))/5 + (2*cos(theta2)*cos(theta3)*sin(theta4)*sin(theta5))/5 - (2*cos(theta6)*sin(theta2)*sin(theta3)*sin(theta4))/5 + (2*cos(theta2)*sin(theta3)*sin(theta5)*sin(theta6))/5 + (2*cos(theta3)*sin(theta2)*sin(theta5)*sin(theta6))/5 - (2*sin(theta2)*sin(theta3)*sin(theta4)*sin(theta5))/5 - (2*cos(theta2)*cos(theta3)*cos(theta4)*cos(theta5)*sin(theta6))/5 + (2*cos(theta4)*cos(theta5)*sin(theta2)*sin(theta3)*sin(theta6))/5)))/5 + ((thetadot4*cos(theta6)*sin(theta4))/10 - (thetadot4*cos(theta4)*cos(theta5)*sin(theta6))/10)*(cos(theta2)*cos(theta3)*cos(theta6)*sin(theta4) - cos(theta6)*sin(theta2)*sin(theta3)*sin(theta4) + cos(theta2)*sin(theta3)*sin(theta5)*sin(theta6) + cos(theta3)*sin(theta2)*sin(theta5)*sin(theta6) - cos(theta2)*cos(theta3)*cos(theta4)*cos(theta5)*sin(theta6) + cos(theta4)*cos(theta5)*sin(theta2)*sin(theta3)*sin(theta6)) + ((2*cos(theta4)*cos(theta5))/5 - (sin(theta3)*sin(theta5))/5 + (cos(theta3)*cos(theta4)*cos(theta5))/5)*((cos(theta2)*cos(theta5)*sin(theta3) + cos(theta3)*cos(theta5)*sin(theta2) + cos(theta2)*cos(theta3)*cos(theta4)*sin(theta5) - cos(theta4)*sin(theta2)*sin(theta3)*sin(theta5))*((2*thetadot2*sin(theta4))/5 + (2*thetadot3*sin(theta4))/5 + (thetadot1*cos(theta2)*cos(theta4))/5 + (thetadot2*cos(theta3)*sin(theta4))/5 + (2*thetadot1*cos(theta2)*cos(theta3)*cos(theta4))/5 - (2*thetadot1*cos(theta4)*sin(theta2)*sin(theta3))/5) - (cos(theta4)*(2*cos(theta2 + theta3) + cos(theta2))*(sin(theta5)*(sin(theta4)*(thetadot2 + thetadot3) + thetadot1*cos(theta2 + theta3)*cos(theta4)) + cos(theta5)*(thetadot4 + thetadot1*sin(theta2 + theta3))))/5 + thetadot6*sin(theta6)*((cos(theta2)*cos(theta5)*cos(theta6)*sin(theta4))/5 - (2*cos(theta2)*cos(theta3)*cos(theta4)*sin(theta6))/5 - (cos(theta2)*cos(theta4)*sin(theta6))/5 + (2*cos(theta2)*cos(theta5)*sin(theta3)*sin(theta6))/5 + (2*cos(theta3)*cos(theta5)*sin(theta2)*sin(theta6))/5 + (2*cos(theta4)*sin(theta2)*sin(theta3)*sin(theta6))/5 + (2*cos(theta2)*cos(theta3)*cos(theta5)*cos(theta6)*sin(theta4))/5 + (2*cos(theta2)*cos(theta3)*cos(theta4)*sin(theta5)*sin(theta6))/5 - (2*cos(theta5)*cos(theta6)*sin(theta2)*sin(theta3)*sin(theta4))/5 - (2*cos(theta4)*sin(theta2)*sin(theta3)*sin(theta5)*sin(theta6))/5) - thetadot6*cos(theta6)*((cos(theta2)*cos(theta4)*cos(theta6))/5 + (2*cos(theta2)*cos(theta5)*sin(theta3))/5 + (2*cos(theta3)*cos(theta5)*sin(theta2))/5 + (2*cos(theta2)*cos(theta3)*cos(theta4)*cos(theta6))/5 + (2*cos(theta2)*cos(theta3)*cos(theta4)*sin(theta5))/5 - (2*cos(theta2)*cos(theta5)*cos(theta6)*sin(theta3))/5 - (2*cos(theta3)*cos(theta5)*cos(theta6)*sin(theta2))/5 - (2*cos(theta4)*cos(theta6)*sin(theta2)*sin(theta3))/5 + (cos(theta2)*cos(theta5)*sin(theta4)*sin(theta6))/5 - (2*cos(theta4)*sin(theta2)*sin(theta3)*sin(theta5))/5 - (2*cos(theta2)*cos(theta3)*cos(theta4)*cos(theta6)*sin(theta5))/5 + (2*cos(theta2)*cos(theta3)*cos(theta5)*sin(theta4)*sin(theta6))/5 + (2*cos(theta4)*cos(theta6)*sin(theta2)*sin(theta3)*sin(theta5))/5 - (2*cos(theta5)*sin(theta2)*sin(theta3)*sin(theta4)*sin(theta6))/5) - cos(theta2 + theta3)*sin(theta4)*((thetadot2*cos(theta5)*sin(theta3))/5 + (2*thetadot2*cos(theta4)*sin(theta5))/5 + (2*thetadot3*cos(theta4)*sin(theta5))/5 + (thetadot2*cos(theta3)*cos(theta4)*sin(theta5))/5 - (thetadot1*cos(theta2)*sin(theta4)*sin(theta5))/5 - (2*thetadot1*cos(theta2)*cos(theta3)*sin(theta4)*sin(theta5))/5 + (2*thetadot1*sin(theta2)*sin(theta3)*sin(theta4)*sin(theta5))/5) + (sin(theta4)*sin(theta5)*(2*cos(theta2 + theta3) + cos(theta2))*(thetadot5 + cos(theta4)*(thetadot2 + thetadot3) - thetadot1*cos(theta2 + theta3)*sin(theta4)))/5) + ((thetadot4*cos(theta4)*cos(theta6))/5 + thetadot4*cos(theta4)*(cos(theta6)/5 + (2*sin(theta5))/5 - (2*cos(theta6)*sin(theta5))/5) + (2*thetadot4*cos(theta5)*sin(theta4)*sin(theta6))/5)*((cos(theta2)*cos(theta4)*cos(theta6))/5 + (2*cos(theta2)*cos(theta5)*sin(theta3))/5 + (2*cos(theta3)*cos(theta5)*sin(theta2))/5 + (2*cos(theta2)*cos(theta3)*cos(theta4)*cos(theta6))/5 + (2*cos(theta2)*cos(theta3)*cos(theta4)*sin(theta5))/5 - (2*cos(theta2)*cos(theta5)*cos(theta6)*sin(theta3))/5 - (2*cos(theta3)*cos(theta5)*cos(theta6)*sin(theta2))/5 - (2*cos(theta4)*cos(theta6)*sin(theta2)*sin(theta3))/5 + (cos(theta2)*cos(theta5)*sin(theta4)*sin(theta6))/5 - (2*cos(theta4)*sin(theta2)*sin(theta3)*sin(theta5))/5 - (2*cos(theta2)*cos(theta3)*cos(theta4)*cos(theta6)*sin(theta5))/5 + (2*cos(theta2)*cos(theta3)*cos(theta5)*sin(theta4)*sin(theta6))/5 + (2*cos(theta4)*cos(theta6)*sin(theta2)*sin(theta3)*sin(theta5))/5 - (2*cos(theta5)*sin(theta2)*sin(theta3)*sin(theta4)*sin(theta6))/5) - ((thetadot3*sin(theta3)*(cos(theta6)*sin(theta4) - cos(theta4)*cos(theta5)*sin(theta6)))/5 - (thetadot3*cos(theta3)*sin(theta5)*sin(theta6))/5)*((cos(theta2)*cos(theta4)*cos(theta6))/5 + (2*cos(theta2)*cos(theta5)*sin(theta3))/5 + (2*cos(theta3)*cos(theta5)*sin(theta2))/5 + (2*cos(theta2)*cos(theta3)*cos(theta4)*cos(theta6))/5 + (2*cos(theta2)*cos(theta3)*cos(theta4)*sin(theta5))/5 - (2*cos(theta2)*cos(theta5)*cos(theta6)*sin(theta3))/5 - (2*cos(theta3)*cos(theta5)*cos(theta6)*sin(theta2))/5 - (2*cos(theta4)*cos(theta6)*sin(theta2)*sin(theta3))/5 + (cos(theta2)*cos(theta5)*sin(theta4)*sin(theta6))/5 - (2*cos(theta4)*sin(theta2)*sin(theta3)*sin(theta5))/5 - (2*cos(theta2)*cos(theta3)*cos(theta4)*cos(theta6)*sin(theta5))/5 + (2*cos(theta2)*cos(theta3)*cos(theta5)*sin(theta4)*sin(theta6))/5 + (2*cos(theta4)*cos(theta6)*sin(theta2)*sin(theta3)*sin(theta5))/5 - (2*cos(theta5)*sin(theta2)*sin(theta3)*sin(theta4)*sin(theta6))/5) + cos(theta4)*(sin(theta2 + theta3)*((sin(theta4)*(thetadot2 + thetadot3))/10 + (thetadot1*cos(theta2 + theta3)*cos(theta4))/10) - (thetadot5*cos(theta5)*((cos(theta2)*sin(theta4)*sin(theta5))/5 + (2*sin(theta2)*sin(theta3)*sin(theta4))/5 - (2*cos(theta2)*cos(theta3)*sin(theta4))/5 + (2*cos(theta2)*cos(theta3)*cos(theta6)*sin(theta4))/5 + (2*cos(theta2)*cos(theta3)*sin(theta4)*sin(theta5))/5 - (2*cos(theta6)*sin(theta2)*sin(theta3)*sin(theta4))/5 + (2*cos(theta2)*sin(theta3)*sin(theta5)*sin(theta6))/5 + (2*cos(theta3)*sin(theta2)*sin(theta5)*sin(theta6))/5 - (2*sin(theta2)*sin(theta3)*sin(theta4)*sin(theta5))/5 - (2*cos(theta2)*cos(theta3)*cos(theta4)*cos(theta5)*sin(theta6))/5 + (2*cos(theta4)*cos(theta5)*sin(theta2)*sin(theta3)*sin(theta6))/5))/5 - cos(theta2 + theta3)*cos(theta4)*(thetadot4/10 + (thetadot1*sin(theta2 + theta3))/10) + (thetadot5*cos(theta6)*sin(theta5)*((cos(theta2)*cos(theta5)*cos(theta6)*sin(theta4))/5 - (2*cos(theta2)*cos(theta3)*cos(theta4)*sin(theta6))/5 - (cos(theta2)*cos(theta4)*sin(theta6))/5 + (2*cos(theta2)*cos(theta5)*sin(theta3)*sin(theta6))/5 + (2*cos(theta3)*cos(theta5)*sin(theta2)*sin(theta6))/5 + (2*cos(theta4)*sin(theta2)*sin(theta3)*sin(theta6))/5 + (2*cos(theta2)*cos(theta3)*cos(theta5)*cos(theta6)*sin(theta4))/5 + (2*cos(theta2)*cos(theta3)*cos(theta4)*sin(theta5)*sin(theta6))/5 - (2*cos(theta5)*cos(theta6)*sin(theta2)*sin(theta3)*sin(theta4))/5 - (2*cos(theta4)*sin(theta2)*sin(theta3)*sin(theta5)*sin(theta6))/5))/5 + (thetadot5*sin(theta5)*sin(theta6)*((cos(theta2)*cos(theta4)*cos(theta6))/5 + (2*cos(theta2)*cos(theta5)*sin(theta3))/5 + (2*cos(theta3)*cos(theta5)*sin(theta2))/5 + (2*cos(theta2)*cos(theta3)*cos(theta4)*cos(theta6))/5 + (2*cos(theta2)*cos(theta3)*cos(theta4)*sin(theta5))/5 - (2*cos(theta2)*cos(theta5)*cos(theta6)*sin(theta3))/5 - (2*cos(theta3)*cos(theta5)*cos(theta6)*sin(theta2))/5 - (2*cos(theta4)*cos(theta6)*sin(theta2)*sin(theta3))/5 + (cos(theta2)*cos(theta5)*sin(theta4)*sin(theta6))/5 - (2*cos(theta4)*sin(theta2)*sin(theta3)*sin(theta5))/5 - (2*cos(theta2)*cos(theta3)*cos(theta4)*cos(theta6)*sin(theta5))/5 + (2*cos(theta2)*cos(theta3)*cos(theta5)*sin(theta4)*sin(theta6))/5 + (2*cos(theta4)*cos(theta6)*sin(theta2)*sin(theta3)*sin(theta5))/5 - (2*cos(theta5)*sin(theta2)*sin(theta3)*sin(theta4)*sin(theta6))/5))/5) + ((thetadot4*cos(theta4)*sin(theta6)*(2*sin(theta5) - 1))/5 - (thetadot4*cos(theta4)*sin(theta6))/5 + (2*thetadot4*cos(theta5)*cos(theta6)*sin(theta4))/5)*((cos(theta2)*cos(theta5)*cos(theta6)*sin(theta4))/5 - (2*cos(theta2)*cos(theta3)*cos(theta4)*sin(theta6))/5 - (cos(theta2)*cos(theta4)*sin(theta6))/5 + (2*cos(theta2)*cos(theta5)*sin(theta3)*sin(theta6))/5 + (2*cos(theta3)*cos(theta5)*sin(theta2)*sin(theta6))/5 + (2*cos(theta4)*sin(theta2)*sin(theta3)*sin(theta6))/5 + (2*cos(theta2)*cos(theta3)*cos(theta5)*cos(theta6)*sin(theta4))/5 + (2*cos(theta2)*cos(theta3)*cos(theta4)*sin(theta5)*sin(theta6))/5 - (2*cos(theta5)*cos(theta6)*sin(theta2)*sin(theta3)*sin(theta4))/5 - (2*cos(theta4)*sin(theta2)*sin(theta3)*sin(theta5)*sin(theta6))/5) + sin(theta4)*((thetadot5*cos(theta5)*(cos(theta2)*cos(theta5)*sin(theta3) + cos(theta3)*cos(theta5)*sin(theta2) + cos(theta2)*cos(theta3)*cos(theta4)*sin(theta5) - cos(theta4)*sin(theta2)*sin(theta3)*sin(theta5)))/5 - cos(theta2 + theta3)*sin(theta4)*(thetadot4/10 + (thetadot1*sin(theta2 + theta3))/10) - sin(theta2 + theta3)*((cos(theta4)*(thetadot2 + thetadot3))/10 - (thetadot1*cos(theta2 + theta3)*sin(theta4))/10) + (thetadot5*sin(theta5)*(cos(theta2)*sin(theta3)*sin(theta5) + cos(theta3)*sin(theta2)*sin(theta5) - cos(theta2)*cos(theta3)*cos(theta4)*cos(theta5) + cos(theta4)*cos(theta5)*sin(theta2)*sin(theta3)))/10 + (thetadot5*sin(theta5)*sin(theta6)*(cos(theta2)*cos(theta3)*cos(theta6)*sin(theta4) - cos(theta6)*sin(theta2)*sin(theta3)*sin(theta4) + cos(theta2)*sin(theta3)*sin(theta5)*sin(theta6) + cos(theta3)*sin(theta2)*sin(theta5)*sin(theta6) - cos(theta2)*cos(theta3)*cos(theta4)*cos(theta5)*sin(theta6) + cos(theta4)*cos(theta5)*sin(theta2)*sin(theta3)*sin(theta6)))/10 + (2*thetadot5*cos(theta5)*sin(theta6)*((cos(theta2)*cos(theta5)*cos(theta6)*sin(theta4))/5 - (2*cos(theta2)*cos(theta3)*cos(theta4)*sin(theta6))/5 - (cos(theta2)*cos(theta4)*sin(theta6))/5 + (2*cos(theta2)*cos(theta5)*sin(theta3)*sin(theta6))/5 + (2*cos(theta3)*cos(theta5)*sin(theta2)*sin(theta6))/5 + (2*cos(theta4)*sin(theta2)*sin(theta3)*sin(theta6))/5 + (2*cos(theta2)*cos(theta3)*cos(theta5)*cos(theta6)*sin(theta4))/5 + (2*cos(theta2)*cos(theta3)*cos(theta4)*sin(theta5)*sin(theta6))/5 - (2*cos(theta5)*cos(theta6)*sin(theta2)*sin(theta3)*sin(theta4))/5 - (2*cos(theta4)*sin(theta2)*sin(theta3)*sin(theta5)*sin(theta6))/5))/5 - thetadot5*cos(theta5)*((2*cos(theta6))/5 - 2/5)*((cos(theta2)*cos(theta4)*cos(theta6))/5 + (2*cos(theta2)*cos(theta5)*sin(theta3))/5 + (2*cos(theta3)*cos(theta5)*sin(theta2))/5 + (2*cos(theta2)*cos(theta3)*cos(theta4)*cos(theta6))/5 + (2*cos(theta2)*cos(theta3)*cos(theta4)*sin(theta5))/5 - (2*cos(theta2)*cos(theta5)*cos(theta6)*sin(theta3))/5 - (2*cos(theta3)*cos(theta5)*cos(theta6)*sin(theta2))/5 - (2*cos(theta4)*cos(theta6)*sin(theta2)*sin(theta3))/5 + (cos(theta2)*cos(theta5)*sin(theta4)*sin(theta6))/5 - (2*cos(theta4)*sin(theta2)*sin(theta3)*sin(theta5))/5 - (2*cos(theta2)*cos(theta3)*cos(theta4)*cos(theta6)*sin(theta5))/5 + (2*cos(theta2)*cos(theta3)*cos(theta5)*sin(theta4)*sin(theta6))/5 + (2*cos(theta4)*cos(theta6)*sin(theta2)*sin(theta3)*sin(theta5))/5 - (2*cos(theta5)*sin(theta2)*sin(theta3)*sin(theta4)*sin(theta6))/5) + (thetadot5*cos(theta6)*sin(theta5)*(cos(theta2)*cos(theta6)*sin(theta3)*sin(theta5) - cos(theta2)*cos(theta3)*sin(theta4)*sin(theta6) + cos(theta3)*cos(theta6)*sin(theta2)*sin(theta5) + sin(theta2)*sin(theta3)*sin(theta4)*sin(theta6) - cos(theta2)*cos(theta3)*cos(theta4)*cos(theta5)*cos(theta6) + cos(theta4)*cos(theta5)*cos(theta6)*sin(theta2)*sin(theta3)))/10 + (2*thetadot5*sin(theta5)*sin(theta6)*((cos(theta2)*sin(theta4)*sin(theta5))/5 + (2*sin(theta2)*sin(theta3)*sin(theta4))/5 - (2*cos(theta2)*cos(theta3)*sin(theta4))/5 + (2*cos(theta2)*cos(theta3)*cos(theta6)*sin(theta4))/5 + (2*cos(theta2)*cos(theta3)*sin(theta4)*sin(theta5))/5 - (2*cos(theta6)*sin(theta2)*sin(theta3)*sin(theta4))/5 + (2*cos(theta2)*sin(theta3)*sin(theta5)*sin(theta6))/5 + (2*cos(theta3)*sin(theta2)*sin(theta5)*sin(theta6))/5 - (2*sin(theta2)*sin(theta3)*sin(theta4)*sin(theta5))/5 - (2*cos(theta2)*cos(theta3)*cos(theta4)*cos(theta5)*sin(theta6))/5 + (2*cos(theta4)*cos(theta5)*sin(theta2)*sin(theta3)*sin(theta6))/5))/5) + cos(theta4)*(((cos(theta5)*(sin(theta4)*(thetadot2 + thetadot3) + thetadot1*cos(theta2 + theta3)*cos(theta4)))/10 - (sin(theta5)*(thetadot4 + thetadot1*sin(theta2 + theta3)))/10)*(cos(theta2)*cos(theta5)*sin(theta3) + cos(theta3)*cos(theta5)*sin(theta2) + cos(theta2)*cos(theta3)*cos(theta4)*sin(theta5) - cos(theta4)*sin(theta2)*sin(theta3)*sin(theta5)) + ((sin(theta5)*(sin(theta4)*(thetadot2 + thetadot3) + thetadot1*cos(theta2 + theta3)*cos(theta4)))/10 + (cos(theta5)*(thetadot4 + thetadot1*sin(theta2 + theta3)))/10)*(cos(theta2)*sin(theta3)*sin(theta5) + cos(theta3)*sin(theta2)*sin(theta5) - cos(theta2)*cos(theta3)*cos(theta4)*cos(theta5) + cos(theta4)*cos(theta5)*sin(theta2)*sin(theta3)) + (2*thetadot6*sin(theta6)*((cos(theta2)*sin(theta4)*sin(theta5))/5 + (2*sin(theta2)*sin(theta3)*sin(theta4))/5 - (2*cos(theta2)*cos(theta3)*sin(theta4))/5 + (2*cos(theta2)*cos(theta3)*cos(theta6)*sin(theta4))/5 + (2*cos(theta2)*cos(theta3)*sin(theta4)*sin(theta5))/5 - (2*cos(theta6)*sin(theta2)*sin(theta3)*sin(theta4))/5 + (2*cos(theta2)*sin(theta3)*sin(theta5)*sin(theta6))/5 + (2*cos(theta3)*sin(theta2)*sin(theta5)*sin(theta6))/5 - (2*sin(theta2)*sin(theta3)*sin(theta4)*sin(theta5))/5 - (2*cos(theta2)*cos(theta3)*cos(theta4)*cos(theta5)*sin(theta6))/5 + (2*cos(theta4)*cos(theta5)*sin(theta2)*sin(theta3)*sin(theta6))/5))/5 + (thetadot6*sin(theta6)*(cos(theta2)*cos(theta3)*cos(theta6)*sin(theta4) - cos(theta6)*sin(theta2)*sin(theta3)*sin(theta4) + cos(theta2)*sin(theta3)*sin(theta5)*sin(theta6) + cos(theta3)*sin(theta2)*sin(theta5)*sin(theta6) - cos(theta2)*cos(theta3)*cos(theta4)*cos(theta5)*sin(theta6) + cos(theta4)*cos(theta5)*sin(theta2)*sin(theta3)*sin(theta6)))/10 + (thetadot6*cos(theta6)*(cos(theta2)*cos(theta6)*sin(theta3)*sin(theta5) - cos(theta2)*cos(theta3)*sin(theta4)*sin(theta6) + cos(theta3)*cos(theta6)*sin(theta2)*sin(theta5) + sin(theta2)*sin(theta3)*sin(theta4)*sin(theta6) - cos(theta2)*cos(theta3)*cos(theta4)*cos(theta5)*cos(theta6) + cos(theta4)*cos(theta5)*cos(theta6)*sin(theta2)*sin(theta3)))/10) + (thetadot4*sin(theta4)*((2*cos(theta6))/5 + sin(theta5)/5 - 2/5) + (thetadot4*sin(theta4)*sin(theta5))/5 - (2*thetadot4*cos(theta4)*cos(theta5)*sin(theta6))/5)*((cos(theta2)*sin(theta4)*sin(theta5))/5 + (2*sin(theta2)*sin(theta3)*sin(theta4))/5 - (2*cos(theta2)*cos(theta3)*sin(theta4))/5 + (2*cos(theta2)*cos(theta3)*cos(theta6)*sin(theta4))/5 + (2*cos(theta2)*cos(theta3)*sin(theta4)*sin(theta5))/5 - (2*cos(theta6)*sin(theta2)*sin(theta3)*sin(theta4))/5 + (2*cos(theta2)*sin(theta3)*sin(theta5)*sin(theta6))/5 + (2*cos(theta3)*sin(theta2)*sin(theta5)*sin(theta6))/5 - (2*sin(theta2)*sin(theta3)*sin(theta4)*sin(theta5))/5 - (2*cos(theta2)*cos(theta3)*cos(theta4)*cos(theta5)*sin(theta6))/5 + (2*cos(theta4)*cos(theta5)*sin(theta2)*sin(theta3)*sin(theta6))/5) - (cos(theta4)*cos(theta6) + cos(theta5)*sin(theta4)*sin(theta6))*((thetadot6/10 + (sin(theta5)*(sin(theta4)*(thetadot2 + thetadot3) + thetadot1*cos(theta2 + theta3)*cos(theta4)))/10 + (cos(theta5)*(thetadot4 + thetadot1*sin(theta2 + theta3)))/10)*(cos(theta2)*cos(theta6)*sin(theta3)*sin(theta5) - cos(theta2)*cos(theta3)*sin(theta4)*sin(theta6) + cos(theta3)*cos(theta6)*sin(theta2)*sin(theta5) + sin(theta2)*sin(theta3)*sin(theta4)*sin(theta6) - cos(theta2)*cos(theta3)*cos(theta4)*cos(theta5)*cos(theta6) + cos(theta4)*cos(theta5)*cos(theta6)*sin(theta2)*sin(theta3)) - ((sin(theta6)*(thetadot5 + cos(theta4)*(thetadot2 + thetadot3) - thetadot1*cos(theta2 + theta3)*sin(theta4)))/10 - (cos(theta6)*(cos(theta5)*(sin(theta4)*(thetadot2 + thetadot3) + thetadot1*cos(theta2 + theta3)*cos(theta4)) - sin(theta5)*(thetadot4 + thetadot1*sin(theta2 + theta3))))/10)*(cos(theta2)*cos(theta5)*sin(theta3) + cos(theta3)*cos(theta5)*sin(theta2) + cos(theta2)*cos(theta3)*cos(theta4)*sin(theta5) - cos(theta4)*sin(theta2)*sin(theta3)*sin(theta5))) + (sin(theta3)*(cos(theta2 + theta3)*sin(theta4)*(cos(theta4)*(thetadot2/5 + thetadot3/5) - (thetadot1*cos(theta2 + theta3)*sin(theta4))/5 + (thetadot2*cos(theta3)*cos(theta4))/5 - (thetadot1*cos(theta2)*sin(theta4))/5) + thetadot5*sin(theta5)*((cos(theta2)*sin(theta4)*sin(theta5))/5 + (2*sin(theta2)*sin(theta3)*sin(theta4))/5 - (2*cos(theta2)*cos(theta3)*sin(theta4))/5 + (2*cos(theta2)*cos(theta3)*cos(theta6)*sin(theta4))/5 + (2*cos(theta2)*cos(theta3)*sin(theta4)*sin(theta5))/5 - (2*cos(theta6)*sin(theta2)*sin(theta3)*sin(theta4))/5 + (2*cos(theta2)*sin(theta3)*sin(theta5)*sin(theta6))/5 + (2*cos(theta3)*sin(theta2)*sin(theta5)*sin(theta6))/5 - (2*sin(theta2)*sin(theta3)*sin(theta4)*sin(theta5))/5 - (2*cos(theta2)*cos(theta3)*cos(theta4)*cos(theta5)*sin(theta6))/5 + (2*cos(theta4)*cos(theta5)*sin(theta2)*sin(theta3)*sin(theta6))/5) + (cos(theta4)*(sin(theta4)*(thetadot2 + thetadot3) + thetadot1*cos(theta2 + theta3)*cos(theta4))*(cos(theta2 + theta3) + cos(theta2)))/5 - (sin(theta4)*(cos(theta4)*(thetadot2 + thetadot3) - thetadot1*cos(theta2 + theta3)*sin(theta4))*(cos(theta2 + theta3) + cos(theta2)))/5 - cos(theta2 + theta3)*cos(theta4)*(sin(theta4)*(thetadot2/5 + thetadot3/5) + (thetadot1*cos(theta2 + theta3)*cos(theta4))/5 + (thetadot1*cos(theta2)*cos(theta4))/5 + (thetadot2*cos(theta3)*sin(theta4))/5) + thetadot5*cos(theta5)*cos(theta6)*((cos(theta2)*cos(theta5)*cos(theta6)*sin(theta4))/5 - (2*cos(theta2)*cos(theta3)*cos(theta4)*sin(theta6))/5 - (cos(theta2)*cos(theta4)*sin(theta6))/5 + (2*cos(theta2)*cos(theta5)*sin(theta3)*sin(theta6))/5 + (2*cos(theta3)*cos(theta5)*sin(theta2)*sin(theta6))/5 + (2*cos(theta4)*sin(theta2)*sin(theta3)*sin(theta6))/5 + (2*cos(theta2)*cos(theta3)*cos(theta5)*cos(theta6)*sin(theta4))/5 + (2*cos(theta2)*cos(theta3)*cos(theta4)*sin(theta5)*sin(theta6))/5 - (2*cos(theta5)*cos(theta6)*sin(theta2)*sin(theta3)*sin(theta4))/5 - (2*cos(theta4)*sin(theta2)*sin(theta3)*sin(theta5)*sin(theta6))/5) + (thetadot5*cos(theta5)^2*sin(theta4)*(2*cos(theta2 + theta3) + cos(theta2)))/5 + (thetadot5*sin(theta4)*sin(theta5)^2*(2*cos(theta2 + theta3) + cos(theta2)))/5 + thetadot5*cos(theta5)*sin(theta6)*((cos(theta2)*cos(theta4)*cos(theta6))/5 + (2*cos(theta2)*cos(theta5)*sin(theta3))/5 + (2*cos(theta3)*cos(theta5)*sin(theta2))/5 + (2*cos(theta2)*cos(theta3)*cos(theta4)*cos(theta6))/5 + (2*cos(theta2)*cos(theta3)*cos(theta4)*sin(theta5))/5 - (2*cos(theta2)*cos(theta5)*cos(theta6)*sin(theta3))/5 - (2*cos(theta3)*cos(theta5)*cos(theta6)*sin(theta2))/5 - (2*cos(theta4)*cos(theta6)*sin(theta2)*sin(theta3))/5 + (cos(theta2)*cos(theta5)*sin(theta4)*sin(theta6))/5 - (2*cos(theta4)*sin(theta2)*sin(theta3)*sin(theta5))/5 - (2*cos(theta2)*cos(theta3)*cos(theta4)*cos(theta6)*sin(theta5))/5 + (2*cos(theta2)*cos(theta3)*cos(theta5)*sin(theta4)*sin(theta6))/5 + (2*cos(theta4)*cos(theta6)*sin(theta2)*sin(theta3)*sin(theta5))/5 - (2*cos(theta5)*sin(theta2)*sin(theta3)*sin(theta4)*sin(theta6))/5)))/5 + ((sin(theta6)*(cos(theta5)*(sin(theta4)*(thetadot2 + thetadot3) + thetadot1*cos(theta2 + theta3)*cos(theta4)) - sin(theta5)*(thetadot4 + thetadot1*sin(theta2 + theta3))) + cos(theta6)*(thetadot5 + cos(theta4)*(thetadot2 + thetadot3) - thetadot1*cos(theta2 + theta3)*sin(theta4)))*((cos(theta2)*cos(theta5)*cos(theta6)*sin(theta4))/5 - (2*cos(theta2)*cos(theta3)*cos(theta4)*sin(theta6))/5 - (cos(theta2)*cos(theta4)*sin(theta6))/5 + (2*cos(theta2)*cos(theta5)*sin(theta3)*sin(theta6))/5 + (2*cos(theta3)*cos(theta5)*sin(theta2)*sin(theta6))/5 + (2*cos(theta4)*sin(theta2)*sin(theta3)*sin(theta6))/5 + (2*cos(theta2)*cos(theta3)*cos(theta5)*cos(theta6)*sin(theta4))/5 + (2*cos(theta2)*cos(theta3)*cos(theta4)*sin(theta5)*sin(theta6))/5 - (2*cos(theta5)*cos(theta6)*sin(theta2)*sin(theta3)*sin(theta4))/5 - (2*cos(theta4)*sin(theta2)*sin(theta3)*sin(theta5)*sin(theta6))/5) + (sin(theta6)*(thetadot5 + cos(theta4)*(thetadot2 + thetadot3) - thetadot1*cos(theta2 + theta3)*sin(theta4)) - cos(theta6)*(cos(theta5)*(sin(theta4)*(thetadot2 + thetadot3) + thetadot1*cos(theta2 + theta3)*cos(theta4)) - sin(theta5)*(thetadot4 + thetadot1*sin(theta2 + theta3))))*((cos(theta2)*cos(theta4)*cos(theta6))/5 + (2*cos(theta2)*cos(theta5)*sin(theta3))/5 + (2*cos(theta3)*cos(theta5)*sin(theta2))/5 + (2*cos(theta2)*cos(theta3)*cos(theta4)*cos(theta6))/5 + (2*cos(theta2)*cos(theta3)*cos(theta4)*sin(theta5))/5 - (2*cos(theta2)*cos(theta5)*cos(theta6)*sin(theta3))/5 - (2*cos(theta3)*cos(theta5)*cos(theta6)*sin(theta2))/5 - (2*cos(theta4)*cos(theta6)*sin(theta2)*sin(theta3))/5 + (cos(theta2)*cos(theta5)*sin(theta4)*sin(theta6))/5 - (2*cos(theta4)*sin(theta2)*sin(theta3)*sin(theta5))/5 - (2*cos(theta2)*cos(theta3)*cos(theta4)*cos(theta6)*sin(theta5))/5 + (2*cos(theta2)*cos(theta3)*cos(theta5)*sin(theta4)*sin(theta6))/5 + (2*cos(theta4)*cos(theta6)*sin(theta2)*sin(theta3)*sin(theta5))/5 - (2*cos(theta5)*sin(theta2)*sin(theta3)*sin(theta4)*sin(theta6))/5) - ((sin(theta6)*(2*thetadot2*sin(theta4) + 2*thetadot3*sin(theta4) + thetadot1*cos(theta2)*cos(theta4) + thetadot2*cos(theta3)*sin(theta4) + 2*thetadot1*cos(theta2)*cos(theta3)*cos(theta4) - 2*thetadot1*cos(theta4)*sin(theta2)*sin(theta3)))/5 + (cos(theta6)*(2*thetadot2*cos(theta4)*cos(theta5) + 2*thetadot3*cos(theta4)*cos(theta5) - thetadot2*sin(theta3)*sin(theta5) + thetadot2*cos(theta3)*cos(theta4)*cos(theta5) - thetadot1*cos(theta2)*cos(theta5)*sin(theta4) - 2*thetadot1*cos(theta2)*cos(theta3)*cos(theta5)*sin(theta4) + 2*thetadot1*cos(theta5)*sin(theta2)*sin(theta3)*sin(theta4)))/5 - (2*sin(theta6)*(sin(theta5)*(thetadot2*sin(theta4) + thetadot3*sin(theta4) + thetadot1*cos(theta2 + theta3)*cos(theta4)) + cos(theta5)*(thetadot4 + thetadot1*sin(theta2 + theta3))))/5)*(cos(theta2)*cos(theta3)*cos(theta6)*sin(theta4) - cos(theta6)*sin(theta2)*sin(theta3)*sin(theta4) + cos(theta2)*sin(theta3)*sin(theta5)*sin(theta6) + cos(theta3)*sin(theta2)*sin(theta5)*sin(theta6) - cos(theta2)*cos(theta3)*cos(theta4)*cos(theta5)*sin(theta6) + cos(theta4)*cos(theta5)*sin(theta2)*sin(theta3)*sin(theta6)) - ((2*thetadot6)/5 - (sin(theta5)*(thetadot2*sin(theta4) + thetadot3*sin(theta4) + thetadot1*cos(theta2 + theta3)*cos(theta4)) + cos(theta5)*(thetadot4 + thetadot1*sin(theta2 + theta3)))*((2*cos(theta6))/5 - 2/5) - (sin(theta6)*(2*thetadot2*cos(theta4)*cos(theta5) + 2*thetadot3*cos(theta4)*cos(theta5) - thetadot2*sin(theta3)*sin(theta5) + thetadot2*cos(theta3)*cos(theta4)*cos(theta5) - thetadot1*cos(theta2)*cos(theta5)*sin(theta4) - 2*thetadot1*cos(theta2)*cos(theta3)*cos(theta5)*sin(theta4) + 2*thetadot1*cos(theta5)*sin(theta2)*sin(theta3)*sin(theta4)))/5 + (cos(theta6)*(2*thetadot2*sin(theta4) + 2*thetadot3*sin(theta4) + thetadot1*cos(theta2)*cos(theta4) + thetadot2*cos(theta3)*sin(theta4) + 2*thetadot1*cos(theta2)*cos(theta3)*cos(theta4) - 2*thetadot1*cos(theta4)*sin(theta2)*sin(theta3)))/5)*(cos(theta2)*cos(theta6)*sin(theta3)*sin(theta5) - cos(theta2)*cos(theta3)*sin(theta4)*sin(theta6) + cos(theta3)*cos(theta6)*sin(theta2)*sin(theta5) + sin(theta2)*sin(theta3)*sin(theta4)*sin(theta6) - cos(theta2)*cos(theta3)*cos(theta4)*cos(theta5)*cos(theta6) + cos(theta4)*cos(theta5)*cos(theta6)*sin(theta2)*sin(theta3)))*((2*cos(theta4)*cos(theta6))/5 - (2*cos(theta4))/5 + (cos(theta5)*sin(theta3))/5 + (2*cos(theta4)*sin(theta5))/5 + (2*cos(theta5)*sin(theta4)*sin(theta6))/5 + (cos(theta3)*cos(theta4)*sin(theta5))/5) - ((thetadot6/10 + (sin(theta5)*(sin(theta4)*(thetadot2 + thetadot3) + thetadot1*cos(theta2 + theta3)*cos(theta4)))/10 + (cos(theta5)*(thetadot4 + thetadot1*sin(theta2 + theta3)))/10)*(cos(theta2)*cos(theta3)*cos(theta6)*sin(theta4) - cos(theta6)*sin(theta2)*sin(theta3)*sin(theta4) + cos(theta2)*sin(theta3)*sin(theta5)*sin(theta6) + cos(theta3)*sin(theta2)*sin(theta5)*sin(theta6) - cos(theta2)*cos(theta3)*cos(theta4)*cos(theta5)*sin(theta6) + cos(theta4)*cos(theta5)*sin(theta2)*sin(theta3)*sin(theta6)) + ((sin(theta6)*(cos(theta5)*(sin(theta4)*(thetadot2 + thetadot3) + thetadot1*cos(theta2 + theta3)*cos(theta4)) - sin(theta5)*(thetadot4 + thetadot1*sin(theta2 + theta3))))/10 + (cos(theta6)*(thetadot5 + cos(theta4)*(thetadot2 + thetadot3) - thetadot1*cos(theta2 + theta3)*sin(theta4)))/10)*(cos(theta2)*cos(theta5)*sin(theta3) + cos(theta3)*cos(theta5)*sin(theta2) + cos(theta2)*cos(theta3)*cos(theta4)*sin(theta5) - cos(theta4)*sin(theta2)*sin(theta3)*sin(theta5)))*(cos(theta4)*sin(theta6) - cos(theta5)*cos(theta6)*sin(theta4)) + ((thetadot6 + sin(theta5)*(sin(theta4)*(thetadot2 + thetadot3) + thetadot1*cos(theta2 + theta3)*cos(theta4)) + cos(theta5)*(thetadot4 + thetadot1*sin(theta2 + theta3)))*((cos(theta2)*cos(theta4)*cos(theta6))/5 + (2*cos(theta2)*cos(theta5)*sin(theta3))/5 + (2*cos(theta3)*cos(theta5)*sin(theta2))/5 + (2*cos(theta2)*cos(theta3)*cos(theta4)*cos(theta6))/5 + (2*cos(theta2)*cos(theta3)*cos(theta4)*sin(theta5))/5 - (2*cos(theta2)*cos(theta5)*cos(theta6)*sin(theta3))/5 - (2*cos(theta3)*cos(theta5)*cos(theta6)*sin(theta2))/5 - (2*cos(theta4)*cos(theta6)*sin(theta2)*sin(theta3))/5 + (cos(theta2)*cos(theta5)*sin(theta4)*sin(theta6))/5 - (2*cos(theta4)*sin(theta2)*sin(theta3)*sin(theta5))/5 - (2*cos(theta2)*cos(theta3)*cos(theta4)*cos(theta6)*sin(theta5))/5 + (2*cos(theta2)*cos(theta3)*cos(theta5)*sin(theta4)*sin(theta6))/5 + (2*cos(theta4)*cos(theta6)*sin(theta2)*sin(theta3)*sin(theta5))/5 - (2*cos(theta5)*sin(theta2)*sin(theta3)*sin(theta4)*sin(theta6))/5) - (cos(theta2)*cos(theta5)*sin(theta3) + cos(theta3)*cos(theta5)*sin(theta2) + cos(theta2)*cos(theta3)*cos(theta4)*sin(theta5) - cos(theta4)*sin(theta2)*sin(theta3)*sin(theta5))*((2*thetadot6)/5 - (sin(theta5)*(thetadot2*sin(theta4) + thetadot3*sin(theta4) + thetadot1*cos(theta2 + theta3)*cos(theta4)) + cos(theta5)*(thetadot4 + thetadot1*sin(theta2 + theta3)))*((2*cos(theta6))/5 - 2/5) - (sin(theta6)*(2*thetadot2*cos(theta4)*cos(theta5) + 2*thetadot3*cos(theta4)*cos(theta5) - thetadot2*sin(theta3)*sin(theta5) + thetadot2*cos(theta3)*cos(theta4)*cos(theta5) - thetadot1*cos(theta2)*cos(theta5)*sin(theta4) - 2*thetadot1*cos(theta2)*cos(theta3)*cos(theta5)*sin(theta4) + 2*thetadot1*cos(theta5)*sin(theta2)*sin(theta3)*sin(theta4)))/5 + (cos(theta6)*(2*thetadot2*sin(theta4) + 2*thetadot3*sin(theta4) + thetadot1*cos(theta2)*cos(theta4) + thetadot2*cos(theta3)*sin(theta4) + 2*thetadot1*cos(theta2)*cos(theta3)*cos(theta4) - 2*thetadot1*cos(theta4)*sin(theta2)*sin(theta3)))/5) - (sin(theta6)*(cos(theta5)*(sin(theta4)*(thetadot2 + thetadot3) + thetadot1*cos(theta2 + theta3)*cos(theta4)) - sin(theta5)*(thetadot4 + thetadot1*sin(theta2 + theta3))) + cos(theta6)*(thetadot5 + cos(theta4)*(thetadot2 + thetadot3) - thetadot1*cos(theta2 + theta3)*sin(theta4)))*((cos(theta2)*sin(theta4)*sin(theta5))/5 + (2*sin(theta2)*sin(theta3)*sin(theta4))/5 - (2*cos(theta2)*cos(theta3)*sin(theta4))/5 + (2*cos(theta2)*cos(theta3)*cos(theta6)*sin(theta4))/5 + (2*cos(theta2)*cos(theta3)*sin(theta4)*sin(theta5))/5 - (2*cos(theta6)*sin(theta2)*sin(theta3)*sin(theta4))/5 + (2*cos(theta2)*sin(theta3)*sin(theta5)*sin(theta6))/5 + (2*cos(theta3)*sin(theta2)*sin(theta5)*sin(theta6))/5 - (2*sin(theta2)*sin(theta3)*sin(theta4)*sin(theta5))/5 - (2*cos(theta2)*cos(theta3)*cos(theta4)*cos(theta5)*sin(theta6))/5 + (2*cos(theta4)*cos(theta5)*sin(theta2)*sin(theta3)*sin(theta6))/5) + ((sin(theta5)*(thetadot2*cos(theta4) + thetadot3*cos(theta4) - thetadot1*cos(theta2 + theta3)*sin(theta4)))/5 + sin(theta5)*((thetadot2*cos(theta4))/5 + (thetadot3*cos(theta4))/5 - (thetadot1*cos(theta2 + theta3)*sin(theta4))/5 + (thetadot2*cos(theta3)*cos(theta4))/5 - (thetadot1*cos(theta2)*sin(theta4))/5) + ((2*cos(theta6))/5 - 2/5)*(thetadot5 + thetadot2*cos(theta4) + thetadot3*cos(theta4) - thetadot1*cos(theta2 + theta3)*sin(theta4)) + (2*sin(theta6)*(cos(theta5)*(thetadot2*sin(theta4) + thetadot3*sin(theta4) + thetadot1*cos(theta2 + theta3)*cos(theta4)) - sin(theta5)*(thetadot4 + thetadot1*sin(theta2 + theta3))))/5 + (thetadot2*cos(theta5)*sin(theta3))/5)*(cos(theta2)*cos(theta3)*cos(theta6)*sin(theta4) - cos(theta6)*sin(theta2)*sin(theta3)*sin(theta4) + cos(theta2)*sin(theta3)*sin(theta5)*sin(theta6) + cos(theta3)*sin(theta2)*sin(theta5)*sin(theta6) - cos(theta2)*cos(theta3)*cos(theta4)*cos(theta5)*sin(theta6) + cos(theta4)*cos(theta5)*sin(theta2)*sin(theta3)*sin(theta6)))*((2*sin(theta4)*sin(theta6))/5 + (cos(theta3)*sin(theta4)*sin(theta6))/5 - (cos(theta6)*sin(theta3)*sin(theta5))/5 - (2*sin(theta4)*sin(theta5)*sin(theta6))/5 + (2*cos(theta4)*cos(theta5)*cos(theta6))/5 + (cos(theta3)*cos(theta4)*cos(theta5)*cos(theta6))/5) + ((thetadot3*sin(theta3)*(sin(theta4)*sin(theta6) + cos(theta4)*cos(theta5)*cos(theta6)))/5 + (thetadot3*cos(theta3)*cos(theta6)*sin(theta5))/5)*((cos(theta2)*cos(theta5)*cos(theta6)*sin(theta4))/5 - (2*cos(theta2)*cos(theta3)*cos(theta4)*sin(theta6))/5 - (cos(theta2)*cos(theta4)*sin(theta6))/5 + (2*cos(theta2)*cos(theta5)*sin(theta3)*sin(theta6))/5 + (2*cos(theta3)*cos(theta5)*sin(theta2)*sin(theta6))/5 + (2*cos(theta4)*sin(theta2)*sin(theta3)*sin(theta6))/5 + (2*cos(theta2)*cos(theta3)*cos(theta5)*cos(theta6)*sin(theta4))/5 + (2*cos(theta2)*cos(theta3)*cos(theta4)*sin(theta5)*sin(theta6))/5 - (2*cos(theta5)*cos(theta6)*sin(theta2)*sin(theta3)*sin(theta4))/5 - (2*cos(theta4)*sin(theta2)*sin(theta3)*sin(theta5)*sin(theta6))/5) + sin(theta4)*sin(theta5)*(((sin(theta6)*(cos(theta5)*(sin(theta4)*(thetadot2 + thetadot3) + thetadot1*cos(theta2 + theta3)*cos(theta4)) - sin(theta5)*(thetadot4 + thetadot1*sin(theta2 + theta3))))/10 + (cos(theta6)*(thetadot5 + cos(theta4)*(thetadot2 + thetadot3) - thetadot1*cos(theta2 + 